simulink model "abslut50_fixpt20_32"  (R2021b)
settings: Solver=VariableStepAuto  StartTime=0.0  StopTime=99  RelTol=1e-3
undefined symbols (not defined in the file or in its folder): figd2104, xcu250
libraries: hdlBasic x5226, vmcUtilities x1
(part 14 of 17)

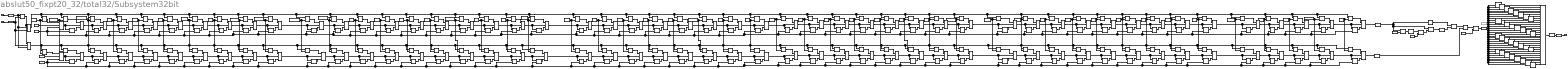
== system abslut50_fixpt20_32/total32/Subsystem32bit ==
  note: 50
  note: 40
  note: 30
  note: 20
  note: 10
  note: tiisai
  note: ooki
  note: 1275no11bit
  note: tmp_2
  note: tmp_3
  note: truthtable_out_x
  note: truthtable_out_y
  In3 : Inport
  In4 : Inport  Port=2
  CMult1 : hdlBasic/CMult  const=50  gui_display_data_type=Fixed-point  const_n_bits=6  const_bin_pt=0  float_type=Single  exp_bits=8  fraction_bits=24  en=off  latency=0  precision=Full  arith_type="Signed  (2's comp)"  n_bits=16  bin_pt=14  quantization=Truncate  overflow=Wrap  use_behavioral_HDL=off  mem_type=Distributed RAM  pipeline=off  XmcBlockStatus=1  maskContainerNames=tabcontainer1  block_type=cmult  block_config=sysgen:CMult_config
      settings: infoedit=[]
  Concat : hdlBasic/Concat  num_inputs=32  XmcBlockStatus=1  maskContainerNames=group1  block_type=concat  block_config=sysgen:Concat_config
  Constant : hdlBasic/Constant  const=1.0  gui_display_data_type=Fixed-point  arith_type=Unsigned  n_bits=1  bin_pt=0  preci_type=Single  exp_width=8  frac_width=24  explicit_period=on  period=1  XmcBlockStatus=1  maskContainerNames=tabcontainer1  block_type=constant  block_config=sysgen:Constant_config
  Constant1 : hdlBasic/Constant  const=0  gui_display_data_type=Fixed-point  arith_type=Unsigned  n_bits=6  bin_pt=0  preci_type=Single  exp_width=8  frac_width=24  explicit_period=on  period=1  XmcBlockStatus=1  maskContainerNames=tabcontainer1  block_type=constant  block_config=sysgen:Constant_config
  Constant2 : hdlBasic/Constant  const=1  gui_display_data_type=Fixed-point  arith_type=Unsigned  n_bits=6  bin_pt=0  preci_type=Single  exp_width=8  frac_width=24  explicit_period=on  period=1  XmcBlockStatus=1  maskContainerNames=tabcontainer1  block_type=constant  block_config=sysgen:Constant_config
  Constant3 : hdlBasic/Constant  const=98  gui_display_data_type=Fixed-point  arith_type=Unsigned  n_bits=7  bin_pt=0  preci_type=Single  exp_width=8  frac_width=24  explicit_period=on  period=1  XmcBlockStatus=1  maskContainerNames=tabcontainer1  block_type=constant  block_config=sysgen:Constant_config
  Constant5 : hdlBasic/Constant  const=1.0  gui_display_data_type=Fixed-point  arith_type=Unsigned  n_bits=10  bin_pt=0  preci_type=Single  exp_width=8  frac_width=24  explicit_period=on  period=1  XmcBlockStatus=1  maskContainerNames=tabcontainer1  block_type=constant  block_config=sysgen:Constant_config
  Constant6 : hdlBasic/Constant  const=0  gui_display_data_type=Fixed-point  arith_type=Unsigned  n_bits=6  bin_pt=0  preci_type=Single  exp_width=8  frac_width=24  explicit_period=on  period=1  XmcBlockStatus=1  maskContainerNames=tabcontainer1  block_type=constant  block_config=sysgen:Constant_config
  Constant7 : hdlBasic/Constant  const=1  gui_display_data_type=Fixed-point  arith_type=Unsigned  n_bits=6  bin_pt=0  preci_type=Single  exp_width=8  frac_width=24  explicit_period=on  period=1  XmcBlockStatus=1  maskContainerNames=tabcontainer1  block_type=constant  block_config=sysgen:Constant_config
  Convert23 : hdlBasic/Convert  Commented=on  gui_display_data_type=Fixed-point  arith_type=Unsigned  n_bits=11  bin_pt=0  float_type=Single  exp_bits=8  fraction_bits=24  quantization="Round  (unbiased: +/- Inf)"  overflow=Saturate  en=off  latency=1  pipeline=off  XmcBlockStatus=1  maskContainerNames=group2  block_type=convert  block_config=sysgen:Convert_config
  Gate_In1 : hdlBasic/Gateway In  gui_display_data_type=Fixed-point  arith_type=Signed (2's comp)  n_bits=32  bin_pt=30  preci_type=Double  exp_width=8  frac_width=24  rows=1  columns=1  quantization="Round  (unbiased: +/- Inf)"  overflow=Saturate  period=1  UseAsADC=off  ADCChannel='1'  interface=None  automatic_assignment=on  address_offset=hex2dec('00')  intf_name=''  intf_description=''  default_value=0  timing_constraint=None  locs_specified=off  LOCs={}  io_standard={}  inherit_from_input=off  hdl_port=on  XmcBlockStatus=1  maskContainerNames=group4  block_type=gatewayin  block_config=sysgen:gateway_in_config  block_width_w=590  block_height_w=620  block_width=640  block_height=850
  Gate_In2 : hdlBasic/Gateway In  gui_display_data_type=Fixed-point  arith_type=Signed (2's comp)  n_bits=32  bin_pt=30  preci_type=Double  exp_width=8  frac_width=24  rows=1  columns=1  quantization="Round  (unbiased: +/- Inf)"  overflow=Saturate  period=1  UseAsADC=off  ADCChannel='1'  interface=None  automatic_assignment=on  address_offset=hex2dec('00')  intf_name=''  intf_description=''  default_value=0  timing_constraint=None  locs_specified=off  LOCs={}  io_standard={}  inherit_from_input=off  hdl_port=on  XmcBlockStatus=1  maskContainerNames=group4  block_type=gatewayin  block_config=sysgen:gateway_in_config  block_width_w=590  block_height_w=620  block_width=640  block_height=850
  Gate_out1 : hdlBasic/Gateway Out  inherit_from_input=off  hdl_port=on  rows=1  columns=1  UseAsDAC=off  DACChannel='1'  interface=None  automatic_assignment=on  address_offset=hex2dec('00')  intf_name=''  intf_description=''  timing_constraint=None  locs_specified=off  LOCs={}  io_standard={}  XmcBlockStatus=1  maskContainerNames=group4  block_type=gatewayout  block_config=sysgen:gateway_out_config  block_width_w=590  block_height_w=620  block_width=620  block_height=750
  Negate : hdlBasic/Negate  precision=Full  arith_type=Unsigned  n_bits=16  bin_pt=14  quantization=Truncate  overflow=Wrap  en=off  latency=0  XmcBlockStatus=1  maskContainerNames=tabcontainer1  block_type=negate  block_config=sysgen:Negate_config
  ROM1 : hdlBasic/ROM  depth=1275  initVector=[1,1,1,1,1,1,1,1,1,1,1,1,1,1,1,1,1,1,1,1,1,1,1,1,1,1,1,1,1,1,1,1,1,1,1,1,1,1,1,1,1,1,1,0,0,1,1,1,1,1,1,0,0,0,0,1,1,1,1,1,0,0,0,0,0,0,1,1,1,1,1,0,0,0,0,0,0,0,1,1,1,1,0,0,0,0,0,0,0,0,0,1,1,1,0,0,0,0,0,0,0,0,0,0,0,1,1,1,0,0,0,0,0,0,0,0,0,0,0,0,1,1,0,0,0,0,0,0,0,0,0,0,0,0,0,0,1,1,0,0,0,0,0,0,0,0,0,0,0,0,0,0,0,1,1,0,0,0,0,0,0,0,0,0,0,0,0,0,0,0,0,1,0,0,0,0,0,0,0,0,0,0,0,0,0,0,0,0,0,0,1,0,0,0,0,0,0,0,0,0,0,0,0,0,0,0,0,0,0,0,1,0,0,0,0,0,0,0,0,0,0,0,0,0,0,0,0,0,0,0,0,1,0,0,0,0,0,0,0,0,0,0,0,0,0,0,0,0,0,0,0,0,0,1,0,0,0,0,0,0,0,0,0,0,0,0,0,0,0,0,0,0,0,0,0,0,1,0,0,0,0,0,0,0,0,0,0,0,0,0,0,0,0,0,0,0,0,0,0,0,1,0,0,0,0,0,0,0,0,0,0,0,0,0,0,0,0,0,0,0,0,0,0,0,0,1,0,0,0,0,0,0,0,0,0,0,0,0,0,0,0,0,0,0,0,0,0,0,0,0,0,1,0,0,0,0,0,0,0,0,0,0,0,0,0,0,0,0,0,0,0,0,0,0,0,0,0,0,1,0,0,0,0,0,0,0,0,0,0,0,0,0,0,0,0,0,0,0,0,0,0,0,0,0,0,0,1,0,0,0,0,0,0,0,0,0,0,0,0,0,0,0,0,0,0,0,0,0,0,0,0,0,0,0,0,1,0,0,0,0,0,0,0,0,0,0,0,0,0,0,0,0,0,0,0,0,0,0,0,0,0,0,0,0,0,1,0,0,0,0,0,0,0,0,0,0,0,0,0,0,0,0,0,0,0,0,0,0,0,0,0,0,0,0,0,0,1,0,0,0,0,0,0,0,0,0,0,0,0,0,0,0,0,0,0,0,0,0,0,0,0,0,0,0,0,0,0,0,1,1,0,0,0,0,0,0,0,0,0,0,0,0,0,0,0,0,0,0,0,0,0,0,0,0,0,0,0,0,0,0,0,1,1,0,0,0,0,0,0,0,0,0,0,0,0,0,0,0,0,0,0,0,0,0,0,0,0,0,0,0,0,0,0,0,0,1,1,0,0,0,0,0,0,0,0,0,0,0,0,0,0,0,0,0,0,0,0,0,0,0,0,0,0,0,0,0,0,0,0,0,1,1,1,0,0,0,0,0,0,0,0,0,0,0,0,0,0,0,0,0,0,0,0,0,0,0,0,0,0,0,0,0,0,0,0,0,1,1,1,0,0,0,0,0,0,0,0,0,0,0,0,0,0,0,0,0,0,0,0,0,0,0,0,0,0,0,0,0,0,0,0,0,0,1,1,1,1,0,0,0,0,0,0,0,0,0,0,0,0,0,0,0,0,0,0,0,0,0,0,0,0,0,0,0,0,0,0,0,0,0,0,1,1,1,1,1,0,0,0,0,0,0,0,0,0,0,0,0,0,0,0,0,0,0,0,0,0,0,0,0,0,0,0,0,0,0,0,0,0,0,1,1,1,1,1,0,0,0,0,0,0,0,0,0,0,0,0,0,0,0,0,0,0,0,0,0,0,0,0,0,0,0,0,0,0,0,0,0,0,0,1,1,1,1,1,1,0,0,0,0,0,0,0,0,0,0,0,0,0,0,0,0,0,0,0,0,0,0,0,0,0,0,0,0,0,0,0,0,0,0,0,1,1,1,1,1,1,1,0,0,0,0,0,0,0,0,0,0,0,0,0,0,0,0,0,0,0,0,0,0,0,0,0,0,0,0,0,0,0,0,0,0,0,1,1,1,1,1,1,1,1,0,0,0,0,0,0,0,0,0,0,0,0,0,0,0,0,0,0,0,0,0,0,0,0,0,0,0,0,0,0,0,0,0,0,1,1,1,1,1,1,1,1,1,1,0,0,0,0,0,0,0,0,0,0,0,0,0,0,0,0,0,0,0,0,0,0,0,0,0,0,0,0,0,0,0,0,1,1,1,1,1,1,1,1,1,1,1,1,1,0,0,0,0,0,0,0,0,0,0,0,0,0,0,0,0,0,0,0,0,0,0,0,0,0,0,0,0,0,0,1,1,1,1,1,1,1,1,1,1,1,1,1,1,1,1,1,0,0,0,0,0,0,0,0,0,0,0,0,0,0,0,0,0,0,0,0,0,0,0,0,0,0,1,1,1,1,1,1,1,1,1,1,1,1,1,1,1,1,1,1,1,1,1,0,0,0,0,0,0,0,0,0,0,0,0,0,0,0,0,0,0,0,0,0,0,0,0,1,1,1,1,1,1,1,1,1,1,1,1,1,1,1,1,1,1,1,1,1,1,1,1,1,0,0,0,0,0,0,0,0,0,0,0,0,0,0,0,0,0,0,0,0,1,1,1,1,1,1,1,1,1,1,1,1,1,1,1,1,1,1,1,1,1,1,1,1,1,1,1,1,1,1,1,0,0,0,0,0,0,0,0,0,0,0,0,0,0,1,1,1,1,1,1,1,1,1,1,1,1,1,1,1,1,1,1,1,1,1,1,1,1,1,1,1,1,1,1,1,1,1,1,1,1,1,1,1,1,1,1,1,1,1,1,1,1,1,1,1,1,1,1,1,1,1,1,1,1,1,1,1,1,1,1,1]  distributed_mem=Distributed memory  rst=off  init_reg=0  en=off  latency=0  gui_display_data_type=Boolean  arith_type=Boolean  n_bits=2  bin_pt=0  preci_type=Double  exp_width=8  frac_width=24  optimize=Area  use_rpm=on  simulation_type=fast_sim  XmcBlockStatus=1  maskContainerNames=tabcontainer1  block_type=sprom  block_config=sysgen:SPROM_config
  ROM10 : hdlBasic/ROM  depth=1275  initVector=[0,1,0,1,1,0,1,1,0,1,1,1,0,0,1,0,0,0,0,1,0,1,1,0,0,1,1,0,1,0,1,1,1,1,0,1,1,0,1,0,1,1,0,0,1,1,0,0,1,1,0,0,0,1,0,0,1,1,1,0,1,1,0,1,1,0,0,0,0,0,0,1,0,1,1,1,0,0,0,0,1,1,1,0,0,1,0,0,0,0,1,1,0,0,1,1,1,1,1,0,1,0,0,0,1,1,1,0,0,1,0,0,0,0,1,0,1,1,1,0,1,1,0,1,0,1,0,0,1,1,0,0,0,1,1,0,1,0,0,1,1,0,1,0,1,1,1,1,1,0,0,0,1,1,1,1,1,0,0,1,1,0,1,1,0,0,0,1,0,0,1,1,1,1,1,1,1,1,0,0,1,0,1,0,0,0,0,1,1,0,0,0,0,1,1,1,1,1,1,1,0,0,1,0,1,1,1,0,1,0,0,0,1,1,0,0,1,1,1,1,1,1,1,0,0,1,0,0,1,0,0,1,0,1,1,0,0,1,0,0,0,1,1,1,1,1,1,0,0,0,0,1,1,0,1,1,0,1,0,0,1,0,0,1,0,0,1,1,1,1,1,1,0,1,1,1,0,0,1,0,1,0,1,1,0,1,0,1,1,0,1,0,0,1,1,1,1,1,0,0,0,1,0,1,0,1,0,1,0,0,1,0,1,0,1,0,1,1,0,1,0,1,1,1,0,0,1,0,1,0,1,0,1,0,0,1,0,1,0,1,0,1,1,0,1,0,1,1,1,0,0,0,0,1,0,1,0,1,1,0,1,0,1,1,0,1,0,0,1,1,1,1,1,0,0,1,1,0,0,1,1,0,1,0,0,1,0,0,1,0,0,1,1,1,1,1,1,0,1,1,1,0,1,1,0,1,1,0,1,1,0,0,1,0,0,0,1,1,1,1,1,1,0,0,0,0,1,1,1,1,1,1,1,1,1,0,0,1,1,0,0,1,1,1,1,1,1,1,0,0,1,0,0,1,0,0,1,1,1,0,0,1,1,1,0,0,0,0,1,1,1,1,1,1,1,0,0,1,0,1,1,1,0,1,0,0,0,0,1,1,1,1,0,0,0,0,1,1,1,1,1,1,1,0,0,1,0,1,0,0,0,0,1,1,0,1,1,0,1,1,0,0,1,1,0,1,1,0,1,1,1,1,0,0,1,1,0,1,1,0,0,0,1,0,0,1,1,0,0,0,1,1,1,1,1,1,0,0,0,1,1,1,0,0,1,1,0,1,0,1,1,1,1,1,0,0,0,1,0,1,1,0,0,1,0,1,1,0,1,0,0,1,1,0,1,1,1,0,1,0,1,0,0,1,1,0,0,0,1,1,0,0,0,0,1,1,1,1,0,0,0,0,1,1,1,1,0,0,0,0,1,1,0,0,1,0,0,0,0,1,0,1,1,1,0,1,0,1,0,1,0,1,1,1,1,1,1,1,1,0,1,0,1,0,1,0,1,0,0,1,1,1,1,1,0,1,0,0,0,1,1,1,0,0,0,0,0,1,1,0,0,0,0,1,1,0,0,0,0,0,1,1,1,0,0,1,1,1,0,0,1,0,0,0,0,1,0,1,0,1,0,0,1,1,1,0,1,1,1,1,0,1,1,1,0,0,1,0,1,0,1,0,0,0,0,0,1,0,1,1,1,0,0,0,0,1,0,1,0,1,0,1,1,0,1,0,0,1,0,1,1,0,1,0,1,0,1,0,0,0,0,1,1,1,0,1,1,0,1,1,0,0,0,0,0,0,1,1,0,0,1,1,1,0,1,1,0,1,1,1,0,0,1,1,0,0,0,0,0,0,1,0,0,1,1,0,0,0,1,0,1,1,0,1,1,1,1,1,1,1,1,0,0,1,0,0,1,0,0,1,1,1,1,1,1,1,1,0,1,1,0,1,0,1,0,1,1,0,0,1,1,1,1,0,0,0,1,1,0,0,1,1,0,0,0,0,0,0,0,0,1,1,0,0,1,1,0,0,0,1,1,1,1,1,0,1,1,1,1,0,1,0,0,0,1,1,1,0,0,0,1,0,1,1,0,1,1,1,1,1,1,0,1,1,0,1,0,0,0,1,1,1,0,0,0,1,1,1,0,0,1,1,0,0,0,0,1,0,0,1,0,0,1,1,1,1,1,1,0,1,0,0,1,0,1,1,1,1,1,1,0,0,1,0,0,1,0,0,0,0,0,0,0,0,1,0,1,1,1,0,1,1,0,1,0,1,0,0,1,1,0,0,0,0,1,1,0,0,0,0,1,1,0,0,1,0,1,0,1,1,0,1,1,1,0,1,1,0,0,1,1,1,1,1,1,0,0,1,1,1,0,1,0,1,1,0,0,1,1,0,0,1,1,0,0,1,1,0,1,0,1,1,1,0,0,1,1,1,1,1,1,1,1,0,1,0,0,0,1,0,1,1,0,1,1,0,1,1,1,1,1,1,1,0,0,1,1,0,0,1,1,1,1,1,1,1,0,1,1,0,1,1,0,1,0,0,0,1,1,1,0,0,0,0,0,1,1,0,1,0,1,0,0,0,0,1,1,0,1,1,1,1,0,0,1,1,1,1,0,1,1,0,0,0,0,1,0,1,0,1,1,0,0,0,0,0,1,0,1,1,1,0,1,0,0,0,1,0,0,0,1,1,0,1,1,0,0,0,1,0,1,1,0,1,0,0,0,1,1,0,1,1,0,0,0,1,0,0,0,1,0,1,1,1,0,0,1,1,1,1,0,1,1,1,1,0,0,0,1,1,1,1,1,1,0,0,1,0,0,0,0,0,0,1,0,0,1,1,1,1,1,1,0,0,0,1,1,1,1,0,1,1,1,1,0]  distributed_mem=Distributed memory  rst=off  init_reg=0  en=off  latency=0  gui_display_data_type=Boolean  arith_type=Boolean  n_bits=2  bin_pt=0  preci_type=Double  exp_width=8  frac_width=24  optimize=Area  use_rpm=on  simulation_type=fast_sim  XmcBlockStatus=1  maskContainerNames=tabcontainer1  block_type=sprom  block_config=sysgen:SPROM_config
  ROM11 : hdlBasic/ROM  depth=1275  initVector=[0,0,1,0,1,1,0,1,0,0,1,1,0,1,1,0,0,0,1,0,0,1,0,1,1,0,1,1,0,0,1,0,0,1,0,0,0,0,0,0,1,1,0,1,1,1,0,1,1,0,1,0,1,0,0,1,0,0,1,1,1,0,1,0,1,1,1,0,0,1,1,1,1,1,1,1,0,1,1,0,1,1,1,0,1,0,1,0,0,0,0,1,1,0,1,0,0,0,1,0,0,1,1,1,1,0,1,1,0,0,1,1,0,1,0,0,0,0,0,0,0,1,0,0,0,0,1,0,1,1,0,1,0,1,1,1,1,0,1,0,1,1,0,1,1,0,0,0,1,1,0,0,0,0,1,1,1,0,1,0,1,1,1,0,1,1,1,1,1,1,1,1,1,0,0,0,1,1,0,1,0,0,0,0,0,0,1,1,0,0,1,0,0,1,1,0,0,0,0,1,0,1,0,0,1,0,1,0,1,1,1,0,1,0,1,0,1,1,0,0,0,0,1,0,1,1,1,1,0,1,1,0,1,1,0,1,0,0,1,0,0,1,0,0,0,0,1,0,1,0,0,0,0,1,1,0,0,1,1,0,0,1,0,0,1,0,1,1,0,0,0,1,0,1,1,1,1,0,0,0,1,1,1,0,0,0,1,1,0,0,1,1,0,1,0,0,0,1,1,0,0,0,0,0,1,1,1,1,1,0,0,0,0,1,1,1,1,0,0,0,1,1,0,0,1,0,0,0,0,1,1,1,1,1,0,0,0,0,1,1,1,1,0,0,0,1,1,0,0,1,1,1,0,0,0,1,1,1,0,0,0,1,1,0,0,1,1,0,1,0,0,0,1,1,0,0,0,0,1,1,0,0,1,1,0,0,1,0,0,1,0,1,1,0,0,0,1,0,1,1,1,1,0,0,1,1,0,1,1,0,1,0,0,1,0,0,1,0,0,0,0,1,0,1,0,0,0,0,1,1,1,1,1,1,0,1,0,1,0,1,0,1,1,0,0,0,0,1,0,1,1,1,1,0,1,1,0,1,0,1,1,0,1,0,1,1,0,0,1,1,0,0,0,0,1,0,1,0,0,1,0,1,0,1,1,1,0,0,0,0,0,0,0,0,1,1,1,1,0,0,0,1,1,0,1,0,0,0,0,0,0,1,1,0,0,1,0,0,1,0,0,0,0,1,0,0,1,0,0,1,1,1,0,1,0,1,1,1,0,1,1,1,1,1,1,1,0,0,1,1,0,1,0,0,1,0,1,1,0,0,1,1,0,1,0,1,1,0,1,1,0,0,0,1,1,0,0,0,1,1,1,1,0,0,0,1,1,0,0,0,1,1,1,1,0,0,1,0,0,0,0,1,0,1,1,0,1,0,1,1,1,0,1,1,0,1,1,0,1,1,1,1,0,1,1,0,1,1,0,1,0,1,1,0,0,1,1,0,1,0,0,0,0,0,0,1,0,1,0,1,1,0,1,1,1,1,1,1,0,1,1,0,1,0,1,0,1,1,0,1,0,0,0,1,0,0,1,1,1,1,0,1,1,1,0,0,0,0,1,0,1,1,0,1,0,0,0,0,1,1,1,0,1,1,0,1,1,1,0,1,0,1,0,0,0,0,1,0,0,1,1,0,0,1,0,0,0,0,0,0,0,0,1,0,0,1,1,0,0,1,0,1,0,0,1,1,1,1,1,1,1,0,1,0,1,0,1,0,1,0,1,0,0,1,1,0,0,1,1,0,0,1,0,1,0,1,0,1,0,1,1,0,0,1,1,1,0,1,0,1,1,0,0,1,0,0,0,0,0,0,0,1,0,1,0,0,1,0,1,0,0,0,0,0,0,0,1,0,0,1,1,0,1,1,0,1,0,1,0,0,1,1,0,0,0,1,0,1,0,1,0,0,0,0,0,0,0,0,0,0,1,0,1,0,1,0,0,0,1,1,0,0,0,0,0,1,1,0,1,1,0,0,1,1,0,1,1,1,1,1,0,0,0,1,0,1,1,0,1,0,0,0,1,1,1,1,1,0,1,1,0,0,1,0,0,1,0,0,1,0,0,1,1,1,1,0,1,0,0,1,1,0,0,1,1,0,0,1,1,0,0,1,1,0,0,1,1,0,0,1,0,1,1,1,1,0,1,0,1,1,0,1,1,0,0,0,0,1,1,0,1,1,0,0,1,0,1,0,0,1,1,1,1,0,0,1,0,1,0,0,1,1,0,1,1,0,0,0,0,1,0,0,0,1,0,0,1,1,1,1,1,1,0,0,1,0,1,1,1,0,0,0,1,1,1,1,1,1,0,0,0,1,1,1,0,1,0,0,1,1,1,1,1,1,0,1,1,0,1,1,0,0,0,1,0,1,1,1,0,0,0,1,0,0,1,1,1,1,1,1,1,1,1,1,1,1,0,0,1,0,0,0,1,1,1,0,1,0,0,0,1,0,1,0,0,1,1,1,0,0,1,1,1,1,1,0,0,0,1,0,1,0,0,0,0,0,0,0,0,0,0,1,0,1,0,0,0,1,1,1,1,1,0,0,1,1,1,0,0,1,1,0,0,0,1,1,0,1,0,0,1,0,1,0,1,1,0,0,1,1,0,0,0,0,0,0,1,1,0,0,1,1,0,1,0,1,0,0,1,0,1,1,0,0,0,1,0,1,1,1,1,0,0,0,0,0,0,0,0,1,1,1,0,1,1,0,0,1,1,0,0,0,0,1,1,0,0,1,1,0,1,1,1,0,0,0,0,0,0,0,0,1,1,1,1,0,0,0,0,1,0,1,0,0,1,1,1,1,1,0,0,1,0,1,1,1,0,1,1,0,0,1,1,0,1,1,1,0,1,0,0,1,1,1,1,1,0,0,1,0,1,0,0,0,0]  distributed_mem=Distributed memory  rst=off  init_reg=0  en=off  latency=0  gui_display_data_type=Boolean  arith_type=Boolean  n_bits=2  bin_pt=0  preci_type=Double  exp_width=8  frac_width=24  optimize=Area  use_rpm=on  simulation_type=fast_sim  XmcBlockStatus=1  maskContainerNames=tabcontainer1  block_type=sprom  block_config=sysgen:SPROM_config
  ROM12 : hdlBasic/ROM  depth=1275  initVector=[0,1,0,0,1,1,0,0,1,1,0,0,0,1,1,1,0,0,0,1,1,0,0,0,0,0,0,1,0,1,0,1,1,0,0,0,1,0,0,1,1,1,0,0,0,1,1,1,1,0,0,1,0,0,0,1,0,1,1,0,1,0,1,0,0,0,0,1,1,0,1,0,0,1,0,0,0,1,1,1,1,0,1,0,0,1,0,0,0,1,1,0,1,0,0,0,0,0,0,1,1,1,0,1,1,0,1,1,0,1,1,0,1,0,0,0,1,0,1,1,0,0,1,0,0,1,0,0,1,1,1,1,0,0,1,1,1,0,0,0,1,0,1,0,1,1,0,1,1,1,1,1,0,1,0,0,1,0,0,0,1,1,1,0,0,0,1,0,1,1,0,0,0,1,1,1,0,1,0,0,0,0,0,1,0,0,0,0,1,0,0,1,0,1,0,1,1,1,1,0,0,0,1,1,0,1,0,1,1,0,0,0,0,0,0,0,1,0,1,1,1,1,0,0,0,0,1,1,0,0,1,0,0,1,0,0,0,1,1,1,0,0,1,1,0,1,0,0,1,1,0,0,1,0,1,0,1,0,1,0,1,1,0,1,1,1,1,0,1,0,0,0,1,0,1,1,1,0,0,1,0,0,1,0,0,1,0,1,0,1,0,1,1,1,1,0,0,0,1,1,0,0,1,1,0,0,1,1,1,0,0,1,1,0,0,1,1,0,0,1,0,1,1,0,1,0,0,1,1,0,0,1,1,1,0,0,1,1,0,0,1,1,0,0,1,0,1,1,0,1,1,1,0,0,1,0,0,1,0,0,1,0,1,0,1,0,1,1,1,1,0,0,0,1,1,0,0,1,0,1,0,1,0,1,0,1,1,0,1,1,1,1,0,1,0,0,0,1,0,1,1,1,1,1,1,1,0,0,1,0,0,0,1,1,1,0,0,1,1,0,1,0,0,1,1,0,0,1,1,0,1,1,0,1,1,0,0,0,0,0,0,1,0,1,1,1,1,0,0,0,0,1,1,0,0,1,0,0,0,0,0,0,0,0,1,0,1,0,1,0,1,1,1,1,0,0,0,1,1,0,1,0,1,1,0,0,0,1,0,1,1,0,1,0,0,0,0,0,1,1,1,0,1,0,0,0,0,0,1,0,0,0,0,1,0,1,0,1,0,1,0,0,1,0,1,0,1,0,1,0,0,1,0,0,0,1,1,1,0,0,0,1,0,1,1,0,1,1,1,1,0,1,0,0,1,0,1,1,1,1,0,1,0,0,0,1,0,1,0,1,1,0,1,1,1,1,1,0,1,0,0,1,0,0,1,1,1,1,0,0,1,0,0,1,0,0,0,1,0,0,1,0,0,1,1,1,1,0,0,1,1,1,1,0,1,0,0,1,1,1,1,1,1,0,0,1,0,1,1,1,0,1,1,0,1,1,0,1,0,0,0,1,0,1,1,1,1,0,0,0,0,1,0,0,0,0,0,0,1,0,0,0,0,1,1,1,0,1,0,0,0,0,0,0,1,1,1,0,1,1,1,0,1,1,0,1,0,0,1,1,0,0,1,1,0,0,1,0,1,1,0,1,1,1,1,1,0,1,0,0,1,0,0,0,1,1,1,0,0,1,0,1,1,0,1,1,0,1,1,0,1,1,0,1,1,0,1,0,0,1,1,0,1,1,0,1,0,0,1,0,0,0,1,1,0,1,1,1,0,0,0,1,1,1,1,1,1,1,1,1,1,0,0,0,1,1,1,0,1,1,1,0,1,1,0,1,0,1,0,0,0,0,0,1,0,1,0,0,0,0,1,0,1,0,0,0,0,1,0,1,0,0,0,0,1,0,1,0,0,0,1,1,1,1,0,0,1,0,0,0,0,0,0,1,0,1,1,1,0,0,1,0,0,1,0,0,1,0,0,1,0,0,1,1,1,0,1,0,0,0,0,1,0,0,1,1,1,0,0,0,0,0,0,0,1,0,1,1,1,0,1,1,1,1,0,1,1,0,1,1,1,1,0,1,1,1,0,1,0,0,0,0,0,0,1,0,1,1,0,0,0,0,0,1,1,1,0,1,0,0,1,0,1,0,1,1,0,1,1,0,1,1,0,1,0,1,0,0,1,0,1,1,1,0,0,0,0,0,0,0,0,0,1,0,0,1,0,0,0,0,0,0,1,0,1,1,1,1,0,1,1,1,1,0,1,1,1,1,0,1,0,0,0,0,0,0,1,0,0,1,1,0,0,0,1,1,0,0,1,0,1,0,0,0,1,1,0,0,0,1,0,0,1,0,0,0,0,1,0,0,1,0,0,0,1,1,0,0,0,1,0,1,0,0,1,0,0,0,1,1,1,0,1,1,0,0,1,1,0,1,0,1,0,1,0,0,0,0,0,0,0,0,0,0,0,0,1,0,1,0,1,0,1,1,0,0,1,1,0,1,1,0,0,1,1,1,0,0,1,1,1,1,0,0,0,0,0,0,1,1,1,0,0,1,1,1,1,1,1,0,0,1,1,1,0,0,0,0,0,0,1,1,1,1,0,0,1,1,0,1,1,1,0,0,0,0,0,1,1,1,1,0,1,1,0,0,1,0,0,1,0,0,1,1,0,0,1,0,0,1,0,0,1,1,0,1,1,1,1,0,0,0,0,0,1,1,1,0,1,0,0,0,0,1,0,1,0,1,1,1,1,0,0,0,0,1,0,0,1,0,0,0,0,1,0,0,1,0,0,0,0,1,1,1,1,0,1,0,1,0,0,0,0,1,0,0,1,0,0,0,1,0,0,1,1,1,0,1,0,0,0,1,1,0,0,0,0,0,1,0,0,1,0,0,0,0,0,1,1,0,0,0,1,0,1,1,1,0,0,1,0,0,0,1,0]  distributed_mem=Distributed memory  rst=off  init_reg=0  en=off  latency=0  gui_display_data_type=Boolean  arith_type=Boolean  n_bits=2  bin_pt=0  preci_type=Double  exp_width=8  frac_width=24  optimize=Area  use_rpm=on  simulation_type=fast_sim  XmcBlockStatus=1  maskContainerNames=tabcontainer1  block_type=sprom  block_config=sysgen:SPROM_config
  ROM13 : hdlBasic/ROM  depth=1275  initVector=[0,1,0,1,1,1,1,1,0,1,0,1,0,0,0,1,1,1,0,0,0,0,0,1,1,0,1,0,1,0,1,0,0,0,1,1,0,0,0,0,1,0,0,1,1,0,0,1,1,0,0,0,0,0,0,1,0,1,1,1,0,1,1,0,0,0,0,0,0,0,1,1,0,1,0,0,0,1,0,0,1,1,0,0,0,1,0,1,0,1,1,0,0,0,0,1,0,1,0,0,0,0,0,1,0,0,1,1,0,0,0,0,1,1,1,1,1,1,1,0,1,1,1,1,1,0,0,1,1,1,0,1,0,1,1,0,1,1,1,1,0,0,1,0,1,1,1,1,1,0,0,1,1,1,0,1,0,1,0,1,1,0,0,1,1,1,1,1,1,1,1,1,0,1,1,1,0,0,1,0,1,0,0,1,0,0,0,0,1,0,1,0,0,0,0,1,0,0,1,1,0,1,1,1,1,1,0,0,1,0,0,0,0,0,0,1,1,0,1,0,0,1,1,0,1,1,1,0,1,0,1,1,0,0,1,0,0,1,1,1,0,1,1,0,1,0,0,0,1,0,1,1,1,1,0,0,0,0,0,1,1,0,0,1,1,1,1,0,0,1,1,0,0,0,1,1,1,0,1,1,0,1,1,0,1,1,1,0,0,0,1,1,1,0,1,1,1,0,1,0,0,1,0,1,0,1,0,0,1,0,1,0,1,0,1,0,1,0,1,1,0,1,0,0,0,0,1,0,1,0,1,0,0,1,0,1,0,1,0,1,0,1,0,1,1,0,1,0,0,0,0,1,0,1,1,0,1,1,0,1,1,1,0,0,0,1,1,1,0,1,1,1,0,1,0,0,0,0,1,0,0,0,0,0,1,1,0,0,1,1,1,1,0,0,1,1,0,0,0,1,1,1,0,0,1,1,1,0,0,1,0,0,1,1,1,0,1,1,0,1,0,0,0,1,0,1,1,1,1,0,1,1,0,1,1,0,0,0,0,0,1,1,0,1,0,0,1,1,0,1,1,1,0,1,0,1,1,0,1,0,0,1,0,1,1,1,0,0,0,0,1,0,0,1,1,0,1,1,1,1,1,0,0,1,0,0,1,0,1,1,1,1,0,1,0,0,1,0,1,1,1,0,0,1,0,1,0,0,1,0,0,0,0,1,0,1,1,0,0,1,1,1,1,0,0,1,1,0,1,0,1,0,1,0,1,1,0,0,1,1,1,1,1,1,1,1,1,0,0,1,1,0,0,0,0,1,1,0,0,1,1,1,1,1,1,0,0,1,0,1,1,1,1,1,0,0,1,1,1,0,0,1,0,1,1,1,1,1,1,0,1,0,0,1,1,1,1,1,1,1,0,0,1,1,1,0,1,0,1,1,0,1,1,0,1,1,0,0,1,0,0,1,0,0,1,1,0,1,1,0,0,1,1,0,0,0,0,1,1,1,1,1,1,1,0,1,0,1,0,1,1,0,0,1,1,1,1,0,0,1,1,0,1,0,1,0,0,0,0,0,1,0,1,0,0,0,0,0,1,0,1,1,0,1,0,1,0,1,1,0,0,0,0,1,1,0,1,0,1,0,1,1,0,0,0,1,1,0,0,0,1,0,1,0,1,1,1,1,0,1,1,1,1,1,0,1,0,1,1,0,1,0,1,1,1,1,1,0,1,1,1,0,0,0,0,1,1,0,1,0,0,0,1,1,0,1,1,1,1,0,1,1,1,1,0,0,0,0,1,1,1,1,0,1,1,1,1,0,1,1,1,0,1,1,1,0,1,1,0,0,0,0,0,0,1,0,1,1,0,0,0,1,1,1,1,1,1,1,1,0,0,0,1,1,0,1,0,0,0,0,0,0,1,1,0,0,0,0,0,0,0,0,1,0,1,1,1,0,1,1,0,0,0,1,0,0,1,0,0,0,1,1,0,1,1,1,0,1,0,0,0,0,0,0,0,1,0,0,1,1,0,0,0,0,0,1,1,1,0,0,1,1,1,0,1,1,1,1,0,1,1,1,0,0,1,1,1,0,0,0,0,0,1,1,0,1,0,0,0,1,1,1,0,1,1,1,0,1,1,0,1,1,0,0,1,1,0,0,0,0,1,1,0,0,1,1,0,1,1,0,1,1,1,0,1,1,0,0,1,1,0,1,0,1,0,0,1,0,0,1,0,0,1,1,0,0,1,1,1,1,0,0,1,1,1,1,0,0,1,1,0,0,1,0,0,1,0,0,1,0,1,1,1,0,0,0,1,0,0,0,0,1,0,0,0,0,0,0,0,1,1,0,0,1,1,1,1,0,0,1,1,0,0,0,0,0,0,0,1,0,0,0,0,1,0,0,1,0,0,0,0,0,0,1,0,1,1,0,1,0,1,0,1,1,0,0,0,0,0,0,0,0,0,0,0,0,1,1,0,1,0,1,0,1,1,0,1,0,0,0,0,1,1,0,1,0,0,1,0,0,1,1,0,1,0,0,1,1,0,1,0,0,1,0,1,1,1,1,0,1,0,0,1,0,1,1,0,0,1,0,1,1,0,0,1,0,0,1,1,1,1,0,0,1,1,1,0,1,1,0,1,0,1,1,1,1,1,0,0,0,0,1,0,0,1,0,0,0,0,1,1,1,1,1,0,1,0,1,1,0,1,1,1,0,0,1,1,0,1,1,1,1,0,0,0,0,0,0,0,0,1,1,1,0,0,0,0,0,0,0,1,1,0,0,0,0,0,0,0,1,1,1,0,0,0,0,0,0,0,0,1,1,1,1,0,0,1,1,1,0,1,0,1,0,0,1,0,0,0,0,1,1,1,1,1,0,1,1,1,0,0,1,1,1,0,1,1,1,1,1,0,0,0,0,1,0,0,1,0,1,0,1,1,1,0]  distributed_mem=Distributed memory  rst=off  init_reg=0  en=off  latency=0  gui_display_data_type=Boolean  arith_type=Boolean  n_bits=2  bin_pt=0  preci_type=Double  exp_width=8  frac_width=24  optimize=Area  use_rpm=on  simulation_type=fast_sim  XmcBlockStatus=1  maskContainerNames=tabcontainer1  block_type=sprom  block_config=sysgen:SPROM_config
  ROM14 : hdlBasic/ROM  depth=1275  initVector=[1,1,0,0,0,1,1,0,1,0,1,1,1,1,1,0,0,1,1,0,0,1,0,1,1,1,1,0,1,1,0,1,0,0,0,1,0,1,1,1,1,1,0,0,0,1,0,1,0,1,1,1,0,1,1,1,1,0,1,1,1,1,1,0,0,0,1,1,1,0,1,0,1,0,0,0,0,1,0,0,0,1,0,0,1,0,1,0,1,1,0,1,0,0,0,1,1,1,1,0,1,0,1,1,1,0,0,0,0,1,1,0,1,1,1,0,0,0,0,1,0,1,0,1,0,0,1,0,0,0,0,1,1,1,0,0,1,1,0,0,0,0,1,1,0,0,1,0,0,1,1,0,1,1,0,0,1,0,1,0,0,0,1,0,1,0,0,0,1,0,0,1,0,0,0,0,0,0,0,1,1,1,1,0,0,1,0,1,0,1,1,1,0,0,0,0,1,1,1,1,1,0,0,0,1,0,1,1,1,0,1,0,0,0,1,1,0,1,0,0,0,0,0,1,1,0,1,0,1,0,1,1,0,1,1,1,0,1,1,1,1,1,1,0,1,0,1,1,1,0,1,0,1,0,1,1,1,1,1,0,0,0,1,1,0,0,1,0,0,0,1,0,0,1,0,0,1,1,1,0,0,1,0,0,1,0,0,1,1,1,0,1,0,1,0,0,0,1,0,1,1,1,1,0,0,0,0,1,1,1,1,1,0,0,0,0,1,1,1,0,1,0,0,0,0,1,1,1,0,0,0,0,1,1,1,1,1,0,0,0,0,1,1,1,0,1,0,0,0,0,0,1,1,1,0,0,1,0,0,1,0,0,1,1,1,0,1,0,1,0,0,0,1,0,1,0,0,1,0,1,1,1,1,1,0,0,0,1,1,0,0,1,0,0,0,1,0,0,1,0,0,0,0,0,0,0,1,0,1,1,1,0,1,1,1,1,1,1,0,1,0,1,1,1,0,1,0,1,0,1,0,0,1,0,1,1,0,0,0,1,1,0,1,0,0,0,0,0,1,1,0,1,0,1,0,1,0,1,0,1,1,0,1,0,1,1,1,0,0,0,0,1,1,1,1,1,0,0,0,1,0,1,1,1,0,0,1,0,0,0,0,0,0,1,0,0,1,0,0,0,0,0,0,0,1,1,1,1,0,0,1,0,1,0,1,1,1,0,0,0,1,1,0,0,0,1,1,1,1,0,0,1,0,1,0,0,0,1,0,1,0,0,0,1,0,0,0,1,0,1,1,1,1,1,1,1,1,0,1,0,0,1,1,0,0,0,0,1,1,0,0,1,0,0,1,1,0,1,0,1,1,1,1,0,0,1,1,0,0,1,1,1,1,0,1,0,1,0,1,0,0,1,0,0,0,0,1,1,1,0,0,0,1,0,0,0,1,0,1,0,0,1,0,1,0,0,0,1,0,0,0,0,0,0,1,1,0,1,1,1,0,0,0,0,1,0,1,0,1,1,1,0,0,0,0,0,0,0,0,1,1,1,0,1,0,1,1,0,0,0,1,1,1,1,0,1,0,1,1,1,0,1,1,0,0,0,1,1,1,1,0,0,1,1,1,1,0,0,0,1,1,0,1,0,0,0,1,0,0,1,0,1,0,1,1,0,1,0,1,0,0,0,0,0,0,0,1,0,0,1,0,0,0,0,0,0,0,1,0,1,0,1,1,1,0,1,0,1,0,0,0,0,1,1,1,0,1,0,1,1,0,0,1,0,1,1,1,1,0,1,0,0,1,1,0,1,0,1,1,1,1,1,0,1,1,1,1,1,0,0,0,0,1,0,0,0,1,0,1,1,0,1,1,0,1,1,0,1,1,0,1,1,0,1,0,0,0,1,0,0,1,0,1,0,1,1,1,0,1,1,0,0,0,1,1,0,0,1,1,1,0,1,1,0,1,1,0,1,1,0,1,1,1,0,0,1,1,0,0,0,1,0,1,1,1,1,1,0,0,0,1,0,0,1,0,1,0,0,0,1,1,0,1,0,1,1,1,1,0,1,0,1,1,0,0,0,1,0,1,0,0,1,0,1,1,0,1,0,0,0,1,0,0,1,0,0,1,1,0,1,0,0,1,1,1,0,0,1,1,0,0,1,1,1,0,0,1,0,1,1,0,0,1,0,0,1,1,0,1,1,1,1,0,0,0,1,1,1,1,1,0,1,1,0,0,1,0,1,0,0,0,0,0,0,1,0,1,0,0,1,1,0,1,1,1,1,1,0,0,0,0,0,1,1,0,0,1,0,1,1,1,0,0,1,1,0,0,1,0,0,1,0,1,1,0,0,1,1,0,1,0,0,1,0,0,1,1,0,0,1,1,1,0,1,0,1,1,1,1,1,0,1,0,1,1,1,1,0,1,1,0,0,0,0,0,1,1,1,0,0,0,0,1,1,1,0,0,0,0,0,1,1,0,1,1,1,1,0,1,0,1,1,0,1,0,1,1,1,1,1,0,1,0,1,0,0,1,0,1,0,0,0,1,1,0,0,0,0,1,1,0,0,0,1,0,1,0,0,1,0,1,0,1,1,1,1,1,0,0,0,1,1,1,1,1,0,1,1,0,1,0,0,0,0,0,0,0,0,0,1,1,1,1,1,1,1,1,0,0,0,0,0,0,0,0,0,1,0,1,1,0,1,1,1,1,1,1,0,0,0,1,0,0,1,1,0,1,1,0,0,0,1,1,0,0,1,0,0,1,1,1,1,1,1,0,0,1,0,0,1,1,0,0,0,1,1,0,1,1,0,0,1,0,0,0,1,1,0,1,1,0,1,1,0,1,1,1,0,1,0,0,1,1,1,1,1,1,0,1,1,1,1,0,1,1,1,1,1,1,0,0,1,0,1,1,1,0,1,1,0,1,1,0,1,1]  distributed_mem=Distributed memory  rst=off  init_reg=0  en=off  latency=0  gui_display_data_type=Boolean  arith_type=Boolean  n_bits=2  bin_pt=0  preci_type=Double  exp_width=8  frac_width=24  optimize=Area  use_rpm=on  simulation_type=fast_sim  XmcBlockStatus=1  maskContainerNames=tabcontainer1  block_type=sprom  block_config=sysgen:SPROM_config
  ROM15 : hdlBasic/ROM  depth=1275  initVector=[0,0,0,0,1,1,0,0,1,1,0,0,1,0,1,0,1,1,0,0,1,0,0,1,1,0,1,0,0,0,1,0,0,1,1,0,1,0,0,1,0,0,1,0,0,1,1,1,0,0,0,1,1,1,0,0,0,0,0,1,0,0,0,1,1,1,0,1,1,1,0,0,1,0,0,1,0,1,1,0,0,1,0,1,0,1,0,0,0,1,1,1,0,1,1,0,1,1,1,1,0,0,1,0,1,1,0,0,0,0,0,1,1,0,1,0,1,0,1,0,0,0,0,0,1,1,1,0,0,1,0,1,1,1,1,0,0,1,0,0,0,1,0,0,0,1,1,0,0,1,0,0,0,0,0,0,1,1,1,1,0,0,1,0,1,0,1,1,0,0,1,0,1,1,0,1,1,0,0,1,1,0,1,1,1,0,1,1,1,1,1,1,1,0,1,1,0,1,0,0,0,0,0,0,0,0,0,1,0,1,0,0,0,1,1,1,0,1,1,1,0,0,0,0,1,1,1,1,0,0,1,0,0,1,1,1,0,1,0,1,0,1,0,0,0,1,0,1,0,0,1,0,0,1,1,1,0,0,1,0,1,0,1,1,1,0,0,1,1,1,0,1,0,0,0,0,0,1,1,0,1,0,0,1,1,1,0,1,1,1,1,1,0,0,1,0,0,0,1,0,1,0,0,1,1,0,0,1,1,0,0,0,1,1,1,1,0,0,1,1,1,0,0,1,0,1,0,0,1,1,0,0,1,1,0,0,0,1,1,1,1,0,0,1,1,1,0,0,1,0,0,0,1,1,0,1,0,0,1,1,1,0,1,1,1,1,1,0,0,1,0,0,0,1,0,1,1,0,1,1,1,0,0,1,0,1,0,1,1,1,0,0,1,1,1,0,1,0,0,0,0,1,0,0,1,0,0,0,1,1,1,0,1,0,1,0,1,0,0,0,1,0,1,0,0,1,0,0,0,0,0,0,0,0,0,0,0,0,1,1,1,0,1,1,1,0,0,0,0,1,1,1,1,0,0,1,0,0,0,1,1,0,0,0,1,1,1,1,0,1,1,0,1,0,0,0,0,0,0,0,0,0,1,0,1,0,1,0,0,1,1,0,0,1,0,1,0,1,1,0,1,1,0,0,1,1,0,1,1,1,0,1,1,1,1,0,0,0,1,1,1,1,1,1,0,0,0,1,0,0,0,1,1,1,1,0,0,1,0,1,0,1,1,0,0,1,1,1,1,0,0,0,0,0,0,0,0,1,1,1,1,0,1,0,0,0,1,0,0,0,1,1,0,0,1,0,0,0,0,1,0,1,1,1,0,0,0,0,1,1,1,0,1,0,0,0,0,0,0,1,1,1,0,0,1,0,1,1,1,1,0,0,0,1,0,1,0,1,1,1,1,1,1,0,1,0,1,0,0,0,1,0,0,0,0,0,1,1,0,1,0,1,0,1,0,1,0,1,0,0,1,1,1,1,1,1,1,1,1,1,0,0,1,0,1,0,1,0,1,1,0,1,1,1,1,0,0,1,0,1,1,1,1,1,1,0,0,0,0,1,1,1,1,0,0,0,0,1,1,1,1,1,1,1,0,0,1,0,1,0,1,0,0,0,1,1,0,0,1,0,0,1,0,0,0,0,1,1,1,1,0,0,0,0,1,0,0,1,0,0,1,0,1,1,1,0,0,1,0,0,1,0,1,1,1,1,1,0,1,1,0,0,0,1,1,0,0,1,1,0,0,0,1,1,0,1,1,1,1,1,0,0,0,0,1,0,0,0,1,1,1,0,0,0,0,0,1,0,0,0,0,1,1,0,0,0,0,1,1,0,0,0,0,1,0,0,0,0,0,1,1,1,1,0,0,0,1,1,1,0,1,1,0,0,1,1,1,1,1,0,1,0,1,1,0,0,1,1,0,1,0,1,1,1,1,1,0,0,1,1,0,1,0,0,1,0,0,1,0,0,1,1,0,0,1,0,0,0,0,1,0,1,1,0,1,1,1,1,0,1,1,0,1,0,0,0,0,1,0,0,1,1,0,0,0,1,0,0,1,1,0,0,1,0,0,1,1,1,0,0,0,0,1,1,0,1,1,1,1,1,1,0,1,1,0,0,0,0,1,1,1,0,0,1,0,0,0,0,1,1,0,1,0,1,1,1,0,1,0,1,1,1,0,1,0,0,0,1,0,0,0,0,0,0,1,0,0,0,1,0,1,1,1,0,1,0,1,1,1,0,0,1,1,0,0,1,1,1,0,0,0,0,1,1,0,1,1,1,1,1,1,0,1,0,0,0,0,1,0,1,1,1,1,1,1,0,1,1,0,0,0,0,1,1,1,0,0,1,0,1,0,0,0,0,0,1,0,0,0,0,1,0,1,1,1,1,1,0,1,1,1,1,0,1,1,1,1,1,0,1,0,0,0,0,1,0,0,0,0,0,1,0,0,1,1,0,0,1,0,1,0,0,1,1,1,0,0,0,1,0,0,1,1,0,0,1,1,0,0,1,1,0,0,1,0,0,0,1,1,1,0,0,1,0,1,0,0,1,0,1,1,1,1,1,1,1,0,1,0,1,0,1,0,0,0,0,1,1,0,1,1,1,0,0,1,1,1,0,1,1,0,0,0,0,1,0,1,0,1,0,1,1,1,1,1,1,0,0,1,0,0,1,0,0,0,1,0,1,0,0,0,0,1,0,1,1,0,0,1,1,0,0,1,1,0,0,1,1,0,1,0,0,0,0,1,0,1,0,0,0,1,0,0,1,0,0,0,0,0,0,0,0,0,1,1,0,0,1,1,1,0,0,0,0,1,0,0,1,0,1,1,0,1,0,0,1,0,0,0,0,1,1,1,0,0,1,1,0,0,0,0,0,0,0,0]  distributed_mem=Distributed memory  rst=off  init_reg=0  en=off  latency=0  gui_display_data_type=Boolean  arith_type=Boolean  n_bits=2  bin_pt=0  preci_type=Double  exp_width=8  frac_width=24  optimize=Area  use_rpm=on  simulation_type=fast_sim  XmcBlockStatus=1  maskContainerNames=tabcontainer1  block_type=sprom  block_config=sysgen:SPROM_config
  ROM16 : hdlBasic/ROM  depth=1275  initVector=[0,1,1,1,0,0,0,0,1,0,1,0,0,0,1,0,0,0,1,1,1,0,1,1,1,0,0,0,0,0,1,1,1,1,1,0,0,0,1,1,0,0,0,0,1,1,1,0,1,1,0,1,0,0,1,0,0,0,0,1,0,1,0,0,1,0,1,1,0,0,1,0,0,0,1,1,1,0,0,0,1,0,1,1,1,1,1,0,0,1,1,0,0,1,0,1,0,0,1,1,1,0,0,1,1,0,1,0,1,1,1,0,1,1,1,0,0,1,1,0,1,1,1,1,1,1,0,0,0,0,0,0,0,0,0,0,0,1,0,1,1,0,1,0,0,1,1,0,1,0,0,1,1,0,0,0,0,1,1,1,0,1,0,1,1,0,0,0,0,1,0,1,0,1,1,1,1,1,0,0,1,0,1,1,1,0,1,1,0,0,1,1,1,1,1,0,1,0,1,1,1,0,1,1,1,1,0,1,0,1,0,1,1,0,0,0,0,1,0,0,1,0,0,0,0,1,1,0,1,0,1,0,1,0,0,0,1,0,1,1,0,0,0,1,1,1,0,0,1,1,1,0,0,0,1,0,1,1,0,0,1,0,0,1,0,1,0,1,0,0,1,0,0,1,0,0,1,0,1,1,1,1,0,1,1,1,0,0,0,1,0,1,0,1,0,0,0,0,1,1,0,1,0,1,0,1,0,1,0,1,0,0,1,1,1,1,0,1,1,0,1,0,1,0,1,0,1,0,1,0,1,0,1,0,1,0,0,1,1,1,1,0,1,1,0,1,0,1,0,1,1,1,0,1,1,1,1,0,1,1,1,0,0,0,1,0,1,0,1,0,0,0,0,1,1,0,0,1,0,1,0,1,1,0,0,1,0,0,1,0,1,0,1,0,0,1,0,0,1,0,0,1,1,1,1,0,0,1,0,0,0,1,0,1,1,0,0,0,1,1,1,0,0,1,1,1,0,0,0,0,0,0,0,0,0,0,1,1,0,0,0,0,1,0,0,1,0,0,0,0,1,1,0,1,0,1,0,1,0,1,1,0,1,0,1,1,1,1,1,1,0,1,0,1,1,1,0,1,1,1,1,0,1,0,1,0,1,0,0,0,0,0,0,1,0,1,1,0,1,1,1,1,1,0,0,1,0,1,1,1,0,1,1,0,0,0,1,1,0,0,1,1,0,0,1,1,0,0,0,0,0,0,1,1,1,0,1,0,1,1,0,0,0,0,1,0,0,1,0,1,1,1,1,1,1,1,1,0,1,0,0,0,1,0,1,1,0,1,0,0,1,1,0,1,0,0,1,1,1,1,0,1,0,0,0,0,0,0,0,0,1,0,1,1,1,1,1,1,1,1,1,0,0,0,0,0,0,0,0,0,0,1,0,1,1,1,0,0,1,1,1,1,0,0,1,1,1,0,1,0,0,1,0,1,1,1,0,1,1,1,0,0,1,1,0,0,0,0,0,1,0,1,1,0,1,1,0,1,1,0,1,0,0,0,0,0,0,0,1,0,1,0,0,1,1,1,0,0,1,1,1,0,0,0,1,1,0,1,0,1,1,1,1,0,1,0,1,1,0,0,0,1,1,0,0,1,0,1,1,1,1,1,0,0,1,1,1,1,0,1,0,1,1,0,1,1,0,1,1,0,1,1,0,1,1,0,1,0,1,1,1,1,1,0,0,1,0,0,0,1,1,1,0,1,0,0,0,0,1,1,0,0,0,0,0,0,0,0,0,0,0,0,1,1,0,0,0,0,1,0,0,0,0,0,1,0,1,0,0,1,0,1,0,0,0,0,1,1,0,1,1,0,1,0,0,0,0,1,0,1,1,0,1,1,0,0,0,0,1,0,1,1,0,1,1,0,1,0,0,1,1,1,0,1,1,0,1,0,1,1,0,0,0,1,1,1,1,0,0,0,1,1,0,1,0,1,1,0,1,1,1,0,0,1,1,0,0,0,0,1,0,0,1,1,1,1,0,0,1,0,1,0,1,0,1,0,0,1,0,1,0,1,0,1,0,0,1,1,1,1,0,0,1,0,0,1,1,1,1,1,0,0,0,0,0,1,1,1,0,0,0,0,0,1,1,1,1,1,1,1,1,1,1,0,0,0,0,0,1,1,1,0,0,0,0,0,0,1,1,1,0,0,0,1,0,1,1,0,1,0,0,0,1,1,1,1,0,0,0,0,0,0,0,0,0,0,1,1,1,1,0,0,0,1,0,1,1,0,1,0,0,0,0,1,1,1,0,1,0,0,0,0,1,0,1,1,0,1,1,0,0,1,0,1,1,1,1,0,1,0,0,1,1,0,1,1,0,1,0,0,0,0,1,0,1,1,0,0,0,1,1,0,1,0,1,1,1,1,1,1,1,1,1,1,1,0,0,1,1,0,0,1,1,0,0,1,1,1,1,1,1,1,1,1,1,1,0,1,0,1,1,0,0,1,0,0,1,1,1,1,1,0,0,0,0,1,1,1,0,1,1,0,0,1,1,1,1,1,1,0,0,1,1,0,1,1,1,0,0,0,0,1,1,1,1,1,0,0,1,0,0,1,0,0,1,1,1,0,0,0,1,1,0,1,0,0,1,1,1,0,0,1,0,0,1,0,0,1,1,1,0,0,1,0,1,1,0,0,0,1,1,1,0,0,1,0,1,1,0,0,0,0,1,0,0,1,0,1,0,0,1,1,1,0,0,1,1,1,1,0,1,1,0,1,1,1,1,0,0,1,1,1,0,0,1,0,1,0,0,1,0,0,0,0,1,0,1,1,0,1,0,0,0,0,1,0,1,0,0,0,1,0,0,1,1,0,0,0,1,0,0,1,0,0,0,1,1,0,0,1,0,0,0,1,0,1,0,0,0,0,1,0,1,1,0]  distributed_mem=Distributed memory  rst=off  init_reg=0  en=off  latency=0  gui_display_data_type=Boolean  arith_type=Boolean  n_bits=2  bin_pt=0  preci_type=Double  exp_width=8  frac_width=24  optimize=Area  use_rpm=on  simulation_type=fast_sim  XmcBlockStatus=1  maskContainerNames=tabcontainer1  block_type=sprom  block_config=sysgen:SPROM_config
  ROM17 : hdlBasic/ROM  depth=1275  initVector=[1,0,0,1,0,0,0,0,0,1,1,1,1,0,0,0,0,0,0,0,1,1,0,0,1,0,0,0,1,0,1,0,1,0,1,1,0,0,1,1,0,0,1,1,0,0,1,1,0,0,0,1,0,0,1,1,0,1,0,1,1,1,0,1,1,0,0,1,0,0,0,1,1,1,1,0,0,1,0,0,0,0,0,0,1,0,1,0,1,0,0,0,0,1,1,1,0,0,0,0,1,0,1,0,1,1,0,1,1,0,0,1,1,1,1,0,0,1,1,0,0,1,0,1,0,0,1,0,1,1,1,0,1,0,0,1,0,0,1,0,1,1,1,1,0,0,1,1,0,0,0,0,0,1,0,1,1,0,0,0,1,0,0,1,0,1,1,0,0,0,0,1,1,1,0,0,0,1,0,1,1,1,1,1,1,1,0,1,0,1,1,1,0,1,1,0,1,0,1,0,1,1,0,0,0,1,1,0,0,0,0,1,0,1,1,0,1,0,0,1,1,1,1,1,1,0,0,0,1,1,1,1,0,1,0,1,0,0,0,0,1,0,1,0,0,0,1,1,1,1,0,1,0,0,1,0,0,0,0,0,0,0,1,0,1,0,0,1,1,0,1,0,0,0,1,1,0,0,1,0,0,1,0,1,0,1,1,1,0,0,0,0,0,1,0,1,0,1,0,0,1,1,0,0,0,0,0,0,0,1,1,0,1,0,0,1,0,0,0,0,1,1,1,1,1,1,1,0,0,0,0,0,0,0,1,1,0,1,0,0,1,0,0,0,0,1,1,1,1,1,1,0,0,1,0,0,1,0,1,0,1,1,1,0,0,0,0,0,1,0,1,0,1,0,0,1,1,0,0,1,0,0,0,0,0,0,0,1,0,1,0,0,1,1,0,1,0,0,0,1,1,0,1,1,0,1,1,0,1,0,1,0,0,0,0,1,0,1,0,0,0,1,1,1,1,0,1,0,1,1,1,1,1,1,0,0,1,0,1,1,0,1,0,0,1,1,1,1,1,1,0,0,0,1,1,1,1,0,0,1,1,0,0,1,1,1,1,0,1,1,0,1,0,1,0,1,1,0,0,0,1,1,0,0,0,1,0,0,1,0,0,1,0,0,1,0,1,1,1,0,0,0,1,0,1,1,1,1,1,1,1,0,1,0,1,0,1,1,0,0,0,0,0,0,1,1,0,1,1,0,1,1,0,0,0,1,0,0,1,0,1,1,0,0,0,0,0,0,0,1,1,1,0,0,1,1,1,0,0,0,0,0,0,1,0,1,1,1,1,0,0,1,1,0,0,0,0,0,0,1,1,0,1,0,0,0,0,0,0,1,0,1,1,0,0,0,1,0,1,0,0,1,0,1,1,1,0,1,0,0,1,0,0,0,1,0,1,1,0,1,1,0,1,1,0,1,0,0,0,1,1,0,1,1,0,0,1,1,1,1,0,0,1,1,0,0,0,0,1,0,1,0,1,0,0,0,0,1,0,1,0,1,0,0,0,0,0,0,1,1,1,0,0,0,0,1,0,1,0,1,1,0,0,1,1,0,1,0,0,0,0,0,0,0,0,1,0,1,1,0,0,1,1,0,0,0,0,0,0,1,0,1,0,1,0,0,0,1,1,0,1,1,0,1,0,0,0,1,1,0,0,0,1,0,1,1,0,1,1,0,0,0,1,0,0,0,1,1,1,1,0,0,1,0,1,0,0,1,0,1,1,1,1,1,1,0,0,1,1,1,1,1,1,0,1,0,0,1,0,1,1,0,1,0,1,1,1,0,1,1,0,0,1,0,0,1,1,1,1,1,1,0,0,1,1,1,1,0,0,1,1,1,1,1,1,0,0,1,0,0,0,1,1,0,0,0,1,0,0,1,1,0,0,1,1,1,0,0,1,0,1,1,1,1,1,1,1,1,1,1,0,1,0,0,1,1,1,0,0,1,1,0,0,1,1,0,0,1,1,0,0,1,1,1,0,1,1,0,0,1,1,0,0,0,0,0,0,0,0,0,0,1,1,0,0,1,1,0,1,1,1,0,0,1,0,1,0,1,0,1,1,1,0,0,1,0,0,1,0,1,1,0,0,0,0,0,1,0,0,1,0,0,0,0,0,1,1,0,1,0,0,1,0,0,1,1,1,0,0,1,0,0,0,1,1,1,1,1,1,0,1,1,1,0,1,1,1,0,0,0,0,0,0,0,0,1,1,1,0,1,1,1,0,1,1,1,1,1,1,0,0,0,0,0,0,1,0,0,0,0,1,1,0,0,0,0,1,0,0,0,0,0,0,1,0,0,1,0,0,0,0,0,0,1,0,0,0,0,1,1,0,0,0,0,1,1,1,1,0,0,0,0,1,0,0,1,0,0,1,0,0,1,0,0,1,1,1,0,0,0,0,0,0,1,1,1,0,0,1,0,0,1,0,0,1,0,0,1,0,0,0,0,0,0,1,0,0,1,0,1,0,0,0,0,1,1,1,0,1,0,1,1,0,0,0,0,0,0,0,0,1,1,0,1,0,1,1,1,0,0,0,0,1,0,1,0,0,1,1,0,0,0,1,0,0,1,1,1,1,0,0,1,1,0,1,1,1,0,0,1,0,1,0,0,1,0,1,0,0,1,1,1,0,1,1,0,0,1,1,1,1,0,0,1,0,0,0,0,0,0,1,0,0,0,0,1,0,1,0,0,0,1,0,0,1,1,1,0,1,0,1,1,0,1,0,1,1,1,0,0,1,0,0,0,1,0,1,0,0,0,0,1,0,0,0,1,0,1,0,1,0,1,1,0,0,1,0,0,0,1,0,0,1,1,1,0,1,0,0,1,1,0,0,1,0,1,1,1,0,0,1,0,0,0,1,0,0,1,1,0,1,0,1,0,1]  distributed_mem=Distributed memory  rst=off  init_reg=0  en=off  latency=0  gui_display_data_type=Boolean  arith_type=Boolean  n_bits=2  bin_pt=0  preci_type=Double  exp_width=8  frac_width=24  optimize=Area  use_rpm=on  simulation_type=fast_sim  XmcBlockStatus=1  maskContainerNames=tabcontainer1  block_type=sprom  block_config=sysgen:SPROM_config
  ROM18 : hdlBasic/ROM  depth=1275  initVector=[1,0,1,0,0,0,0,0,0,0,1,1,0,0,0,0,0,0,0,0,0,0,1,0,0,0,1,0,0,0,0,0,0,0,0,0,1,0,0,0,0,1,0,1,0,0,0,0,0,0,0,1,1,1,0,1,0,0,0,0,1,0,0,0,1,1,1,0,0,1,1,1,0,1,0,1,1,1,1,1,0,1,0,0,1,1,1,0,1,1,1,1,0,1,0,0,1,0,0,1,0,0,1,1,1,0,0,0,0,1,0,0,0,0,0,0,0,1,0,1,0,0,1,0,0,0,1,0,0,0,1,1,0,1,1,1,0,1,1,1,0,0,1,0,1,1,1,0,1,1,0,1,1,1,1,1,1,1,0,0,0,0,0,1,0,1,1,0,1,1,0,0,0,0,0,1,1,1,0,1,1,0,0,0,1,0,1,0,0,0,0,1,0,0,1,0,0,1,1,0,0,1,0,1,1,0,1,0,0,0,0,0,0,0,1,0,0,0,0,1,1,0,0,0,1,1,1,0,0,0,0,0,0,1,0,1,1,0,0,1,0,1,1,1,1,0,1,0,0,0,0,0,0,0,1,1,1,1,0,0,1,0,0,1,1,1,0,1,0,0,0,1,1,0,0,0,1,1,1,1,1,0,1,0,0,0,1,1,1,0,0,1,0,0,0,0,0,1,1,0,1,0,1,1,1,0,0,1,1,0,1,0,0,1,1,0,0,1,0,1,0,0,1,0,0,1,0,1,1,1,0,0,1,1,0,1,0,0,1,1,0,0,1,0,1,0,0,1,0,0,0,1,1,1,1,1,0,1,0,0,0,1,1,1,0,0,1,0,0,0,0,0,1,1,0,0,0,0,0,1,1,1,1,0,0,1,0,0,1,1,1,0,1,0,0,0,1,1,0,0,0,1,1,1,1,0,0,0,1,0,1,1,0,0,1,0,1,1,1,1,0,1,0,0,0,0,0,0,0,1,0,0,1,0,0,0,0,0,0,1,0,0,0,0,1,1,0,0,0,1,1,1,0,0,0,0,0,0,0,0,0,0,0,0,0,0,1,0,0,1,0,0,1,1,0,0,1,0,1,1,0,1,0,0,0,0,0,1,0,1,1,0,1,0,0,0,0,0,0,0,1,1,1,0,1,1,0,0,0,1,0,1,0,0,0,0,0,0,1,0,0,0,0,1,0,0,0,0,1,1,1,1,1,0,0,0,0,0,1,0,1,1,0,1,1,0,0,0,0,0,0,0,1,1,0,0,0,0,0,0,0,0,1,1,1,0,0,1,0,1,1,1,0,1,1,0,1,1,1,0,1,1,0,0,0,0,0,0,0,0,1,1,0,1,1,0,0,1,0,0,0,1,0,0,0,1,1,0,1,1,1,1,1,1,0,1,1,0,1,0,0,1,0,1,1,0,1,1,1,1,0,0,0,0,1,0,0,0,0,0,0,0,1,0,1,1,0,0,0,1,1,0,1,0,1,1,0,1,0,1,1,0,0,0,1,1,1,0,1,0,0,1,0,0,1,0,0,1,1,1,0,1,1,1,1,1,0,1,0,0,1,1,0,0,1,0,1,1,1,1,1,0,1,1,1,0,1,0,0,1,1,1,0,1,1,1,1,1,0,1,1,0,0,0,1,1,1,0,0,1,1,1,0,0,0,1,1,0,1,1,1,1,0,0,1,1,1,0,1,0,1,1,1,1,1,0,1,0,0,0,1,0,1,1,1,0,0,1,1,1,0,1,0,0,0,1,0,1,1,1,1,0,0,0,0,1,0,0,0,1,1,1,1,0,0,1,1,1,0,0,1,1,1,1,1,1,1,1,1,1,0,0,1,1,1,0,0,1,1,1,0,0,0,0,0,0,1,1,1,0,1,1,0,0,0,0,1,0,1,0,1,0,0,0,0,0,0,0,0,1,0,1,0,1,0,0,0,0,1,1,0,1,0,0,0,0,1,0,1,0,1,0,0,1,1,0,0,1,0,1,1,0,1,0,0,1,1,0,0,1,0,1,1,0,1,0,0,1,1,0,0,1,0,0,0,0,0,0,0,0,0,1,1,0,1,1,0,0,0,0,0,0,1,0,0,1,0,1,1,0,1,0,0,1,0,0,0,0,0,0,1,1,0,1,1,0,0,1,0,0,0,1,0,0,0,1,0,0,1,0,0,1,1,0,1,0,0,0,0,1,0,0,1,0,0,0,0,1,0,1,1,0,0,1,0,0,1,0,0,0,0,0,0,0,0,0,1,0,1,0,1,1,0,1,0,0,0,0,1,0,0,1,0,0,0,0,0,0,1,0,0,1,0,0,0,0,1,0,1,1,0,1,0,1,0,1,1,0,0,0,0,0,0,0,0,0,1,0,0,1,0,0,1,1,1,1,1,1,1,1,1,1,1,1,1,1,1,1,0,0,1,0,0,1,0,0,0,0,0,0,0,0,0,0,0,0,0,0,0,0,0,0,1,1,0,0,0,1,1,0,0,0,0,1,1,1,1,1,1,0,0,0,0,1,1,0,0,0,1,1,0,0,0,0,0,0,0,0,0,0,0,0,0,0,0,0,0,0,0,0,0,1,0,1,1,1,0,0,0,1,1,1,1,1,1,1,1,0,0,0,1,1,1,0,1,0,0,0,0,0,0,0,0,0,0,0,0,1,0,0,1,0,1,0,0,0,0,0,1,0,0,0,1,1,0,1,0,0,1,1,0,0,1,1,0,0,1,0,1,1,0,0,0,1,0,0,0,0,0,1,0,1,0,0,1,1,0,0,0,1,0,0,0,1,0,1,1,1,1,0,0,0,1,0,0,0,0,0,1,1,1,1,0,0,0,0,0,1,0,0,0,1,1,1,1,0,1,0,0,0,1,0,0,0,1]  distributed_mem=Distributed memory  rst=off  init_reg=0  en=off  latency=0  gui_display_data_type=Boolean  arith_type=Boolean  n_bits=2  bin_pt=0  preci_type=Double  exp_width=8  frac_width=24  optimize=Area  use_rpm=on  simulation_type=fast_sim  XmcBlockStatus=1  maskContainerNames=tabcontainer1  block_type=sprom  block_config=sysgen:SPROM_config
  ROM19 : hdlBasic/ROM  depth=1275  initVector=[1,0,1,1,0,0,1,0,0,0,0,1,0,0,0,0,0,0,1,1,0,0,0,1,0,0,0,1,1,0,1,0,1,1,0,1,0,1,0,1,0,1,1,0,1,0,0,0,1,1,1,0,1,0,1,0,0,1,0,0,0,1,1,1,0,0,0,1,1,0,0,0,1,0,0,1,1,0,1,0,1,1,1,0,0,0,1,0,0,0,0,0,1,1,1,1,0,0,1,1,0,1,1,0,0,0,1,0,0,1,1,1,0,1,1,0,1,1,0,1,1,0,1,1,0,0,0,0,1,1,1,0,1,0,0,1,0,0,0,0,0,1,1,0,1,0,0,1,1,0,1,1,1,1,1,0,1,1,1,1,1,0,0,1,1,0,0,0,0,0,0,0,1,1,0,0,1,1,0,1,0,1,1,0,0,0,1,0,0,0,0,0,0,0,0,1,0,1,1,1,0,0,1,1,1,1,0,1,1,0,1,0,0,1,1,0,1,1,1,0,0,0,1,0,0,0,0,0,0,0,0,1,1,1,0,0,1,0,1,0,1,0,0,0,1,0,0,0,0,1,1,1,1,1,1,0,0,0,0,0,0,0,1,1,0,1,1,1,0,0,0,1,0,0,1,1,0,1,0,1,1,1,1,0,1,0,0,1,0,1,0,0,1,1,0,1,1,1,0,1,0,1,1,0,0,1,1,0,0,0,0,1,1,1,0,0,1,0,1,1,1,1,1,1,1,0,1,1,0,0,1,1,0,0,0,0,1,1,1,0,0,1,0,1,1,1,1,1,1,1,1,0,1,0,1,1,1,1,0,1,0,0,1,0,1,0,0,1,1,0,1,1,1,0,1,1,1,1,1,1,0,0,0,0,0,0,0,1,1,0,1,1,1,0,0,0,1,0,0,1,1,0,1,1,0,1,1,1,1,0,0,1,0,1,0,1,0,0,0,1,0,0,0,0,1,1,1,1,1,1,1,1,1,1,1,1,0,0,1,1,0,1,1,1,0,0,0,1,0,0,0,0,0,0,0,0,1,0,1,1,1,1,0,1,0,0,0,0,0,0,1,0,1,1,1,0,0,1,1,1,1,0,1,1,0,0,1,0,1,1,1,1,0,1,0,0,0,1,1,0,0,1,1,0,1,0,1,1,0,0,0,1,0,0,0,1,0,1,1,0,1,1,0,1,1,0,1,0,1,1,0,1,1,1,1,1,0,0,1,1,0,0,0,0,0,0,0,1,0,0,0,1,0,0,1,0,0,0,1,0,0,0,0,0,0,0,1,1,0,1,0,0,1,1,0,1,1,1,0,0,0,0,0,0,1,1,1,1,0,0,0,0,0,0,1,1,0,1,1,0,0,0,0,1,1,1,0,1,0,0,1,1,0,1,1,0,0,0,0,0,0,0,0,0,0,1,1,0,1,1,0,1,0,0,1,1,1,0,1,1,0,1,1,0,1,0,1,0,0,1,0,0,1,0,0,0,0,1,0,0,1,0,0,1,0,1,0,1,1,1,1,0,0,1,1,0,1,1,0,0,0,0,0,0,0,1,0,1,1,1,1,1,1,1,1,0,1,0,0,0,0,0,0,1,0,1,1,1,0,0,0,1,0,0,0,0,0,1,1,1,0,0,1,1,0,1,0,1,1,0,1,0,1,1,0,0,1,1,1,0,0,0,1,1,0,0,0,1,0,0,1,1,0,0,1,1,0,1,1,1,0,0,0,0,1,1,1,1,0,0,0,0,1,1,1,0,1,1,0,0,0,0,1,0,0,0,1,1,1,0,0,1,0,1,0,1,0,1,1,0,0,0,1,0,0,0,0,1,0,0,0,1,1,0,1,0,1,0,1,0,0,0,0,1,1,1,0,1,0,1,0,1,0,0,1,1,0,0,0,1,0,1,1,0,0,0,0,1,1,0,1,0,0,0,1,1,0,0,1,0,1,0,1,0,1,0,1,1,0,1,0,1,0,1,1,1,1,1,0,1,1,1,0,0,1,0,0,1,0,0,1,1,1,0,1,1,1,1,1,0,1,0,1,1,0,1,0,1,1,0,1,0,1,1,0,0,1,0,0,0,1,0,1,1,1,0,0,0,0,0,0,1,1,1,0,1,0,0,0,1,0,0,1,1,0,1,0,0,1,0,0,0,1,0,1,0,1,1,0,0,1,0,1,1,1,0,1,0,0,1,1,1,1,0,0,1,0,1,1,1,0,1,0,0,1,1,0,1,0,1,0,0,0,1,1,0,0,1,1,1,0,0,0,0,1,0,1,1,1,1,0,1,0,1,1,1,1,0,1,0,1,1,1,1,0,1,0,0,0,0,1,1,1,0,0,0,1,0,0,0,1,0,1,0,1,0,0,1,1,1,0,0,1,0,0,1,0,0,1,0,0,1,0,0,1,0,0,1,0,0,1,1,1,0,0,1,0,1,0,1,0,1,0,0,0,0,1,0,0,1,1,0,0,1,1,0,1,0,1,0,0,1,0,0,1,0,0,1,0,0,1,0,0,1,0,1,0,1,1,0,0,1,1,0,0,1,0,0,1,0,0,0,0,0,1,1,0,0,1,1,1,1,0,1,0,0,1,0,0,1,0,0,1,1,0,0,1,0,0,1,0,0,1,0,1,1,1,1,0,0,1,1,0,0,0,0,0,1,0,0,1,0,0,0,1,0,0,1,0,1,1,0,0,1,1,0,0,1,1,1,1,1,1,1,1,0,0,1,1,0,0,1,1,0,1,0,0,1,0,0,0,1,0,0,1,1,0,1,1,0,0,0,1,0,0,0,0,1,0,0,1,0,1,0,0,1,1,1,0,0,0,0,1,1,1,0,0,1,0,1,0,0,1,0,0,0,0,1,0,0,0,1,1,0,1]  distributed_mem=Distributed memory  rst=off  init_reg=0  en=off  latency=0  gui_display_data_type=Boolean  arith_type=Boolean  n_bits=2  bin_pt=0  preci_type=Double  exp_width=8  frac_width=24  optimize=Area  use_rpm=on  simulation_type=fast_sim  XmcBlockStatus=1  maskContainerNames=tabcontainer1  block_type=sprom  block_config=sysgen:SPROM_config
  ROM2 : hdlBasic/ROM  depth=1275  initVector=[0,0,0,0,0,0,0,0,0,0,0,0,0,0,0,0,0,0,0,0,0,0,0,0,0,0,0,0,0,0,0,0,0,0,0,0,0,0,0,0,0,0,0,1,1,0,0,0,0,0,0,1,1,1,1,0,0,0,0,0,1,1,1,1,1,1,0,0,0,0,0,1,1,1,1,1,1,1,0,0,0,0,1,1,1,1,1,1,1,1,1,0,0,0,1,1,1,1,1,1,1,1,1,1,1,0,0,0,1,1,1,1,1,1,1,1,1,1,1,1,0,0,1,1,1,1,1,1,1,1,1,1,1,1,1,1,0,0,1,1,1,1,1,1,1,1,1,1,1,1,1,1,0,0,0,1,1,1,1,1,1,1,1,1,1,1,1,1,0,0,0,0,1,1,1,1,1,1,1,1,1,1,1,1,1,1,0,0,0,0,0,1,1,1,1,1,1,1,1,1,1,1,1,1,0,0,0,0,0,0,0,1,1,1,1,1,1,1,1,1,1,1,1,1,0,0,0,0,0,0,0,0,1,1,1,1,1,1,1,1,1,1,1,1,0,0,0,0,0,0,0,0,0,0,1,1,1,1,1,1,1,1,1,1,1,1,0,0,0,0,0,0,0,0,0,0,0,1,1,1,1,1,1,1,1,1,1,1,1,0,0,0,0,0,0,0,0,0,0,0,0,1,1,1,1,1,1,1,1,1,1,1,1,0,0,0,0,0,0,0,0,0,0,0,0,0,1,1,1,1,1,1,1,1,1,1,1,1,0,0,0,0,0,0,0,0,0,0,0,0,0,0,1,1,1,1,1,1,1,1,1,1,1,1,0,0,0,0,0,0,0,0,0,0,0,0,0,0,0,1,1,1,1,1,1,1,1,1,1,1,1,0,0,0,0,0,0,0,0,0,0,0,0,0,0,0,0,1,1,1,1,1,1,1,1,1,1,1,1,0,0,0,0,0,0,0,0,0,0,0,0,0,0,0,0,0,1,1,1,1,1,1,1,1,1,1,1,1,1,0,0,0,0,0,0,0,0,0,0,0,0,0,0,0,0,0,1,1,1,1,1,1,1,1,1,1,1,1,1,0,0,0,0,0,0,0,0,0,0,0,0,0,0,0,0,0,0,1,1,1,1,1,1,1,1,1,1,1,1,1,1,0,0,0,0,0,0,0,0,0,0,0,0,0,0,0,0,0,0,0,1,1,1,1,1,1,1,1,1,1,1,1,1,0,0,0,0,0,0,0,0,0,0,0,0,0,0,0,0,0,0,0,0,1,1,1,1,1,1,1,1,1,1,1,1,1,1,0,0,0,0,0,0,0,0,0,0,0,0,0,0,0,0,0,0,0,0,1,1,1,1,1,1,1,1,1,1,1,1,1,1,1,0,0,0,0,0,0,0,0,0,0,0,0,0,0,0,0,1,1,0,0,0,1,1,1,1,1,1,1,1,1,1,1,1,1,1,1,1,0,0,0,0,0,0,0,0,0,0,0,0,1,1,1,1,1,0,0,0,1,1,1,1,1,1,1,1,1,1,1,1,1,1,1,1,1,1,0,0,0,0,0,0,0,0,1,1,1,1,1,1,1,1,0,0,0,0,1,1,1,1,1,1,1,1,1,1,1,1,1,1,1,1,1,1,1,1,1,1,1,1,1,1,1,1,1,1,1,1,1,1,0,0,0,0,0,1,1,1,1,1,1,1,1,1,1,1,1,1,1,1,1,1,1,1,1,1,1,1,1,1,1,1,1,1,1,1,1,1,1,0,0,0,0,0,1,1,1,1,1,1,1,1,1,1,1,1,1,1,1,1,1,1,1,1,1,1,1,1,1,1,1,1,1,1,1,1,1,1,1,0,0,0,0,0,0,1,1,1,1,1,1,1,1,1,1,1,1,1,1,1,1,1,1,1,1,1,1,1,1,1,1,1,1,1,1,1,1,1,1,1,0,0,0,0,0,0,0,1,1,1,1,1,1,1,1,1,1,1,1,1,1,1,1,1,1,1,1,1,1,1,1,1,1,1,1,1,1,1,1,1,1,1,0,0,0,0,0,0,0,0,1,1,1,1,1,1,1,1,1,1,1,1,1,1,1,1,1,1,1,1,1,1,1,1,1,1,1,1,1,1,1,1,1,1,0,0,0,0,0,0,0,0,0,0,1,1,1,1,1,1,1,1,1,1,1,1,1,1,1,1,1,1,1,1,1,1,1,1,1,1,1,1,1,1,1,1,0,0,0,0,0,0,0,0,0,0,0,0,0,1,1,1,1,1,1,1,1,1,1,1,1,1,1,1,1,1,1,1,1,1,1,1,1,1,1,1,1,1,1,0,0,0,0,0,0,0,0,0,0,0,0,0,0,0,0,0,1,1,1,1,1,1,1,1,1,1,1,1,1,1,1,1,1,1,1,1,1,1,1,1,1,1,0,0,0,0,0,0,0,0,0,0,0,0,0,0,0,0,0,0,0,0,0,1,1,1,1,1,1,1,1,1,1,1,1,1,1,1,1,1,1,1,1,1,1,1,1,0,0,0,0,0,0,0,0,0,0,0,0,0,0,0,0,0,0,0,0,0,0,0,0,0,1,1,1,1,1,1,1,1,1,1,1,1,1,1,1,1,1,1,1,1,0,0,0,0,0,0,0,0,0,0,0,0,0,0,0,0,0,0,0,0,0,0,0,0,0,0,0,0,0,0,0,1,1,1,1,1,1,1,1,1,1,1,1,1,1,0,0,0,0,0,0,0,0,0,0,0,0,0,0,0,0,0,0,0,0,0,0,0,0,0,0,0,0,0,0,0,0,0,0,0,0,0,0,0,0,0,0,0,0,0,0,0,0,0,0,0,0,0,0,0,0,0,0,0,0,0,0,0,0,0,0,0]  distributed_mem=Distributed memory  rst=off  init_reg=0  en=off  latency=0  gui_display_data_type=Boolean  arith_type=Boolean  n_bits=2  bin_pt=0  preci_type=Double  exp_width=8  frac_width=24  optimize=Area  use_rpm=on  simulation_type=fast_sim  XmcBlockStatus=1  maskContainerNames=tabcontainer1  block_type=sprom  block_config=sysgen:SPROM_config
  ROM20 : hdlBasic/ROM  depth=1275  initVector=[1,1,1,1,0,0,0,0,0,0,1,0,0,1,1,1,1,0,0,0,1,0,0,0,1,1,1,0,1,1,1,1,1,1,0,0,1,1,0,0,0,0,0,1,1,1,1,0,1,1,0,1,1,0,1,0,1,1,1,0,0,0,0,1,0,0,0,0,1,1,1,1,0,0,0,0,0,0,1,0,1,0,1,1,1,1,1,1,0,0,1,0,0,0,0,0,0,1,0,0,0,1,0,0,1,0,1,1,1,0,1,1,0,1,0,1,1,1,1,0,0,1,1,0,1,1,1,1,0,1,1,1,1,0,0,1,1,1,1,0,1,1,0,1,0,1,1,1,1,0,1,1,1,1,0,1,1,1,1,0,0,0,1,1,0,0,1,0,1,0,0,1,0,0,0,1,0,1,1,0,1,1,1,1,0,0,0,0,0,0,0,1,1,1,0,1,0,1,1,1,0,0,0,1,0,1,1,0,0,1,0,1,0,1,0,1,0,0,1,0,0,0,1,0,0,1,1,1,1,0,1,0,1,1,1,1,0,1,1,0,1,0,0,1,1,1,1,0,0,1,1,1,0,0,0,0,1,0,1,1,1,1,1,1,1,1,0,1,0,0,1,0,1,0,0,0,1,1,1,1,0,1,0,0,1,1,0,1,0,0,0,1,0,0,0,1,0,0,1,1,1,0,1,1,0,1,1,0,1,0,1,1,1,0,1,0,0,0,1,0,0,0,0,1,1,1,0,1,1,0,1,1,0,1,0,1,1,1,0,1,0,0,0,1,0,0,0,0,1,1,1,1,1,1,1,0,1,0,0,1,1,0,1,0,0,0,1,0,0,0,1,0,0,1,1,1,1,1,0,0,0,1,0,1,1,1,1,1,1,1,1,0,1,0,0,1,0,1,0,0,0,1,0,0,1,0,0,1,1,1,1,0,1,1,0,1,0,0,1,1,1,1,0,0,1,1,1,0,0,0,0,0,0,0,0,0,1,0,1,0,1,0,0,1,0,0,0,1,0,0,1,1,1,1,0,1,1,0,0,0,0,0,0,1,1,0,1,1,1,0,1,0,1,1,1,0,0,0,1,0,1,1,0,0,1,0,1,1,1,0,0,1,1,1,0,1,1,0,0,0,1,0,1,1,0,1,1,1,1,0,0,0,0,0,0,0,1,1,0,0,1,1,0,0,1,1,0,0,1,0,1,1,1,1,0,0,0,1,1,0,0,1,0,1,0,0,0,0,1,0,1,0,0,0,0,1,0,1,0,0,0,1,1,1,0,1,1,0,1,0,1,1,1,1,0,1,1,1,0,0,1,1,0,0,0,0,0,0,0,0,1,1,0,0,1,0,1,1,0,1,1,1,1,0,1,1,1,1,0,0,1,1,1,0,1,1,1,0,1,0,0,1,0,1,1,1,0,1,1,1,0,1,1,1,0,1,1,0,1,0,1,1,1,1,0,0,1,0,0,0,0,1,1,0,1,1,0,1,1,0,0,0,0,1,0,0,0,0,0,0,0,0,1,0,0,0,1,0,0,1,1,0,0,1,0,1,0,1,0,0,0,0,0,0,1,0,1,0,1,0,0,1,1,1,0,1,0,1,1,1,1,1,1,0,0,1,0,1,1,1,0,1,0,1,1,1,0,1,1,0,1,1,1,0,1,0,1,1,1,0,1,0,0,1,1,1,1,0,0,0,0,0,0,0,0,1,1,1,0,1,0,0,0,1,1,1,1,1,1,0,0,0,1,0,1,1,1,0,0,0,0,1,1,1,0,0,0,0,1,0,0,0,0,1,1,1,1,1,1,0,0,0,1,0,1,1,0,1,0,0,0,1,1,1,1,1,1,0,0,0,1,1,0,1,1,0,1,1,0,1,0,0,1,0,0,1,1,1,1,1,0,1,1,1,0,0,1,1,1,0,1,1,1,1,1,0,0,1,0,0,1,1,1,0,0,0,0,0,1,1,0,1,0,1,0,1,0,0,0,0,1,1,0,1,1,1,1,1,1,0,1,1,0,0,0,0,1,0,1,0,1,0,1,1,1,1,1,1,1,0,0,1,1,0,0,1,0,0,1,1,0,1,1,0,1,1,0,0,0,0,1,1,0,1,1,0,1,1,0,0,1,0,0,1,1,0,0,0,0,1,1,1,0,0,0,1,0,0,1,1,1,1,0,0,1,0,0,1,1,0,1,1,0,1,1,0,0,1,0,0,1,1,1,1,0,0,1,0,0,0,1,1,0,0,0,1,1,1,0,0,0,1,1,0,1,1,1,1,0,1,1,0,1,1,1,1,1,1,0,1,1,0,1,1,1,1,0,1,1,0,0,0,1,1,1,1,0,0,1,1,0,1,1,0,1,0,1,1,0,0,1,1,1,1,0,0,1,0,0,0,0,0,0,1,0,0,1,1,1,1,0,0,1,1,0,1,0,1,1,0,1,0,0,0,0,1,0,1,1,0,1,1,1,0,0,1,0,0,1,0,1,1,1,1,1,1,1,1,1,1,1,1,0,1,0,0,1,0,0,1,1,1,0,1,1,0,1,0,1,0,0,0,0,0,0,1,0,0,1,1,1,0,1,1,1,1,0,1,0,1,0,1,1,1,1,0,1,0,1,0,1,1,1,1,0,1,1,1,0,0,1,0,0,0,0,0,1,1,0,0,0,1,0,1,1,1,1,0,0,0,1,1,1,0,0,1,1,1,0,1,0,0,1,0,1,1,1,0,0,1,1,1,0,0,0,1,1,1,1,0,1,0,0,0,1,1,1,1,0,1,1,0,1,1,1,0,0,1,0,0,0,1,1,1,0,0,0,0,1,1,1,1,0,0,0,0,1,1,1,0,0,0,1,0,0,1,1,1,0,1,1,0,1,1,1]  distributed_mem=Distributed memory  rst=off  init_reg=0  en=off  latency=0  gui_display_data_type=Boolean  arith_type=Boolean  n_bits=2  bin_pt=0  preci_type=Double  exp_width=8  frac_width=24  optimize=Area  use_rpm=on  simulation_type=fast_sim  XmcBlockStatus=1  maskContainerNames=tabcontainer1  block_type=sprom  block_config=sysgen:SPROM_config
  ROM21 : hdlBasic/ROM  depth=1275  initVector=[0,0,1,0,0,0,1,0,0,1,0,0,0,0,0,1,1,0,1,1,1,0,1,1,0,0,0,0,0,0,1,1,0,1,1,1,0,1,1,0,1,1,1,1,0,0,1,1,1,1,0,1,1,0,1,1,0,1,0,1,1,0,1,0,0,0,1,0,1,0,1,1,1,1,0,1,1,1,1,1,1,1,0,1,0,1,0,1,0,0,0,0,0,1,1,0,0,1,0,1,0,1,0,1,1,0,1,0,0,0,1,0,0,0,0,0,1,0,1,1,1,1,1,0,1,0,1,1,1,1,0,1,0,0,1,0,0,1,1,1,0,0,0,0,0,0,0,1,1,0,0,0,1,1,1,1,1,0,0,1,1,1,1,0,0,1,0,0,1,0,0,1,1,0,0,1,1,1,0,0,0,1,1,1,0,0,1,1,0,1,1,1,1,0,0,0,0,0,1,0,1,1,0,0,0,1,1,1,0,0,0,0,0,0,1,1,1,0,1,0,0,0,1,0,1,0,1,0,1,0,1,1,0,1,1,1,1,1,1,0,1,0,1,1,1,0,1,1,0,1,1,1,0,0,0,0,0,0,1,0,0,1,0,0,0,0,0,1,1,0,1,0,1,1,1,1,1,1,1,1,1,0,0,1,1,1,1,0,1,1,0,1,0,1,1,1,1,1,1,0,0,0,1,1,0,1,1,0,1,1,0,0,1,1,0,1,0,1,1,1,0,1,0,1,1,0,0,1,1,0,1,1,0,1,1,0,0,1,1,0,1,0,1,1,1,0,1,0,1,1,1,1,1,1,1,1,0,0,1,1,1,1,0,1,1,0,1,0,1,1,1,1,1,1,0,1,1,0,0,0,0,0,0,1,0,0,1,0,0,0,0,0,1,1,0,1,0,1,1,1,1,1,0,0,1,1,1,0,1,1,1,1,1,1,0,1,0,1,1,1,0,1,1,0,1,1,1,0,1,1,1,1,1,1,0,0,0,0,0,1,1,1,0,1,0,0,0,1,0,1,0,1,0,1,0,1,1,1,1,0,0,1,1,1,1,1,1,1,0,0,0,0,0,1,0,1,1,0,0,0,1,1,1,0,0,0,1,1,1,1,1,1,1,1,0,0,1,1,0,0,1,1,1,0,0,0,1,1,1,0,0,1,1,0,1,0,1,1,0,1,1,1,1,0,1,1,0,1,1,1,1,1,0,0,1,1,1,1,0,0,1,0,0,1,0,0,0,1,0,0,1,1,1,1,1,1,0,0,1,0,0,0,1,1,1,0,0,0,0,0,0,0,1,1,0,0,0,1,0,1,1,1,1,0,0,0,0,0,0,1,1,1,1,0,1,1,1,1,0,1,0,1,1,1,1,0,1,0,0,1,0,0,1,1,1,0,1,1,1,1,1,1,1,1,0,1,1,1,0,0,0,1,0,0,0,1,0,0,0,0,0,1,0,1,1,1,0,0,0,0,1,0,1,0,0,0,0,1,0,1,0,0,0,0,1,1,0,0,1,1,0,0,1,0,1,0,1,0,1,1,1,0,0,0,0,0,0,1,0,1,1,1,1,0,1,0,0,0,0,0,0,1,1,1,1,1,1,0,1,0,1,0,1,0,0,0,1,0,0,1,1,1,0,1,1,0,1,1,1,1,0,1,1,0,1,1,1,0,0,1,0,1,0,1,0,1,1,1,1,0,1,1,1,0,0,1,1,1,0,1,1,0,1,0,0,0,0,0,0,1,0,1,1,0,1,1,1,0,0,1,1,0,1,0,1,1,0,1,0,0,0,1,0,1,0,0,0,0,1,1,0,0,0,1,0,0,1,0,0,0,1,1,0,0,0,0,1,0,1,0,0,1,1,1,1,0,1,1,0,1,0,1,1,0,0,1,0,1,0,0,0,1,0,1,1,1,1,0,1,0,0,0,1,0,1,0,0,1,1,0,1,0,1,1,0,1,1,1,1,0,0,0,0,0,1,0,1,0,1,0,1,1,0,1,1,1,1,1,1,0,1,1,0,1,0,1,0,1,0,0,0,0,0,0,0,1,1,0,1,1,1,1,1,1,1,1,0,0,1,0,1,0,0,0,1,0,1,0,0,1,0,1,0,0,0,1,0,1,0,0,1,1,1,1,1,1,0,1,1,0,0,0,0,1,1,1,0,1,0,1,0,1,0,1,1,0,1,1,0,0,1,1,0,0,1,1,0,1,1,0,1,0,1,0,1,0,1,1,1,0,1,1,0,1,1,1,0,1,1,0,1,1,1,0,1,0,0,0,1,0,1,1,1,0,1,1,0,1,1,1,0,1,0,0,0,1,0,1,1,1,0,1,1,0,1,0,0,0,0,0,1,0,0,1,1,1,1,0,0,0,1,0,0,1,0,1,1,0,1,0,0,1,0,1,1,0,1,0,0,1,0,0,0,1,1,1,1,0,0,1,0,1,0,0,1,0,1,0,1,0,1,0,0,1,1,0,0,1,1,0,0,0,1,0,1,1,1,1,0,1,0,0,0,1,1,0,0,1,1,0,0,1,0,1,0,1,0,1,0,0,0,0,0,0,1,1,1,1,1,1,1,1,0,1,1,1,0,1,0,1,0,1,1,1,1,0,1,0,1,0,1,1,1,0,1,1,1,1,1,1,1,1,0,0,0,0,0,1,0,0,0,1,1,0,1,1,0,0,1,0,1,1,1,1,1,1,0,0,0,1,0,0,1,0,0,0,1,1,1,1,1,1,0,1,0,0,1,1,0,1,1,0,0,0,1,0,0,0,1,0,1,0,0,0,0,1,1,1,0,0,1,0,1,1,1,0,1,0,1,0,0,1,0,1,0,1,1,1,0,1,0,0,1,1,1,0,0,0,0,1,0,1,0,0,0]  distributed_mem=Distributed memory  rst=off  init_reg=0  en=off  latency=0  gui_display_data_type=Boolean  arith_type=Boolean  n_bits=2  bin_pt=0  preci_type=Double  exp_width=8  frac_width=24  optimize=Area  use_rpm=on  simulation_type=fast_sim  XmcBlockStatus=1  maskContainerNames=tabcontainer1  block_type=sprom  block_config=sysgen:SPROM_config
  ROM22 : hdlBasic/ROM  depth=1275  initVector=[0,0,0,1,1,0,0,1,1,1,0,1,0,0,1,0,1,0,1,0,1,1,0,1,1,1,0,1,1,1,1,0,0,0,0,1,0,1,1,1,0,1,1,0,1,1,0,0,1,0,1,1,0,0,1,0,1,1,0,0,0,1,1,0,1,1,1,1,1,1,0,1,1,0,1,1,1,1,1,1,0,0,0,0,1,1,0,0,1,0,1,0,1,1,1,1,0,1,0,1,0,0,0,1,1,1,0,1,1,0,1,1,1,0,0,0,1,1,1,0,1,1,0,1,1,0,1,0,0,1,0,1,0,1,1,0,0,0,0,1,0,1,1,0,0,1,1,0,0,1,1,1,0,0,0,1,0,1,0,1,0,1,1,1,0,1,0,1,0,0,0,1,1,0,0,1,1,1,1,0,1,0,1,1,0,1,1,1,0,0,0,1,0,0,1,0,0,1,0,1,1,1,1,1,0,1,0,1,1,0,1,1,1,0,1,0,0,1,1,1,0,1,0,1,0,1,1,1,1,0,0,1,1,0,1,1,1,0,1,1,0,1,0,1,0,0,0,0,1,1,0,1,0,1,0,0,1,0,1,1,1,1,0,0,0,1,1,1,1,0,1,1,0,0,1,0,0,1,1,1,1,0,0,0,1,1,1,0,1,1,0,1,1,1,0,1,1,1,1,0,0,1,1,1,1,0,0,1,1,1,1,1,1,1,1,0,1,0,0,0,1,0,1,0,0,0,1,1,1,1,0,0,1,1,1,1,1,1,1,1,0,1,0,0,0,1,0,1,0,0,0,0,1,1,1,1,0,0,0,1,1,1,0,1,1,0,1,1,1,0,1,1,1,1,0,0,0,0,1,0,0,1,0,1,1,1,1,0,0,0,1,1,1,1,0,1,1,0,0,1,0,1,1,1,1,0,1,1,0,1,1,1,0,1,1,0,1,0,1,0,0,0,0,1,1,0,1,0,1,1,0,0,1,1,0,1,1,1,0,1,0,0,1,1,1,0,1,0,1,0,1,1,1,1,0,0,1,0,1,1,1,1,0,1,0,0,1,0,0,1,0,0,1,0,1,1,1,1,1,0,1,0,1,1,0,0,0,0,1,0,0,1,0,0,0,0,1,1,0,0,1,1,1,1,0,1,0,1,1,0,1,1,1,0,0,1,1,1,1,0,0,0,0,1,1,1,1,0,0,0,1,0,1,0,1,0,1,1,1,0,1,0,1,0,0,0,0,1,1,1,1,1,0,0,1,1,1,1,1,0,0,0,0,0,1,0,1,1,0,0,1,1,0,0,1,1,1,0,0,1,0,1,0,0,1,1,1,1,0,0,1,0,1,0,0,1,1,0,1,1,0,1,0,0,1,0,1,0,1,1,0,1,0,1,1,1,0,1,1,0,0,1,1,0,1,1,1,0,1,0,1,0,1,1,0,1,1,1,0,0,0,1,1,1,0,1,1,1,1,0,0,0,1,0,1,1,0,1,0,0,0,1,1,1,1,0,0,1,1,1,1,0,1,0,1,0,0,0,1,1,1,1,1,0,0,1,1,0,1,1,1,1,1,1,0,1,1,0,0,1,1,1,1,1,1,0,0,0,0,1,1,0,0,1,0,1,1,1,0,0,1,1,1,0,1,1,1,1,1,1,1,1,0,1,1,1,0,0,1,1,1,1,1,1,1,0,1,1,0,1,1,1,1,0,0,1,1,0,0,1,1,1,0,0,0,1,1,0,0,0,1,1,1,0,0,1,1,0,0,1,0,1,1,0,0,0,1,1,0,1,1,1,1,0,0,0,1,1,0,1,0,1,0,1,1,1,1,0,1,0,1,0,1,1,0,0,0,1,1,1,1,0,0,1,0,1,1,0,0,1,1,1,0,0,0,1,1,1,1,1,1,0,0,1,1,1,1,0,0,1,1,1,1,1,1,0,0,0,1,1,1,0,1,1,1,0,1,1,0,1,0,0,1,0,1,0,0,0,1,0,0,1,1,1,1,1,1,1,1,1,1,0,0,1,0,0,0,1,0,1,0,0,1,1,1,1,0,0,0,0,1,0,0,1,0,1,0,1,0,0,0,1,1,1,1,1,0,1,1,0,1,1,1,1,1,0,0,0,1,0,1,0,1,0,0,1,1,0,1,1,1,0,1,0,1,1,1,1,1,1,1,1,1,1,1,0,0,0,1,0,0,0,0,1,0,0,0,1,1,1,1,1,1,1,1,1,1,1,0,1,0,1,0,1,0,1,0,0,1,1,0,1,0,0,1,0,1,0,1,0,0,1,1,0,0,0,0,1,1,0,0,1,0,1,0,1,0,0,1,0,1,1,0,0,1,0,1,0,0,1,0,1,0,0,0,0,0,0,1,0,1,0,1,1,1,1,1,0,1,1,1,1,0,1,1,1,1,1,0,1,0,1,0,0,0,0,0,0,1,0,1,0,1,1,1,0,1,1,0,1,1,0,1,0,1,1,1,1,0,0,0,0,1,1,1,1,1,1,1,1,0,0,0,0,1,1,1,1,0,1,0,1,1,0,1,1,0,1,1,1,0,1,0,0,1,1,1,0,1,1,0,1,1,0,0,1,0,0,1,0,0,1,1,1,1,0,0,1,0,0,1,0,0,1,1,0,1,1,0,1,1,1,0,0,1,0,0,0,1,1,1,1,0,1,1,0,1,1,1,1,0,1,0,0,1,1,1,1,0,1,1,1,1,0,1,1,1,1,0,0,1,0,1,1,1,1,0,1,1,0,1,1,1,1,0,0,0,1,0,0,0,1,1,0,1,0,1,1,0,1,1,0,0,1,0,1,1,1,0,0,0,0,1,1,1,0,1,0,0,1,1,0,1,1,0,1,0,1,1,0,0,0,1,0,0]  distributed_mem=Distributed memory  rst=off  init_reg=0  en=off  latency=0  gui_display_data_type=Boolean  arith_type=Boolean  n_bits=2  bin_pt=0  preci_type=Double  exp_width=8  frac_width=24  optimize=Area  use_rpm=on  simulation_type=fast_sim  XmcBlockStatus=1  maskContainerNames=tabcontainer1  block_type=sprom  block_config=sysgen:SPROM_config
  ROM23 : hdlBasic/ROM  depth=1275  initVector=[1,0,1,0,1,1,1,1,1,0,0,0,1,1,0,0,1,1,1,1,0,1,1,0,1,0,1,0,1,0,1,1,1,1,1,0,0,0,0,0,0,0,0,0,1,0,1,1,1,0,0,1,0,0,1,1,0,0,0,0,0,0,1,1,0,1,0,0,0,1,1,1,0,1,0,0,0,1,0,1,0,0,0,0,0,0,0,1,0,0,1,0,0,0,0,0,0,1,0,1,0,0,0,0,1,0,0,1,1,0,1,1,0,1,0,0,1,0,1,0,0,1,1,0,0,0,0,1,0,0,1,1,1,1,0,0,0,1,0,0,1,1,1,0,1,1,0,0,1,1,1,0,0,1,1,1,0,0,0,1,0,1,1,0,1,0,1,0,1,1,0,1,0,1,0,0,0,1,0,0,0,0,0,0,1,1,0,0,0,0,0,1,0,1,0,1,0,0,0,0,1,0,1,0,1,0,0,1,0,1,0,1,0,1,1,0,0,1,1,0,1,0,0,1,1,1,1,0,1,0,1,0,1,0,1,0,0,0,0,0,0,1,0,0,0,1,0,0,1,1,1,1,1,1,1,0,1,0,1,0,1,0,1,0,1,0,0,1,0,1,1,0,1,1,0,1,1,1,0,0,0,1,1,0,1,1,0,1,1,1,0,1,1,0,0,1,0,1,0,1,1,0,0,0,1,0,0,0,1,1,0,1,0,0,1,1,0,0,1,1,1,1,0,0,1,1,0,0,0,1,0,0,0,1,1,0,1,0,0,1,1,0,0,1,1,1,1,0,0,1,1,1,1,0,0,0,1,1,0,1,1,0,1,1,1,0,1,1,0,0,1,0,1,0,1,0,0,1,1,1,0,1,0,1,0,1,0,1,0,1,0,0,1,0,1,1,0,1,1,0,1,0,0,0,0,1,0,1,0,1,0,0,0,0,0,0,1,0,0,0,1,0,0,1,1,1,1,1,0,1,1,1,1,0,1,0,1,0,1,1,0,0,1,1,0,1,0,0,1,1,1,1,0,1,0,1,1,1,0,1,1,0,1,1,1,0,1,0,1,0,1,0,0,0,0,1,0,1,0,1,0,0,1,0,1,0,1,1,1,1,1,1,1,1,0,1,1,0,1,0,0,0,1,0,0,0,0,0,0,1,1,0,0,0,0,0,1,1,0,0,1,1,0,0,1,1,0,0,1,1,1,0,0,0,1,0,1,1,0,1,0,1,0,1,1,0,0,1,0,1,1,0,0,0,0,1,1,0,1,0,0,0,1,0,0,1,1,1,0,1,1,0,0,1,1,1,0,0,1,0,0,1,0,1,1,0,0,1,1,0,1,0,0,1,0,0,1,1,0,0,0,0,1,0,0,1,1,1,1,0,0,0,1,0,0,1,0,0,1,1,1,1,0,0,1,0,0,1,0,0,0,0,1,1,0,1,1,0,1,0,0,1,0,1,0,0,1,0,1,1,1,1,1,0,1,1,0,1,1,1,1,1,0,1,0,0,0,0,0,0,0,0,1,0,1,0,0,0,0,1,1,1,1,1,1,0,1,0,0,1,0,0,1,0,0,1,0,1,1,1,1,1,1,0,1,0,0,0,0,0,0,0,1,0,0,1,0,0,1,1,0,0,1,0,0,0,1,0,0,1,0,0,0,1,0,0,1,1,0,0,1,0,0,0,1,1,1,0,1,0,0,0,1,0,0,1,1,0,1,0,0,0,0,1,1,1,1,1,1,0,0,0,0,1,0,1,1,0,0,1,1,0,0,0,0,0,0,1,1,0,1,0,0,0,0,1,0,0,0,1,1,1,0,0,0,0,0,0,1,1,1,0,0,0,1,0,0,0,0,1,0,1,1,1,0,0,1,0,0,1,0,0,1,0,0,0,1,1,0,0,0,0,1,1,1,1,1,1,0,0,0,0,1,1,0,0,0,1,0,0,1,0,0,0,0,0,0,0,0,1,0,1,0,0,1,1,0,1,1,0,0,1,0,0,1,1,1,1,0,0,1,0,0,1,1,0,1,1,0,0,1,0,1,1,0,1,1,1,1,1,0,0,0,1,1,0,0,0,1,0,0,0,0,1,0,1,0,0,0,0,1,0,1,0,0,0,0,1,0,0,0,1,1,0,0,0,1,1,0,1,0,1,0,1,0,1,0,0,0,1,1,0,1,1,1,0,0,0,0,1,0,0,1,0,0,0,0,1,1,1,0,1,1,0,0,0,1,0,1,0,0,1,1,1,1,0,1,1,0,0,0,1,0,0,1,0,1,0,0,1,0,0,1,1,0,0,1,1,0,0,1,0,0,1,0,1,0,0,1,0,0,0,1,1,0,0,0,1,1,0,1,0,1,0,0,0,1,0,0,0,0,1,0,0,0,1,0,0,0,1,1,0,0,0,1,0,0,0,1,0,0,0,0,1,0,0,0,1,0,1,0,1,1,1,0,1,1,1,1,0,1,0,1,0,0,1,0,0,0,0,1,1,1,1,0,0,0,0,1,1,1,1,0,0,0,0,1,0,0,1,0,1,0,1,1,1,1,0,0,1,1,1,1,1,0,1,0,1,0,0,0,0,1,1,0,1,1,0,0,0,0,0,0,0,0,0,0,0,0,1,1,0,1,1,0,0,0,0,1,0,1,0,1,1,1,1,0,1,1,1,0,1,1,0,0,1,0,0,1,0,0,1,1,1,0,1,1,1,1,1,0,0,1,1,1,1,1,0,1,1,1,0,0,1,0,0,1,0,0,1,1,0,1,1,1,1,0,0,1,0,0,1,1,0,0,1,0,0,0,0,0,0,1,1,0,0,0,1,1,1,1,1,1,0,0,0,1,1,0,0,0,0,0,0,1,0,0,1,1,0,0,1,0,0,1]  distributed_mem=Distributed memory  rst=off  init_reg=0  en=off  latency=0  gui_display_data_type=Boolean  arith_type=Boolean  n_bits=2  bin_pt=0  preci_type=Double  exp_width=8  frac_width=24  optimize=Area  use_rpm=on  simulation_type=fast_sim  XmcBlockStatus=1  maskContainerNames=tabcontainer1  block_type=sprom  block_config=sysgen:SPROM_config
  ROM24 : hdlBasic/ROM  depth=1275  initVector=[1,1,1,1,1,1,1,0,0,0,0,0,1,0,0,0,0,1,1,0,0,1,0,1,1,0,0,1,0,0,0,0,1,0,1,1,1,1,1,0,0,0,1,1,0,0,0,0,1,1,1,1,1,0,0,0,0,0,0,0,0,0,0,0,0,0,0,0,1,1,1,1,1,1,0,0,0,1,0,1,1,0,1,0,0,1,0,0,0,1,1,1,1,0,0,0,0,1,1,0,1,0,1,1,1,1,1,0,1,0,1,0,0,1,0,0,0,1,1,0,0,0,1,0,1,0,0,0,0,0,0,1,0,0,1,0,0,1,1,0,1,0,1,1,0,1,1,1,0,1,1,0,0,1,0,1,1,1,0,1,0,0,0,1,0,0,1,1,0,1,1,0,0,0,0,1,0,1,1,1,1,0,0,0,1,1,1,0,1,1,0,1,0,1,0,1,1,0,0,0,1,0,0,0,0,0,0,1,0,0,1,1,1,0,0,1,0,0,0,1,1,1,0,1,1,1,0,0,1,1,0,1,0,1,1,0,0,1,1,0,0,0,0,0,0,0,0,1,1,1,1,1,0,1,0,0,0,0,0,1,1,1,0,1,1,0,1,1,1,0,1,1,0,1,0,1,1,0,0,1,0,1,0,1,1,1,0,1,1,1,1,0,0,0,0,1,0,0,0,1,0,0,1,1,0,1,0,0,1,1,1,1,0,1,1,1,0,1,1,0,0,1,0,1,1,0,0,1,1,0,1,0,0,1,1,1,1,0,1,1,1,0,1,1,0,0,1,0,1,1,1,1,0,0,1,0,1,0,1,1,1,0,1,1,1,1,0,0,0,0,1,0,0,0,1,1,1,1,1,0,0,0,0,0,1,1,1,0,1,1,0,1,1,1,0,1,1,0,1,0,1,0,0,0,0,1,1,0,1,1,0,0,1,1,0,0,0,0,0,0,0,0,1,1,1,1,1,0,0,0,1,1,0,0,0,1,1,1,0,0,1,0,0,0,1,1,1,0,1,1,1,0,0,1,1,0,1,1,0,0,0,0,1,1,0,0,1,0,1,0,1,1,0,0,0,1,0,0,0,0,0,0,1,0,0,1,1,0,1,0,0,1,0,1,1,0,0,0,0,0,1,0,1,1,1,1,0,0,0,1,1,1,0,1,1,0,1,1,1,0,1,1,0,1,1,1,0,1,1,0,1,1,1,0,1,0,0,0,1,0,0,1,1,0,1,1,1,1,0,1,1,0,1,1,0,1,1,0,1,1,1,0,1,1,0,1,0,1,1,0,1,1,1,0,1,1,0,0,1,0,0,0,1,0,0,0,0,0,0,1,0,0,0,1,0,0,0,1,0,1,0,0,0,0,0,0,1,0,0,1,0,0,0,1,0,1,0,1,0,1,1,0,1,0,1,0,1,0,0,0,1,1,0,1,0,1,0,0,1,0,0,0,1,1,0,1,1,1,1,0,1,0,1,1,1,1,1,1,0,1,0,1,1,1,1,0,1,1,0,0,0,0,1,1,0,1,0,1,1,1,1,0,1,1,1,0,1,0,1,1,1,1,1,1,0,1,0,1,1,1,0,1,1,0,1,1,0,1,0,0,1,0,0,0,1,1,1,1,0,0,0,0,0,0,0,0,1,0,0,1,0,0,0,0,0,0,0,0,1,1,1,0,0,1,1,1,1,1,1,0,0,0,1,1,1,0,1,1,0,0,0,1,0,1,1,1,1,1,1,0,1,0,0,0,1,1,0,1,1,1,0,0,0,0,0,0,0,0,0,0,0,0,0,0,0,0,1,1,0,1,1,0,1,0,1,1,0,1,0,1,1,0,1,1,0,0,0,0,0,0,0,0,0,1,1,1,1,1,0,0,0,0,0,1,0,0,1,0,1,0,1,0,0,1,1,1,1,0,0,1,0,1,0,1,0,0,1,0,0,0,0,1,1,1,0,0,0,1,1,0,0,0,0,0,0,1,0,0,0,1,0,0,0,1,1,1,1,1,1,0,0,0,1,0,0,0,1,0,0,0,0,0,0,0,0,0,0,1,0,1,1,1,1,0,1,1,1,0,0,1,0,1,0,0,1,1,1,0,0,1,1,1,0,0,1,0,1,0,0,1,1,1,0,1,1,1,1,0,1,1,0,0,1,1,1,1,0,1,0,1,0,0,1,1,1,1,0,1,1,0,0,0,0,1,1,0,1,1,1,1,0,0,1,0,1,0,1,1,1,1,0,0,1,1,0,0,0,0,0,1,0,1,0,0,1,0,0,0,0,1,1,0,0,1,1,1,1,0,0,1,1,0,0,0,0,1,0,0,1,0,1,0,0,0,0,0,0,1,0,0,0,0,1,0,1,0,1,1,0,0,1,1,1,1,0,0,0,0,0,0,0,0,0,0,0,0,1,1,1,1,0,0,1,1,0,1,0,1,0,0,0,1,0,0,0,0,1,1,0,0,1,0,1,0,0,1,0,0,1,0,1,0,1,0,1,1,1,1,0,1,0,1,0,1,0,0,1,0,0,1,0,1,0,0,1,1,0,0,1,1,1,0,1,1,1,0,1,0,0,1,1,0,0,1,1,1,0,0,1,1,0,0,1,1,0,0,1,1,0,0,1,1,1,0,0,1,1,0,0,1,0,1,1,1,0,1,1,1,1,0,0,0,0,0,1,0,0,0,1,1,1,0,1,0,0,1,1,0,0,0,0,0,0,0,0,1,1,0,0,1,0,1,1,1,0,0,0,1,0,0,0,0,0,1,1,1,1,1,1,0,0,1,0,1,0,0,0,0,1,1,0,0,1,0,0,1,1,1,1,0,0,1,1,1,1,0,0,1,0,0,1,1,0,0,0,0,1,0,1,0,0,1,1,1,1]  distributed_mem=Distributed memory  rst=off  init_reg=0  en=off  latency=0  gui_display_data_type=Boolean  arith_type=Boolean  n_bits=2  bin_pt=0  preci_type=Double  exp_width=8  frac_width=24  optimize=Area  use_rpm=on  simulation_type=fast_sim  XmcBlockStatus=1  maskContainerNames=tabcontainer1  block_type=sprom  block_config=sysgen:SPROM_config
  ROM25 : hdlBasic/ROM  depth=1275  initVector=[0,0,1,0,0,1,0,1,1,0,1,0,0,0,1,0,1,1,1,1,1,0,1,0,1,1,0,0,1,1,0,0,0,1,0,1,1,1,1,0,1,1,0,1,0,1,1,1,0,0,0,0,1,0,0,1,1,0,1,1,0,1,0,0,1,1,1,0,0,0,0,0,0,1,0,0,1,0,1,0,1,1,1,0,1,1,0,0,1,1,1,1,0,0,1,1,0,1,1,1,0,0,0,0,1,1,1,0,1,1,1,0,1,0,1,0,1,0,1,0,0,0,0,1,0,1,1,0,1,1,0,1,0,0,0,1,1,0,1,0,1,0,1,1,0,1,0,0,0,1,0,1,1,1,1,0,0,0,0,0,1,0,1,0,1,1,1,0,0,1,0,0,1,1,1,1,0,0,1,0,0,1,1,0,0,0,1,0,0,1,1,0,0,1,1,0,0,0,1,0,0,1,1,1,1,0,0,0,0,0,0,1,0,0,0,1,1,0,1,1,0,1,1,0,1,1,0,0,1,0,0,1,1,0,1,1,1,1,0,0,1,0,1,1,1,1,0,1,0,1,1,1,1,0,1,0,1,1,0,1,1,1,0,0,1,1,0,0,0,0,1,0,0,1,0,0,0,0,0,1,0,0,0,1,1,1,1,0,0,0,0,0,1,0,1,1,1,1,0,0,1,1,1,1,1,1,0,0,1,0,0,0,1,1,1,1,0,0,1,1,0,0,0,1,1,1,1,1,1,1,1,0,0,1,0,0,0,1,1,1,1,0,0,1,1,0,0,0,1,1,1,0,0,0,1,0,0,0,1,1,1,1,0,0,0,0,0,1,0,1,1,1,1,0,0,1,1,0,0,1,0,1,1,0,1,1,1,0,0,1,1,0,0,0,0,1,0,0,1,0,0,0,0,0,0,0,1,1,0,1,1,1,1,0,0,1,0,1,1,1,1,0,1,0,1,1,1,1,0,1,0,0,1,0,1,0,1,0,0,0,1,1,0,1,1,0,1,1,0,1,1,0,0,1,0,0,1,1,1,0,0,1,1,1,0,1,0,0,1,1,0,0,0,1,0,0,1,1,1,1,0,0,0,0,0,0,1,0,1,1,1,1,0,1,0,0,0,1,1,1,1,0,0,1,0,0,1,1,0,0,0,1,0,0,1,0,1,1,0,1,1,1,1,0,1,1,0,1,1,1,0,0,0,0,0,1,0,1,0,1,1,1,0,0,1,0,0,0,0,0,1,0,0,0,0,1,0,0,0,0,0,1,0,1,0,1,0,1,1,0,1,0,0,0,1,0,1,1,1,0,0,0,1,0,1,0,0,1,0,1,0,0,0,1,1,0,0,0,1,0,1,1,0,1,1,0,1,0,0,0,1,1,0,1,0,1,0,0,0,1,1,0,0,0,1,0,1,0,1,1,1,1,0,1,1,1,0,1,0,1,0,1,0,1,0,0,0,0,0,1,1,1,0,0,1,1,0,0,1,1,1,0,0,0,0,0,1,0,0,1,1,0,1,1,1,0,0,0,0,1,1,0,1,1,0,1,0,1,0,0,1,1,0,0,1,0,1,0,1,1,0,1,1,1,0,1,1,1,0,1,1,0,0,1,1,1,0,0,0,0,1,0,1,1,1,1,0,1,1,0,1,1,1,1,0,1,0,0,0,0,1,1,0,0,0,0,0,0,1,0,0,1,0,1,0,1,1,0,1,1,1,1,1,1,0,0,0,0,1,1,1,1,1,1,0,1,1,0,1,0,1,1,0,1,1,0,1,0,0,1,1,1,1,0,0,0,0,0,1,0,0,0,0,1,0,0,1,0,0,0,0,1,0,0,0,0,0,1,1,1,1,1,1,0,0,0,0,1,0,0,1,0,0,0,1,1,1,1,0,0,1,1,0,1,0,0,1,0,1,1,0,0,1,1,1,1,0,0,0,1,0,1,1,1,0,1,1,0,1,0,0,0,0,0,1,0,1,0,0,0,1,1,0,1,1,1,1,1,1,0,1,1,0,0,0,1,0,1,0,0,0,0,0,1,1,0,0,0,1,0,1,1,1,0,1,1,1,1,0,1,1,1,0,0,0,1,1,0,0,1,1,0,0,0,1,1,1,0,1,1,1,1,0,1,1,1,0,1,0,1,1,0,0,0,0,0,1,0,1,1,0,1,1,0,0,0,1,1,1,0,0,0,0,1,1,1,0,0,0,1,1,0,1,1,0,1,0,0,0,0,0,1,1,1,1,1,0,1,1,0,0,0,0,0,1,1,0,0,0,0,1,1,0,0,1,1,0,0,1,1,0,0,0,0,1,1,0,0,0,0,0,1,1,0,1,1,0,0,0,1,1,1,0,1,0,1,0,1,1,1,0,1,0,1,1,0,1,1,0,1,1,0,1,1,0,1,1,0,1,0,1,1,1,0,1,0,1,0,1,1,1,0,1,1,0,0,1,1,0,0,0,1,0,1,1,1,1,0,0,1,1,0,1,1,1,1,1,1,1,1,0,1,1,0,0,1,1,1,1,0,1,0,0,0,1,1,0,0,0,0,1,1,0,1,0,0,1,1,0,0,1,0,0,0,1,0,1,0,0,0,0,0,1,1,0,0,0,0,0,1,0,1,0,0,0,1,0,0,1,1,0,0,1,0,1,1,0,1,0,1,0,1,1,1,1,1,1,0,0,0,1,0,0,1,1,0,1,1,1,0,1,1,0,1,1,1,0,1,1,0,0,1,0,0,0,1,1,1,1,1,1,0,1,0,1,0,0,0,0,1,0,0,1,1,1,1,1,1,1,1,0,1,1,0,1,0,1,0,0,1,1,0,0,1,0,1,0,1,1,0,1,1,1,1,1,1,1,1,0,0,1,0,0,0,0]  distributed_mem=Distributed memory  rst=off  init_reg=0  en=off  latency=0  gui_display_data_type=Boolean  arith_type=Boolean  n_bits=2  bin_pt=0  preci_type=Double  exp_width=8  frac_width=24  optimize=Area  use_rpm=on  simulation_type=fast_sim  XmcBlockStatus=1  maskContainerNames=tabcontainer1  block_type=sprom  block_config=sysgen:SPROM_config
  ROM26 : hdlBasic/ROM  depth=1275  initVector=[0,0,0,1,0,1,0,1,1,1,0,1,0,1,0,0,0,0,1,0,1,0,1,1,1,0,1,1,0,1,1,0,1,0,1,0,0,0,0,0,1,0,0,0,0,0,0,1,0,0,0,1,1,1,1,1,0,1,0,0,0,1,0,0,0,1,1,0,0,1,1,0,1,1,1,0,1,0,0,1,0,1,0,0,0,1,1,0,0,0,0,1,1,0,0,1,1,0,1,0,1,0,0,1,1,0,0,0,1,1,0,1,1,1,0,1,1,0,0,0,1,0,1,1,0,0,0,0,0,1,0,1,0,0,1,0,0,1,0,0,0,1,0,0,0,0,0,1,0,0,1,1,1,0,1,0,1,1,1,1,0,1,0,0,0,0,0,0,1,0,1,0,0,1,1,1,0,1,1,0,0,0,0,0,1,1,1,0,0,0,0,1,0,0,0,0,1,0,1,1,0,0,0,1,0,0,1,0,0,0,0,1,1,0,0,1,0,1,1,1,1,1,1,1,0,0,1,1,0,1,1,0,1,1,0,0,1,1,0,1,0,0,0,1,1,1,1,0,1,1,1,0,0,1,0,1,0,0,0,1,0,0,0,1,0,1,0,1,1,1,0,1,0,0,1,0,1,1,1,0,0,1,0,0,0,0,0,1,0,1,1,1,0,1,0,0,0,0,0,1,0,1,0,1,1,0,0,0,1,0,0,1,0,1,0,0,0,1,1,0,1,0,0,0,1,0,1,0,1,1,0,0,0,1,0,0,1,0,1,0,0,0,1,1,0,1,0,0,0,1,1,1,1,1,0,0,1,0,0,0,0,0,1,0,1,1,1,0,1,0,0,0,0,0,1,0,0,1,1,0,1,0,0,0,1,0,0,0,1,0,1,0,1,1,1,0,1,0,0,1,0,0,0,0,0,0,0,1,1,0,0,1,1,0,1,0,0,0,1,1,1,1,0,1,1,1,0,0,1,0,0,0,0,1,0,0,1,1,0,0,1,0,1,1,1,1,1,1,1,0,0,1,1,0,1,1,0,0,0,1,1,0,0,0,1,0,1,0,0,0,0,1,0,1,1,0,0,0,1,0,0,1,0,0,0,1,1,0,0,0,0,0,0,1,1,0,0,0,1,1,1,0,1,1,0,0,0,0,0,1,1,1,0,0,0,0,0,1,1,0,1,1,0,1,1,0,0,0,0,1,0,1,1,1,1,0,1,0,0,0,0,0,0,1,0,1,0,0,1,1,0,1,1,1,1,0,1,1,0,0,1,0,1,0,0,0,1,0,0,0,0,0,1,0,0,1,1,1,0,0,1,1,0,1,0,0,0,0,1,0,1,1,0,0,1,1,0,1,1,0,0,0,0,0,1,0,1,0,0,1,0,1,1,1,0,0,1,1,1,0,0,1,1,1,0,0,1,1,1,0,0,0,0,1,1,0,1,1,1,0,1,1,0,0,0,1,1,0,1,0,0,1,1,1,0,0,1,1,1,0,0,1,0,1,1,0,1,1,0,0,1,1,0,1,0,1,0,0,1,1,0,0,0,0,1,1,1,1,0,1,1,1,1,0,1,1,1,1,0,0,0,0,1,0,1,0,1,0,0,0,1,1,0,0,0,0,1,0,0,0,0,0,0,1,1,1,0,0,0,0,1,1,1,0,0,0,0,0,0,1,0,1,0,0,1,1,0,1,1,1,0,1,0,0,0,1,1,1,0,0,0,1,0,0,1,1,1,1,0,0,1,0,0,0,1,1,1,0,0,0,1,0,1,0,0,0,1,0,0,0,1,1,0,0,1,0,0,0,0,0,1,0,1,0,0,0,0,1,0,1,0,0,0,0,0,1,0,0,1,1,0,0,1,0,0,0,1,1,1,1,0,0,0,1,0,1,0,0,0,1,1,0,0,0,0,0,0,0,0,1,1,0,0,0,1,0,1,0,0,0,1,0,0,0,0,1,0,0,0,0,1,0,1,1,0,1,0,0,1,0,1,1,1,0,0,1,1,0,0,1,1,1,0,1,0,0,1,0,1,1,0,1,0,0,1,1,0,1,0,1,0,0,1,0,1,1,1,1,0,0,0,1,0,1,0,0,0,0,0,0,0,0,1,0,1,0,0,0,1,1,1,1,0,1,0,0,0,1,1,1,0,1,1,1,0,1,1,1,0,0,1,0,0,1,1,1,0,1,1,0,0,0,0,1,1,0,1,1,1,0,0,1,0,0,1,1,1,0,1,1,0,0,0,1,0,1,1,0,0,0,0,0,0,1,0,0,1,1,0,0,1,1,0,1,0,0,1,0,1,1,0,0,1,1,0,0,1,0,0,0,0,0,0,1,1,0,1,0,1,0,0,0,1,1,0,0,1,0,1,1,0,0,1,1,0,0,0,0,0,1,1,0,0,0,0,0,1,1,0,0,1,1,0,1,0,0,1,1,0,0,0,0,1,1,1,1,1,1,0,0,0,0,1,1,0,1,1,0,1,1,0,0,0,0,0,1,1,0,0,0,0,0,1,1,0,1,1,0,1,1,0,0,0,0,1,1,1,1,1,0,1,1,0,0,1,1,0,1,1,0,0,0,0,1,0,0,1,0,1,1,1,1,0,0,1,1,1,1,0,1,0,0,1,0,0,0,0,1,1,0,1,1,0,0,1,1,0,0,0,1,1,0,1,1,0,0,0,0,1,1,0,0,1,1,0,1,1,1,0,1,1,1,1,0,1,1,1,0,1,1,0,0,1,1,0,0,0,0,1,1,0,1,1,0,0,0,0,1,0,0,0,0,0,0,0,1,1,0,1,0,1,0,0,0,0,0,0,1,1,0,0,1,1,0,0,0,0,0,0,1,0,1,0,1,1,0,0,0,0,0,0,0,1,0,0]  distributed_mem=Distributed memory  rst=off  init_reg=0  en=off  latency=0  gui_display_data_type=Boolean  arith_type=Boolean  n_bits=2  bin_pt=0  preci_type=Double  exp_width=8  frac_width=24  optimize=Area  use_rpm=on  simulation_type=fast_sim  XmcBlockStatus=1  maskContainerNames=tabcontainer1  block_type=sprom  block_config=sysgen:SPROM_config
  ROM27 : hdlBasic/ROM  depth=1275  initVector=[1,0,0,0,0,1,0,1,1,0,1,1,0,0,1,0,0,0,0,1,1,1,0,0,0,1,0,0,1,0,0,1,0,1,1,1,1,0,0,1,1,1,1,0,0,1,1,0,1,1,0,1,0,0,1,1,1,0,1,1,0,0,1,0,0,0,1,1,0,1,1,1,0,1,1,0,1,1,1,0,1,0,1,0,1,1,1,1,0,0,0,1,0,0,1,0,0,1,1,1,1,0,1,1,0,0,1,1,0,0,0,0,0,1,0,1,1,0,1,1,1,0,1,0,1,0,0,1,0,0,1,1,0,0,0,0,1,1,0,0,1,0,0,1,0,0,1,1,0,1,1,0,1,1,1,1,0,1,1,1,0,0,1,0,0,0,0,1,0,0,0,0,1,0,1,1,0,1,0,1,1,0,1,1,0,0,0,1,1,1,1,1,0,1,0,0,1,0,1,0,0,0,1,0,0,0,1,1,1,0,0,0,1,0,1,0,0,1,1,0,0,1,1,0,0,0,1,0,1,1,1,1,1,0,1,0,1,1,1,0,0,0,0,0,1,0,1,1,1,0,0,1,1,0,0,0,1,1,0,0,0,1,0,1,0,0,1,1,0,0,1,1,0,0,1,0,1,0,0,1,0,1,0,0,0,1,0,0,1,1,0,1,0,1,0,1,1,0,0,1,1,0,0,1,0,1,0,0,1,0,1,1,0,0,0,0,1,1,0,0,1,0,1,0,0,1,0,0,1,0,1,0,0,1,0,1,1,0,0,0,0,1,1,0,0,1,0,1,0,0,0,1,0,0,1,0,1,0,0,0,1,0,0,1,1,0,1,0,1,0,1,1,0,0,1,0,0,1,0,0,0,1,1,0,0,0,1,0,1,0,0,1,1,0,0,1,1,0,0,1,0,0,1,1,0,0,1,1,0,1,0,1,1,1,0,0,0,0,0,1,0,1,1,1,0,0,1,1,1,0,0,0,0,1,1,0,0,1,0,1,0,0,1,1,0,0,1,1,0,0,0,1,0,1,1,1,1,0,1,1,1,1,0,1,1,1,1,0,1,0,0,1,0,1,0,0,0,1,0,0,0,1,1,1,0,1,0,0,1,0,0,1,0,0,1,0,0,1,0,1,1,0,1,0,1,1,0,1,1,0,0,0,1,1,1,1,1,0,1,0,0,0,0,1,0,1,1,1,1,1,1,0,1,1,1,0,0,1,0,0,0,0,1,0,0,0,1,1,0,1,1,1,1,1,1,1,1,0,1,1,0,1,1,0,0,1,0,0,1,0,0,1,1,0,1,1,0,1,0,1,1,1,1,0,0,1,1,0,0,1,1,1,1,0,1,1,0,1,0,1,0,0,1,0,0,1,1,0,0,0,0,0,0,0,0,0,1,0,1,0,0,1,0,1,0,0,0,0,0,0,0,1,1,0,0,0,0,0,1,0,1,1,0,1,1,0,1,1,0,0,0,0,1,0,0,0,0,1,0,0,0,0,1,1,0,1,1,0,0,1,0,0,1,1,1,1,0,1,1,0,1,0,1,0,0,0,0,1,1,1,0,0,1,1,1,0,0,0,0,1,0,1,0,1,0,1,0,1,0,1,1,1,1,0,0,0,1,0,0,0,0,1,1,1,0,0,1,0,0,1,0,0,1,1,1,0,0,0,0,1,0,1,1,0,1,1,1,0,1,1,0,1,1,0,1,1,1,1,0,1,0,1,0,0,0,1,1,0,0,0,1,0,1,0,1,1,1,1,0,1,1,1,0,1,1,0,0,1,0,0,0,1,0,0,1,1,1,0,0,0,0,0,1,0,1,1,0,1,0,0,0,0,0,1,1,1,0,0,1,0,1,1,0,1,1,0,1,0,0,1,0,0,1,1,0,0,0,1,1,0,0,0,0,1,0,0,1,0,0,0,0,1,1,0,0,0,1,1,0,0,1,1,0,0,1,1,1,1,0,0,0,0,1,1,1,1,0,0,0,1,1,1,0,1,0,1,1,0,1,0,1,1,1,0,0,0,1,1,1,1,0,0,0,1,0,0,1,0,1,1,1,0,0,1,1,1,1,0,1,1,0,0,0,1,1,0,0,0,0,0,0,1,1,0,0,0,1,1,0,1,1,1,1,0,0,1,1,0,0,0,1,0,0,1,1,1,0,0,1,1,0,0,0,1,1,1,0,1,0,0,0,0,0,0,1,0,1,1,1,0,0,0,1,1,0,0,1,1,1,0,0,0,0,0,1,1,0,1,1,0,0,1,0,0,0,0,0,1,0,0,0,1,0,1,1,1,1,0,1,0,0,0,1,0,0,0,0,0,1,0,0,1,1,0,1,1,1,0,0,1,1,1,0,1,1,1,1,1,0,0,1,1,1,1,0,1,0,1,0,0,0,0,1,0,1,0,1,1,1,1,0,0,1,1,1,1,1,0,1,1,1,0,1,1,0,0,0,0,1,1,1,1,1,0,1,0,0,0,0,1,1,0,1,1,1,1,1,1,1,1,0,1,1,0,0,0,0,1,0,1,1,1,1,1,0,0,0,0,0,0,1,1,0,0,0,0,0,0,0,0,1,0,1,1,0,1,0,0,1,0,0,0,0,0,0,0,0,1,0,0,1,0,1,1,0,1,0,0,0,0,0,0,0,0,1,1,0,0,0,1,1,0,0,0,0,1,1,1,0,0,1,0,1,1,1,1,0,1,0,0,0,0,0,0,1,0,1,1,1,1,0,1,0,0,1,1,1,0,0,0,0,1,1,0,0,1,0,0,0,1,0,1,1,1,1,1,1,1,1,0,1,1,1,0,1,0,1,0,1,1,1,1,0,1,0,1,0,1,1,1,0,1,1,1,1,1,1,1,1,0,1,0,0,0,1]  distributed_mem=Distributed memory  rst=off  init_reg=0  en=off  latency=0  gui_display_data_type=Boolean  arith_type=Boolean  n_bits=2  bin_pt=0  preci_type=Double  exp_width=8  frac_width=24  optimize=Area  use_rpm=on  simulation_type=fast_sim  XmcBlockStatus=1  maskContainerNames=tabcontainer1  block_type=sprom  block_config=sysgen:SPROM_config
  ROM28 : hdlBasic/ROM  depth=1275  initVector=[1,1,0,1,0,0,1,1,1,0,0,0,0,0,0,1,1,1,0,1,1,0,1,0,0,0,0,1,0,0,0,1,0,1,1,1,1,1,1,0,0,0,0,0,1,0,1,0,1,1,1,1,1,0,0,1,0,0,1,1,0,1,0,1,1,0,1,0,0,0,0,0,1,1,1,1,1,0,1,1,1,0,1,1,1,0,1,0,0,0,0,0,1,1,0,1,0,0,1,0,1,0,1,0,1,1,1,0,0,1,0,1,1,1,1,0,1,1,0,1,0,0,1,1,0,0,1,0,1,0,0,1,0,1,1,1,1,1,0,1,0,1,0,1,0,0,1,0,0,0,0,0,1,0,0,0,0,0,1,1,1,1,1,1,1,1,0,0,1,1,0,0,0,0,0,0,1,1,1,1,1,1,1,0,1,0,0,0,1,0,1,1,1,0,1,0,1,0,1,0,0,1,0,0,1,1,1,1,1,0,1,0,1,1,0,1,1,1,1,0,1,0,1,0,0,0,0,1,1,1,0,1,0,0,0,1,1,1,0,1,1,1,1,0,1,0,1,0,0,1,1,0,1,1,1,0,1,0,1,1,0,1,0,0,0,0,1,1,1,0,1,1,1,0,0,1,0,0,0,0,1,1,0,0,1,0,1,1,1,1,0,0,1,1,1,0,0,0,1,1,1,1,1,0,0,0,0,0,1,0,0,0,1,0,0,1,1,0,1,0,1,1,0,0,1,1,1,1,0,0,0,0,0,1,0,0,0,1,0,0,1,1,0,1,0,1,1,0,0,1,1,0,0,0,0,1,1,0,0,1,0,1,1,1,1,0,0,1,1,1,0,0,0,1,1,0,0,1,1,1,0,1,0,1,1,0,1,0,0,0,0,1,1,1,0,1,1,1,0,0,1,1,0,0,1,1,1,0,0,0,1,1,1,0,1,1,1,1,0,1,0,1,0,0,1,1,0,1,0,0,1,1,0,0,1,1,0,1,1,0,1,1,1,1,0,1,0,1,0,0,0,0,1,1,1,0,0,0,0,1,1,0,0,0,0,1,1,1,0,1,0,1,0,1,0,0,1,0,0,1,1,1,1,1,0,1,1,1,0,0,0,0,1,1,1,0,0,0,0,0,0,1,1,1,1,1,1,1,0,1,0,0,0,1,0,1,1,1,1,1,1,1,1,1,1,1,1,0,0,0,0,0,0,1,1,1,1,1,1,1,1,0,0,1,1,0,1,1,1,0,1,1,0,0,1,1,0,1,1,1,0,1,1,0,1,0,1,0,1,0,0,1,0,0,0,0,0,1,1,0,1,0,0,0,1,1,1,1,0,0,0,1,0,1,1,0,0,1,1,0,0,1,0,1,0,0,1,0,1,1,1,0,1,0,1,0,1,1,0,1,1,0,1,1,0,1,0,1,0,1,1,1,0,0,1,0,1,1,1,1,0,1,1,0,1,1,0,0,0,1,0,0,1,0,0,0,0,1,0,0,1,0,0,0,1,1,0,1,1,0,1,0,0,1,0,1,0,1,0,1,0,1,0,0,1,0,0,1,1,1,0,0,1,1,1,0,0,1,0,0,1,0,1,1,1,1,0,1,1,1,0,1,0,0,0,0,0,1,0,0,1,0,0,1,0,0,1,1,1,1,0,0,1,0,0,1,0,0,1,0,0,1,0,0,0,0,0,1,1,1,1,1,0,0,1,1,1,0,1,1,1,0,1,0,1,0,0,1,0,1,0,1,1,1,0,1,1,1,0,0,1,0,0,1,1,0,1,0,1,1,0,1,0,0,0,0,1,1,1,0,1,1,0,1,0,0,1,0,1,1,0,1,1,1,0,0,0,0,1,0,0,1,0,1,1,1,1,1,0,0,1,1,0,1,1,0,0,1,1,0,0,1,0,0,0,0,0,0,1,0,0,1,1,0,0,1,1,0,1,1,0,1,1,1,0,0,0,0,0,1,0,1,1,1,0,1,1,0,1,1,1,1,1,1,1,1,1,1,1,1,1,1,1,1,0,1,1,0,1,1,1,0,1,0,0,0,1,0,1,1,1,0,1,0,1,0,1,1,0,1,1,1,0,1,0,0,0,0,0,0,0,0,1,0,1,1,1,0,1,1,0,1,0,1,0,1,0,1,0,0,0,0,1,1,0,1,1,1,1,0,1,1,0,1,1,1,1,1,1,0,0,0,0,1,1,1,1,1,1,0,1,1,0,1,1,1,1,0,1,1,1,1,1,0,1,1,0,1,0,1,0,0,1,0,0,0,1,1,1,0,1,1,1,1,0,0,1,1,1,1,0,1,1,1,0,0,0,1,0,0,1,0,1,0,1,0,0,0,0,0,1,0,0,0,1,1,0,1,1,1,0,0,0,0,1,0,1,0,1,0,0,1,0,1,0,1,0,0,0,0,1,1,1,0,1,1,0,0,0,1,0,1,1,1,0,0,0,0,1,0,1,1,0,0,0,0,1,1,0,0,0,1,0,1,0,0,0,0,1,0,1,0,0,0,1,1,0,0,0,0,1,1,0,1,0,0,0,0,1,0,0,1,0,1,0,0,1,0,0,0,1,1,0,1,0,0,0,1,1,0,0,0,1,1,0,0,0,1,1,0,0,0,1,0,1,1,0,0,0,1,0,0,1,0,1,0,1,0,0,1,0,1,1,0,1,1,0,0,1,1,1,0,1,0,0,1,0,0,1,0,1,1,0,1,0,0,1,0,0,1,0,1,1,1,0,0,1,1,0,1,1,0,1,0,0,1,1,1,1,0,1,0,0,1,0,1,1,1,0,1,0,1,0,0,1,1,1,1,0,1,1,0,1,1,1,1,0,0,1,0,1,0,1,1,1,0,1,0,0,1,0,1,1,1,1]  distributed_mem=Distributed memory  rst=off  init_reg=0  en=off  latency=0  gui_display_data_type=Boolean  arith_type=Boolean  n_bits=2  bin_pt=0  preci_type=Double  exp_width=8  frac_width=24  optimize=Area  use_rpm=on  simulation_type=fast_sim  XmcBlockStatus=1  maskContainerNames=tabcontainer1  block_type=sprom  block_config=sysgen:SPROM_config
  ROM29 : hdlBasic/ROM  depth=1275  initVector=[0,0,1,1,1,1,0,0,1,0,0,1,0,1,0,1,0,0,0,0,1,1,1,1,0,0,0,1,0,1,0,0,1,1,1,0,0,0,0,0,1,0,1,1,0,0,0,1,1,0,1,0,0,0,1,0,0,0,0,1,0,1,1,0,1,1,0,0,1,1,0,1,0,0,0,0,0,0,0,0,0,0,1,0,0,0,1,0,1,1,0,1,1,0,0,1,0,0,1,0,0,1,1,1,1,1,0,0,1,0,1,0,0,0,1,1,0,0,1,1,1,0,0,1,0,0,1,0,0,0,1,1,0,0,0,0,0,1,1,0,0,0,1,0,1,0,0,0,1,0,1,1,0,0,1,1,1,1,1,1,0,1,0,0,1,0,1,0,0,1,1,0,0,0,0,0,0,1,1,1,0,0,1,0,0,1,0,0,0,1,1,0,0,0,1,0,0,1,1,0,1,0,1,1,1,1,0,0,0,0,1,1,0,0,1,0,0,1,0,0,1,0,0,1,1,0,0,1,1,1,0,0,0,1,0,1,0,1,0,1,0,0,1,0,0,1,0,1,0,1,0,0,1,1,1,0,1,0,0,1,0,1,0,0,1,1,0,1,0,1,1,1,1,1,0,1,0,1,1,0,0,0,1,0,0,1,0,1,0,1,1,0,0,1,1,0,0,0,1,0,0,1,1,0,1,0,1,0,1,1,0,1,1,0,0,1,0,1,0,0,0,1,1,1,0,0,1,1,0,1,0,1,0,1,1,0,1,1,0,0,1,0,1,0,0,0,1,1,1,0,0,0,1,1,0,0,0,1,0,0,1,0,1,0,1,1,0,0,1,1,0,0,0,1,0,1,1,0,1,1,0,1,0,0,1,0,1,0,0,1,1,0,1,0,1,1,1,1,1,0,1,1,1,1,1,1,0,0,1,0,1,0,1,0,1,0,0,1,0,0,1,0,1,0,1,0,0,1,0,0,1,1,0,0,1,1,1,0,0,1,0,0,1,0,0,1,0,0,1,1,0,0,1,1,1,0,0,1,0,0,0,0,1,0,0,1,0,0,0,1,0,0,1,1,0,1,0,1,1,1,1,0,0,0,0,1,0,1,0,0,0,0,1,0,1,0,0,0,0,0,0,0,1,1,1,0,0,1,0,0,1,0,0,0,1,0,1,1,1,1,0,0,1,1,1,1,0,1,0,1,1,1,1,1,1,0,1,0,0,1,0,1,0,0,1,1,0,0,1,0,1,1,1,1,1,1,0,1,0,0,1,0,1,1,0,0,0,1,0,1,0,0,0,1,0,1,1,0,1,0,0,0,1,1,0,0,0,0,1,1,0,0,0,1,0,1,0,0,1,0,0,1,0,0,0,1,1,0,0,0,0,1,0,0,1,0,0,0,0,1,1,0,0,0,0,1,0,0,1,0,1,0,0,1,0,1,0,0,0,1,1,0,0,1,1,0,1,0,1,1,1,1,1,1,0,0,1,1,1,1,1,1,0,1,0,1,1,1,0,0,1,0,0,1,0,0,1,1,1,1,1,0,0,1,0,1,1,0,0,1,0,0,1,0,0,1,1,0,1,0,0,1,1,0,0,0,0,1,0,0,0,1,0,1,1,0,1,0,0,1,0,0,1,0,0,1,0,1,1,0,1,0,0,1,0,0,1,0,0,1,0,0,0,1,1,0,1,0,0,0,0,0,0,1,1,0,1,0,1,1,0,0,1,1,1,1,1,1,1,1,0,0,1,1,0,1,0,1,1,0,0,0,0,0,1,0,1,1,0,1,1,0,1,1,1,1,0,0,0,1,1,0,0,0,0,0,0,0,0,1,1,0,0,0,1,1,1,1,0,1,0,0,1,1,0,1,0,0,0,1,1,0,0,0,1,0,0,0,0,0,0,0,0,1,1,1,1,0,0,0,0,0,0,0,0,1,0,0,0,1,1,0,0,0,0,1,0,1,1,0,0,0,0,1,0,0,0,1,1,1,1,0,1,1,0,1,1,0,1,1,0,1,1,1,1,0,0,0,1,0,0,0,0,0,1,0,0,1,1,1,0,1,0,1,0,0,1,0,0,0,0,1,1,1,0,0,0,0,0,0,0,0,1,1,1,0,0,0,0,1,0,0,1,0,1,0,1,1,1,0,0,0,1,1,1,0,1,0,0,0,0,1,1,1,1,0,0,1,1,1,1,1,1,1,1,0,0,1,1,1,1,0,0,0,0,1,0,1,1,1,1,0,0,0,0,1,0,1,0,1,0,1,0,0,1,0,0,1,0,0,0,0,0,0,0,0,0,0,0,0,0,0,1,0,0,1,0,0,1,0,1,0,1,0,1,0,1,0,1,0,0,0,1,1,0,1,0,1,1,0,0,0,1,0,1,1,1,0,0,1,1,0,0,1,1,1,0,1,0,0,0,1,1,0,1,0,1,1,0,0,0,0,0,1,0,1,0,0,0,0,1,0,1,0,0,1,1,0,1,0,0,0,0,1,0,0,0,0,1,0,0,0,0,1,0,1,1,0,0,1,0,1,0,0,0,0,1,0,1,1,1,1,0,0,1,0,0,1,0,1,0,0,0,0,1,1,0,0,0,1,0,1,1,1,1,0,1,0,0,0,1,1,0,0,0,0,1,0,1,0,0,1,0,0,1,1,0,1,1,0,1,0,1,1,0,0,0,0,0,1,0,0,1,1,0,0,1,0,1,1,1,1,1,1,0,1,0,0,1,1,0,0,1,0,0,0,0,0,1,1,0,1,0,1,1,0,0,1,0,0,1,1,0,0,0,0,0,0,1,1,1,0,0,0,1,1,0,1,0,0,0,0,1,0,1,1,0,0,0,1,1,1,0,0,0,0,0,0,1,1,0,0,1,0,0]  distributed_mem=Distributed memory  rst=off  init_reg=0  en=off  latency=0  gui_display_data_type=Boolean  arith_type=Boolean  n_bits=2  bin_pt=0  preci_type=Double  exp_width=8  frac_width=24  optimize=Area  use_rpm=on  simulation_type=fast_sim  XmcBlockStatus=1  maskContainerNames=tabcontainer1  block_type=sprom  block_config=sysgen:SPROM_config
  ROM3 : hdlBasic/ROM  depth=1275  initVector=[1,1,1,1,1,1,1,1,1,0,1,1,0,0,0,1,0,0,0,0,0,1,0,0,0,0,0,0,0,0,0,0,0,0,0,0,0,0,0,0,0,0,0,1,1,0,0,0,0,0,0,1,1,1,1,0,0,0,0,0,1,1,1,1,1,1,0,0,0,0,0,1,1,1,1,1,1,1,0,0,0,0,1,1,1,1,1,1,1,1,0,0,0,0,1,1,1,1,1,1,1,1,0,0,0,0,0,0,1,1,1,1,1,1,1,0,0,0,0,0,0,0,1,1,1,1,1,1,1,0,0,0,0,0,0,0,0,0,1,1,1,1,1,1,1,0,0,0,0,0,0,0,1,0,0,1,1,1,1,1,1,0,0,0,0,0,0,0,1,1,1,0,1,1,1,1,1,1,1,0,0,0,0,0,0,0,1,1,1,1,0,1,1,1,1,1,1,0,0,0,0,0,0,0,1,1,1,1,1,1,0,1,1,1,1,1,1,0,0,0,0,0,0,0,1,1,1,1,1,1,1,0,1,1,1,1,1,1,0,0,0,0,0,0,1,1,1,1,1,1,1,0,0,0,1,1,1,1,1,1,0,0,0,0,0,0,1,1,1,1,1,1,0,0,0,0,0,1,1,1,1,1,1,0,0,0,0,0,0,1,1,1,1,1,1,0,0,0,0,0,0,1,1,1,1,1,1,0,0,0,0,0,0,1,1,1,1,1,1,0,0,0,0,0,0,0,1,1,1,1,1,1,0,0,0,0,0,0,1,1,1,1,1,1,0,0,0,0,0,0,0,0,1,1,1,1,1,1,0,0,0,0,0,0,1,1,1,1,1,1,0,0,0,0,0,0,0,0,0,1,1,1,1,1,1,0,0,0,0,0,0,1,1,1,1,1,1,0,0,0,0,0,0,0,0,0,0,1,1,1,1,1,1,0,0,0,0,0,0,1,1,1,1,1,1,1,0,0,0,0,0,0,0,0,0,0,1,1,1,1,1,1,0,0,0,0,0,0,0,1,1,1,1,1,1,1,0,0,0,0,0,0,0,0,1,0,1,1,1,1,1,1,0,0,0,0,0,0,0,1,1,1,1,1,1,1,1,0,0,0,0,0,0,1,1,1,0,1,1,1,1,1,1,1,0,0,0,0,0,0,0,1,1,1,1,1,1,1,1,1,1,1,1,1,1,1,1,1,0,0,1,1,1,1,1,1,0,0,0,0,0,0,0,1,1,1,1,1,1,1,1,1,1,1,1,1,1,1,1,1,1,0,0,1,1,1,1,1,1,1,0,0,0,0,0,0,0,1,1,1,1,1,1,1,1,1,1,1,1,1,1,1,1,1,1,0,0,1,1,1,1,1,1,1,0,0,0,0,0,0,0,0,1,1,1,1,1,1,1,1,1,1,1,1,1,1,1,1,0,0,0,0,0,1,1,1,1,1,1,1,0,0,0,0,0,0,0,0,0,1,1,1,1,1,1,1,1,1,1,1,1,0,0,0,0,0,0,0,0,1,1,1,1,1,1,1,1,0,0,0,0,0,0,0,0,0,0,1,1,1,1,1,1,1,1,0,0,0,0,0,0,0,0,0,0,0,0,1,1,1,1,1,1,1,1,0,0,0,0,0,0,0,0,0,0,0,0,0,0,0,0,0,0,0,0,0,0,0,0,0,0,0,0,0,0,0,1,1,1,1,1,1,1,1,0,0,0,0,0,0,0,0,0,0,0,0,0,0,0,0,0,0,0,0,0,0,0,0,1,1,0,0,0,0,0,1,1,1,1,1,1,1,1,1,0,0,0,0,0,0,0,0,0,0,0,0,0,0,0,0,0,0,0,0,0,0,1,1,1,1,0,0,0,0,0,0,1,1,1,1,1,1,1,1,1,0,0,0,0,0,0,0,0,0,0,0,0,0,0,0,0,0,0,0,0,1,1,1,1,1,1,0,0,0,0,0,0,0,1,1,1,1,1,1,1,1,1,1,0,0,0,0,0,0,0,0,0,0,0,0,0,0,0,0,1,1,1,1,1,1,1,1,1,0,0,0,0,0,0,0,0,1,1,1,1,1,1,1,1,1,1,1,0,0,0,0,0,0,0,0,0,0,0,0,1,1,1,1,1,1,1,1,1,1,1,0,1,0,0,0,0,0,0,0,0,1,1,1,1,1,1,1,1,1,1,1,1,1,1,1,1,1,1,1,1,1,1,1,1,1,1,1,1,1,1,1,1,0,0,0,1,0,0,0,0,0,0,0,0,0,1,1,1,1,1,1,1,1,1,1,1,1,1,1,1,1,1,1,1,1,1,1,1,1,1,1,1,1,1,1,0,0,0,0,0,1,1,0,0,0,0,0,0,0,0,0,0,1,1,1,1,1,1,1,1,1,1,1,1,1,1,1,1,1,1,1,1,1,1,1,1,1,1,0,0,0,0,0,0,0,0,1,1,1,0,0,0,0,0,0,0,0,0,0,1,1,1,1,1,1,1,1,1,1,1,1,1,1,1,1,1,1,1,1,1,1,1,1,0,0,0,0,0,0,0,0,0,0,1,1,1,1,0,0,0,0,0,0,0,0,0,0,0,1,1,1,1,1,1,1,1,1,1,1,1,1,1,1,1,1,1,1,1,0,0,0,0,0,0,0,0,0,0,0,1,1,1,1,1,1,1,0,0,0,0,0,0,0,0,0,0,0,0,0,1,1,1,1,1,1,1,1,1,1,1,1,1,1,0,0,0,0,0,0,0,0,0,0,0,0,0,1,1,1,1,1,1,1,1,1,1,1,0,0,0,0,0,0,0,0,0,0,0,0,0,0,0,0,0,0,0,0,0,0,0,0,0,0,0,0,0,0,0,0,0,0,0,0,1,1,1,1,1,1,1]  distributed_mem=Distributed memory  rst=off  init_reg=0  en=off  latency=0  gui_display_data_type=Boolean  arith_type=Boolean  n_bits=2  bin_pt=0  preci_type=Double  exp_width=8  frac_width=24  optimize=Area  use_rpm=on  simulation_type=fast_sim  XmcBlockStatus=1  maskContainerNames=tabcontainer1  block_type=sprom  block_config=sysgen:SPROM_config
  ROM30 : hdlBasic/ROM  depth=1275  initVector=[0,0,1,1,0,0,0,1,0,1,0,0,1,0,0,0,0,1,0,0,1,1,0,1,0,0,0,0,1,1,0,1,1,0,1,1,1,0,1,1,1,1,1,0,0,0,1,0,1,1,1,0,0,1,1,0,0,1,1,0,1,1,1,0,1,0,1,1,1,0,0,0,1,1,0,0,0,1,0,0,0,1,0,1,1,1,0,0,0,0,0,0,0,0,1,1,1,1,0,1,0,1,1,0,1,0,0,1,0,0,1,0,0,0,0,1,1,0,0,0,1,1,1,1,0,0,1,0,0,0,1,0,0,0,0,1,1,0,0,1,1,0,1,1,1,0,0,1,1,1,0,1,0,1,1,0,1,1,1,1,0,1,0,0,1,1,1,0,1,1,1,1,1,1,1,1,0,0,1,1,0,1,1,1,1,1,1,0,0,0,0,0,1,1,1,0,0,0,1,0,0,1,1,1,1,0,0,0,1,1,1,0,0,0,1,1,0,0,1,0,0,1,1,1,0,0,0,0,0,0,0,1,0,1,1,1,0,1,0,1,1,0,1,1,0,1,0,0,0,0,0,1,1,1,1,1,0,1,1,1,0,1,0,1,1,1,0,1,1,0,0,1,1,0,0,0,0,0,1,0,0,0,1,0,1,0,1,1,0,1,1,0,0,0,1,1,0,0,1,1,1,1,1,1,0,1,1,1,0,0,1,0,0,1,0,0,1,1,0,1,1,0,0,0,0,1,1,1,1,0,1,1,1,0,0,1,0,0,1,0,0,1,1,0,1,1,0,0,0,0,0,0,0,1,0,0,0,1,0,1,0,1,1,0,1,1,0,0,0,1,1,0,0,1,1,0,0,1,1,1,1,0,1,1,1,0,1,0,1,1,1,0,1,1,0,0,1,1,0,0,0,1,0,0,1,0,1,0,1,1,1,0,1,0,1,1,0,1,1,0,1,0,0,0,0,0,1,1,0,0,0,0,0,0,1,1,0,0,0,1,1,0,0,1,0,0,1,1,1,0,0,0,0,0,0,0,1,0,0,1,1,0,0,1,0,0,0,1,1,1,0,0,0,1,0,0,1,1,1,1,0,0,0,1,1,0,0,1,1,1,1,1,1,0,0,1,1,1,1,1,1,0,0,1,1,0,1,1,1,1,1,1,0,0,0,1,0,0,1,1,0,0,1,1,0,0,1,0,1,1,0,1,1,1,1,0,1,0,0,1,1,1,0,1,1,1,0,0,0,0,0,0,1,1,0,0,0,0,0,0,1,1,0,0,1,1,0,1,1,1,0,0,1,1,1,0,1,0,1,0,0,0,0,0,0,1,1,0,0,0,0,0,0,1,0,1,1,1,1,0,0,1,0,0,0,1,0,0,0,0,1,1,1,1,0,0,0,1,0,0,0,0,1,0,0,0,1,1,1,1,0,0,1,0,0,1,0,0,0,0,1,1,0,0,0,0,0,0,1,1,0,1,1,1,0,0,1,1,1,0,1,1,0,0,0,0,0,0,0,1,1,1,1,0,1,0,1,1,0,1,0,0,1,1,1,1,1,0,0,1,1,1,1,0,0,1,1,1,1,1,0,0,1,0,0,0,1,0,1,1,1,0,0,0,0,0,0,0,0,1,1,1,1,1,1,1,0,0,0,0,1,1,1,1,1,1,1,0,0,0,0,1,1,1,0,0,0,1,1,0,0,0,1,0,1,1,0,1,1,1,1,1,1,1,1,0,0,1,1,1,1,1,1,1,1,0,1,1,0,1,0,0,1,1,0,1,1,1,0,1,0,0,0,1,1,1,0,0,1,0,0,0,1,1,1,1,1,1,0,0,0,1,0,0,1,1,1,0,0,0,0,1,0,1,1,1,0,0,1,1,1,0,0,0,0,0,0,0,0,0,0,1,0,0,0,0,0,0,1,0,0,0,0,0,0,0,0,0,0,1,1,1,0,1,1,1,1,1,0,0,1,0,0,0,1,0,0,1,1,1,1,1,1,1,1,0,0,1,1,1,1,1,1,1,1,0,0,1,0,0,0,1,0,1,1,0,1,1,0,1,1,0,0,1,1,1,0,0,0,1,0,1,0,0,0,0,0,1,1,0,0,0,0,0,1,0,1,0,0,0,1,1,1,0,0,1,1,0,1,0,0,0,0,1,1,0,1,1,1,1,0,1,1,1,0,0,0,1,1,1,1,1,1,1,1,0,0,0,1,1,1,0,1,1,1,1,0,1,1,0,0,0,1,0,0,1,0,0,1,1,1,0,1,1,1,0,0,1,0,0,1,0,1,0,1,1,0,1,0,1,0,0,1,0,0,1,1,1,0,1,1,1,0,0,1,0,0,1,0,0,0,0,1,1,1,0,0,0,1,0,0,1,1,1,1,1,1,1,0,0,0,0,1,1,1,1,1,1,1,0,0,1,0,0,0,1,1,1,0,0,0,0,1,0,1,0,0,0,1,1,1,1,0,1,1,0,1,1,1,1,1,0,1,0,0,1,1,0,0,1,0,1,1,1,1,1,0,1,1,0,1,1,1,1,0,0,0,1,1,0,0,0,1,1,1,0,1,0,1,1,0,0,1,1,0,0,1,1,0,1,1,1,1,1,1,1,1,0,1,1,0,0,1,1,0,0,1,1,0,1,0,1,1,1,0,0,0,1,0,1,0,0,0,1,0,1,0,1,0,0,0,1,0,1,1,0,0,0,1,0,1,1,0,1,0,0,0,1,1,0,1,0,0,0,1,0,1,0,1,0,0,0,1,0,1,0,0,1,0,0,0,1,1,1,0,0,1,0,0,0,1,1,1,1,0,1,1,1,0,1,1,0,1,1,1,0,1,1,1,1,0,0,0,1,0,0,1,1,1,0,0,0,1,0,0]  distributed_mem=Distributed memory  rst=off  init_reg=0  en=off  latency=0  gui_display_data_type=Boolean  arith_type=Boolean  n_bits=2  bin_pt=0  preci_type=Double  exp_width=8  frac_width=24  optimize=Area  use_rpm=on  simulation_type=fast_sim  XmcBlockStatus=1  maskContainerNames=tabcontainer1  block_type=sprom  block_config=sysgen:SPROM_config
  ROM31 : hdlBasic/ROM  depth=1275  initVector=[1,0,1,0,0,1,1,0,0,1,0,1,1,0,1,1,1,0,1,0,1,0,1,1,0,0,0,1,1,1,0,1,1,0,1,1,1,0,0,1,1,1,0,0,1,1,0,1,0,0,1,1,1,0,1,0,0,0,1,0,0,0,1,1,1,1,1,1,0,0,1,1,0,0,1,1,1,1,0,1,0,0,1,1,1,0,1,0,0,0,1,1,1,1,0,0,0,1,1,1,1,1,1,1,1,0,0,1,0,0,1,1,0,0,1,0,0,1,0,1,0,0,1,0,0,1,1,0,1,1,0,1,0,0,1,1,1,0,0,1,1,1,0,1,1,1,1,1,0,1,1,0,1,0,0,1,1,0,0,1,1,1,1,1,0,0,0,1,1,1,1,0,0,1,0,0,1,0,1,1,1,1,0,0,1,1,1,1,0,1,0,1,1,1,1,0,1,1,0,1,1,0,0,0,0,0,1,0,1,1,1,0,1,1,0,0,1,1,0,1,1,1,1,1,1,0,0,0,0,1,1,1,0,1,1,1,1,0,0,1,1,0,1,1,1,1,1,1,1,1,0,1,1,1,0,0,0,0,1,1,1,0,0,0,0,0,1,0,0,1,0,1,1,0,0,1,1,1,0,0,1,0,1,0,0,0,0,0,0,1,1,0,1,1,0,1,1,1,0,1,1,0,1,0,1,0,1,0,1,1,0,1,0,1,0,0,1,1,0,1,0,1,0,1,1,1,0,1,0,1,0,1,0,1,1,0,1,0,1,0,0,1,1,0,1,0,1,0,1,1,1,1,1,0,0,1,0,1,0,0,0,0,0,0,1,1,0,1,1,0,1,1,1,0,1,1,1,1,1,0,0,0,0,1,1,1,0,0,0,0,0,1,0,0,1,0,1,1,0,0,1,0,0,0,0,1,1,0,1,1,1,1,0,0,1,1,0,1,1,1,1,1,1,1,1,0,1,1,0,1,1,1,1,0,1,1,0,1,1,0,0,1,1,0,1,1,1,1,1,1,0,0,0,0,1,1,1,0,1,0,0,1,0,1,1,0,1,1,1,1,0,1,1,0,1,1,0,0,0,0,0,1,0,1,1,1,0,1,1,1,1,1,1,0,1,1,0,0,1,0,0,1,0,1,1,1,1,0,0,1,1,1,1,0,1,1,0,1,1,0,0,0,0,1,1,0,1,1,0,0,1,1,0,0,1,1,1,1,1,0,0,0,1,1,1,1,0,0,0,1,0,1,1,1,1,0,1,0,0,0,1,1,0,0,1,1,1,0,1,1,1,1,1,0,1,1,0,1,1,1,1,0,1,1,1,1,1,1,1,1,0,1,1,1,1,0,0,1,0,0,1,1,0,1,1,0,1,0,0,1,1,0,1,1,0,0,1,0,0,0,0,0,0,1,0,0,1,1,0,1,0,0,1,0,0,1,1,0,0,1,0,0,1,0,1,1,1,1,1,0,1,1,0,1,0,0,1,0,1,1,0,1,1,1,1,1,1,1,1,0,0,0,1,1,1,1,1,1,1,1,0,0,1,0,1,0,1,1,1,1,1,1,1,1,1,1,0,1,0,1,0,0,1,0,1,0,0,1,1,1,0,1,0,0,0,1,1,1,0,0,0,0,0,1,1,0,0,0,0,0,0,1,1,0,0,0,0,0,1,1,1,1,1,0,0,1,1,0,0,1,1,1,1,0,1,0,1,1,0,0,0,1,1,0,0,1,1,0,0,1,1,0,0,0,1,1,0,1,0,1,0,0,0,1,0,0,0,1,1,1,1,1,0,1,0,0,1,1,1,1,1,0,0,0,0,0,0,0,0,1,1,1,1,1,0,0,1,0,1,1,1,0,1,0,0,1,1,1,0,1,1,1,0,1,1,1,1,1,1,1,1,1,0,0,1,1,0,0,1,1,1,1,1,1,1,1,1,0,1,1,1,1,0,0,1,1,1,0,0,1,0,1,1,1,1,0,1,1,1,1,0,0,1,0,0,1,1,0,0,1,0,0,1,1,1,1,0,1,1,1,1,0,1,1,1,0,1,1,0,1,1,0,1,1,0,0,1,0,0,1,1,1,1,1,0,1,0,0,0,0,1,0,1,1,1,1,1,0,0,1,0,0,1,1,0,1,0,1,1,0,0,0,1,1,0,1,0,0,1,1,1,1,0,1,0,1,1,0,1,1,1,1,1,1,0,1,1,0,1,0,1,1,1,1,0,0,1,0,1,1,1,1,0,1,0,1,0,0,1,1,0,1,1,0,1,1,1,0,1,0,0,1,1,0,0,0,0,1,1,0,0,1,0,1,1,1,0,1,1,0,1,1,0,0,1,0,1,1,0,1,0,0,1,1,0,0,1,1,0,0,0,1,0,0,1,0,1,0,1,1,1,1,0,1,0,1,0,0,1,0,0,0,1,1,0,0,1,1,0,0,1,1,0,0,1,0,1,0,1,1,0,1,0,0,0,0,0,1,1,0,1,1,1,0,0,0,0,0,0,1,1,1,0,1,1,0,0,0,0,0,1,0,1,1,0,1,0,1,0,0,1,0,1,0,1,0,0,1,0,0,0,1,1,1,0,1,1,1,1,1,0,0,1,1,0,0,1,1,1,1,1,0,1,1,1,0,0,0,1,0,0,1,0,1,0,1,0,1,0,0,1,1,1,1,0,0,0,1,1,1,0,0,0,0,0,1,0,0,0,1,0,0,1,0,0,0,1,0,0,0,0,0,1,1,1,0,0,0,1,1,1,1,0,0,1,1,0,0,1,0,1,0,1,1,1,0,1,0,1,0,0,1,0,0,0,1,1,1,1,1,1,1,1,1,1,0,0,0,1,0,0,1,0,1,0,1,1,1,0,1,0,1,0,0,1]  distributed_mem=Distributed memory  rst=off  init_reg=0  en=off  latency=0  gui_display_data_type=Boolean  arith_type=Boolean  n_bits=2  bin_pt=0  preci_type=Double  exp_width=8  frac_width=24  optimize=Area  use_rpm=on  simulation_type=fast_sim  XmcBlockStatus=1  maskContainerNames=tabcontainer1  block_type=sprom  block_config=sysgen:SPROM_config
  ROM32 : hdlBasic/ROM  depth=1275  initVector=[1,0,1,0,1,1,0,1,0,1,0,0,0,1,1,1,0,0,0,1,1,1,0,1,0,1,1,1,0,1,1,1,0,0,1,1,1,0,1,1,0,1,0,1,1,1,0,0,1,1,0,1,1,0,1,1,1,0,0,1,0,1,1,0,1,1,0,1,0,0,0,0,1,0,0,1,1,1,0,0,0,0,0,0,0,0,1,0,0,0,1,1,1,1,0,1,0,0,0,1,1,1,1,0,0,1,0,1,0,0,1,0,0,1,1,0,0,1,1,0,0,1,0,1,0,0,1,0,0,0,1,0,1,1,1,0,0,1,1,0,0,0,0,1,0,1,0,0,1,0,0,1,0,0,1,0,0,1,1,1,0,1,1,1,1,1,1,0,0,1,0,1,0,1,1,0,1,0,1,1,0,0,1,1,1,1,0,1,1,0,1,1,0,0,1,0,1,0,1,0,0,1,0,1,1,1,1,1,1,0,0,0,0,0,0,0,0,1,0,0,1,0,1,1,1,0,1,1,0,1,0,1,0,0,0,1,1,0,0,1,0,1,0,1,0,1,1,0,0,0,0,0,0,1,0,0,0,1,0,1,1,0,1,0,1,1,0,1,1,1,0,1,1,1,0,0,0,0,1,1,1,1,0,0,0,1,1,0,1,1,0,1,1,1,0,0,0,1,1,0,1,1,0,0,1,1,1,0,0,0,1,0,0,0,0,0,1,1,0,0,0,0,1,1,0,1,1,0,0,1,1,1,0,0,0,1,0,0,0,0,0,1,1,0,0,0,0,1,1,0,0,0,0,1,1,1,1,0,0,0,1,1,0,1,1,0,1,1,1,0,0,0,1,1,0,1,1,0,1,0,0,0,1,0,1,1,0,1,0,1,1,0,1,1,1,0,1,1,1,0,0,1,1,1,1,0,1,0,0,0,1,1,0,0,1,0,1,0,1,0,1,1,0,0,0,0,0,0,0,1,0,0,1,0,0,0,0,0,0,0,0,0,1,0,0,1,0,1,1,1,0,1,1,0,1,0,0,1,0,0,0,0,1,0,0,1,1,0,0,1,0,1,0,1,0,0,1,0,1,1,1,1,1,1,0,1,0,1,0,0,0,0,1,0,1,0,1,0,1,1,0,1,0,1,1,0,0,1,1,1,1,0,1,1,0,1,0,0,1,0,0,0,0,1,0,0,1,0,0,1,0,0,1,1,1,0,1,1,1,1,1,1,0,0,1,0,1,1,1,0,0,1,1,1,1,0,0,1,1,1,0,0,1,1,0,0,0,0,1,0,1,0,0,1,0,0,1,0,1,1,1,1,0,1,1,1,1,1,1,0,1,1,1,1,0,0,1,0,1,0,0,1,0,0,0,1,0,1,1,1,0,1,0,0,1,0,1,1,1,0,0,1,1,1,0,1,0,0,1,0,1,0,1,0,0,1,0,0,1,1,0,0,1,1,0,1,0,0,1,1,1,1,1,0,0,0,0,1,1,1,1,1,0,0,1,0,1,1,1,0,1,0,0,0,1,1,1,1,0,0,1,1,0,1,1,1,1,0,0,1,0,0,1,0,0,1,1,1,1,0,1,1,0,0,0,0,0,0,0,0,0,1,0,0,0,1,0,1,1,1,1,1,0,1,1,1,1,0,0,1,1,1,1,0,1,1,1,1,1,0,1,0,1,0,0,0,0,1,0,0,1,1,1,0,1,0,0,0,1,1,1,0,0,1,0,0,0,0,1,0,0,1,1,1,0,0,0,1,0,1,1,1,0,0,1,0,1,1,0,1,1,1,0,1,0,1,0,1,0,0,1,1,0,1,1,1,1,0,1,1,0,0,1,0,1,0,1,0,1,1,1,0,0,1,1,0,1,1,0,1,1,1,0,1,1,0,1,1,0,0,0,0,1,1,0,0,1,1,0,0,0,0,1,1,0,1,1,0,1,1,1,1,0,1,1,0,1,0,1,1,0,0,0,1,1,1,0,0,1,1,1,0,1,0,0,0,0,0,0,1,0,1,1,1,0,0,1,1,1,0,0,0,1,0,1,1,1,0,0,1,1,1,1,1,0,0,0,0,0,1,0,1,0,1,0,1,0,0,0,0,1,0,1,0,1,0,1,0,0,0,0,0,1,1,1,1,1,0,1,0,1,1,1,1,0,1,1,1,0,0,0,1,0,1,0,1,0,0,1,0,1,1,0,1,0,0,1,0,1,0,1,0,0,0,1,1,1,0,1,1,1,0,0,0,1,1,1,0,1,0,0,0,0,0,1,0,0,1,1,0,0,1,0,1,1,1,1,0,1,0,0,1,1,0,0,1,0,0,0,0,0,1,0,1,1,0,0,0,1,1,1,1,0,0,1,1,0,0,1,0,0,0,1,0,1,0,1,1,1,1,1,1,1,1,0,1,0,1,0,0,0,1,0,0,1,1,0,0,1,1,1,0,1,0,1,1,0,0,1,1,1,0,0,0,0,0,1,0,0,1,0,0,0,0,1,0,0,1,0,0,0,0,1,0,0,1,0,0,0,0,0,1,1,1,0,0,1,1,0,1,1,0,0,0,1,1,1,0,0,0,0,1,1,0,1,0,1,0,0,0,0,1,0,0,1,0,0,0,0,1,0,1,0,1,1,0,0,0,0,1,1,1,0,0,0,1,0,1,1,1,0,0,0,1,0,0,1,1,0,1,0,1,1,1,0,1,0,0,0,0,1,1,0,0,0,0,1,0,1,1,1,0,1,0,1,1,0,0,1,0,0,0,1,1,1,1,0,0,0,0,1,1,0,1,1,1,0,0,1,1,0,0,0,1,1,0,1,1,0,1,1,0,1,1,0,1,1,0,0,0,1,1,0,0,1,1,1,0,1,1,0,0,0,0,1]  distributed_mem=Distributed memory  rst=off  init_reg=0  en=off  latency=0  gui_display_data_type=Boolean  arith_type=Boolean  n_bits=2  bin_pt=0  preci_type=Double  exp_width=8  frac_width=24  optimize=Area  use_rpm=on  simulation_type=fast_sim  XmcBlockStatus=1  maskContainerNames=tabcontainer1  block_type=sprom  block_config=sysgen:SPROM_config
  ROM4 : hdlBasic/ROM  depth=1275  initVector=[1,1,0,0,0,0,0,0,0,1,0,0,1,1,1,0,1,1,1,1,1,0,1,1,1,1,0,0,1,1,1,1,0,0,0,0,1,1,1,0,0,0,0,1,1,1,1,0,0,0,0,1,1,1,1,1,1,0,0,0,1,1,1,1,0,0,1,0,0,0,0,1,1,1,0,0,0,0,0,0,0,0,1,1,1,1,0,0,0,0,1,0,0,0,1,1,1,1,0,0,0,0,1,1,1,0,0,0,1,1,1,0,0,0,0,1,1,1,1,0,0,0,1,1,1,1,0,0,0,1,1,1,1,0,0,0,0,0,1,1,1,0,0,0,0,1,1,1,0,0,0,0,1,0,0,1,1,1,0,0,0,1,1,1,1,0,0,0,1,1,1,0,1,1,1,1,0,0,0,1,1,1,0,0,0,0,1,1,1,1,0,1,1,1,0,0,0,1,1,1,1,0,0,0,1,1,1,1,0,0,0,1,1,1,0,0,0,1,1,1,0,0,0,0,1,1,1,0,0,0,0,0,1,1,1,0,0,0,1,1,1,0,0,0,1,1,1,1,0,0,0,1,1,0,1,1,1,0,0,0,1,1,1,0,0,0,1,1,1,0,0,0,1,1,1,1,0,1,1,1,0,0,0,1,1,1,0,0,0,1,1,1,0,0,0,1,1,1,0,0,0,1,1,1,0,0,0,1,1,1,0,0,0,1,1,1,0,0,0,1,1,1,0,0,0,0,1,1,1,0,0,0,1,1,1,0,0,0,1,1,1,0,0,0,1,1,1,0,0,0,0,0,1,1,1,0,0,0,1,1,1,0,0,0,1,1,1,0,0,0,1,1,1,0,0,0,0,0,0,1,1,1,0,0,0,1,1,1,0,0,0,1,1,1,0,0,0,1,1,1,1,0,0,0,0,1,0,1,1,1,0,0,0,1,1,1,0,0,0,1,1,1,1,0,0,0,1,1,1,1,1,1,1,1,1,0,1,1,1,0,0,0,1,1,1,0,0,0,0,1,1,1,0,0,0,0,1,1,1,1,1,1,1,1,0,0,1,1,1,0,0,0,1,1,1,1,0,0,0,1,1,1,1,0,0,0,0,1,1,1,1,1,1,0,0,0,0,1,1,1,1,0,0,0,1,1,1,0,0,0,0,1,1,1,1,0,0,0,0,0,0,0,0,0,0,0,0,1,0,0,1,1,1,0,0,0,1,1,1,1,0,0,0,1,1,1,1,1,0,0,0,0,0,0,0,0,0,0,1,1,1,0,0,1,1,1,0,0,0,0,1,1,1,0,0,0,0,1,1,1,1,1,1,0,0,0,0,0,0,1,1,1,1,1,1,0,0,1,1,1,1,0,0,0,1,1,1,1,0,0,0,0,1,1,1,1,1,1,1,1,1,1,1,1,1,1,1,1,0,0,0,0,0,1,1,1,0,0,0,0,1,1,1,1,0,0,0,0,0,1,1,1,1,1,1,1,1,1,1,1,1,0,0,0,0,0,0,0,0,1,1,1,1,0,0,0,0,1,1,1,1,0,0,0,0,0,0,1,1,1,1,1,1,1,1,0,0,0,0,0,0,1,1,0,0,0,0,1,1,1,1,0,0,0,0,1,1,1,1,0,0,0,0,0,0,0,0,0,0,0,0,0,0,0,0,0,0,1,1,1,1,1,0,0,0,0,1,1,1,0,0,0,0,0,1,1,1,1,1,0,0,0,0,0,0,0,0,0,0,0,0,0,0,1,1,1,1,1,0,0,1,1,0,0,0,1,1,1,1,0,0,0,0,0,1,1,1,1,1,1,0,0,0,0,0,0,0,0,0,0,1,1,1,1,1,1,0,0,0,0,1,1,0,0,0,0,1,1,1,1,0,0,0,0,0,1,1,1,1,1,1,1,1,1,1,1,1,1,1,1,1,1,1,1,1,0,0,0,0,0,1,1,1,1,0,0,0,0,1,1,1,1,0,0,0,0,0,0,1,1,1,1,1,1,1,1,1,1,1,1,1,1,1,1,0,0,0,0,0,0,1,1,1,1,1,1,1,0,0,0,0,1,1,1,1,1,0,0,0,0,0,0,1,1,1,1,1,1,1,1,1,1,1,1,0,0,0,0,0,0,1,1,1,1,1,0,0,1,1,1,1,0,0,0,0,1,1,1,1,1,0,0,0,0,0,0,0,0,0,0,0,0,0,0,0,0,0,0,0,0,0,0,1,1,1,1,1,0,0,0,0,1,1,1,1,1,0,0,0,0,1,1,1,1,1,1,0,0,0,0,0,0,0,0,0,0,0,0,0,0,0,0,0,0,1,1,1,1,1,1,0,0,0,0,1,0,0,1,1,1,1,1,0,0,0,0,0,1,1,1,1,1,1,1,0,0,0,0,0,0,0,0,0,0,0,0,1,1,1,1,1,1,1,0,0,0,0,0,1,1,1,0,0,0,1,1,1,1,1,0,0,0,0,0,1,1,1,1,1,1,1,1,1,1,1,1,1,1,1,1,1,1,1,1,1,1,1,1,0,0,0,0,0,1,1,1,1,1,0,0,0,0,1,1,1,1,1,0,0,0,0,0,0,1,1,1,1,1,1,1,1,1,1,1,1,1,1,1,1,1,1,1,1,0,0,0,0,0,0,1,1,1,1,1,0,0,1,0,0,0,0,1,1,1,1,1,1,0,0,0,0,0,0,0,1,1,1,1,1,1,1,1,1,1,1,1,1,1,0,0,0,0,0,0,0,1,1,1,1,1,1,0,0,0,0,1,1,0,0,0,0,0,1,1,1,1,1,0,0,0,0,0,0,0,0,0,0,0,0,0,0,0,0,0,0,0,0,0,0,0,0,0,0,1,1,1,1,1,0,0,0,0,0,1,1]  distributed_mem=Distributed memory  rst=off  init_reg=0  en=off  latency=0  gui_display_data_type=Boolean  arith_type=Boolean  n_bits=2  bin_pt=0  preci_type=Double  exp_width=8  frac_width=24  optimize=Area  use_rpm=on  simulation_type=fast_sim  XmcBlockStatus=1  maskContainerNames=tabcontainer1  block_type=sprom  block_config=sysgen:SPROM_config
  ROM5 : hdlBasic/ROM  depth=1275  initVector=[0,0,1,1,1,0,1,0,0,1,0,0,1,1,0,0,1,1,0,0,0,0,1,1,0,0,1,1,1,1,0,0,1,1,0,0,1,0,0,1,1,0,0,1,1,0,0,1,1,0,0,1,1,0,0,0,0,1,0,0,1,1,0,0,1,1,0,1,1,0,0,1,0,0,1,1,0,0,1,1,0,0,1,1,0,0,1,1,0,0,1,1,1,0,1,1,0,0,1,1,0,0,1,1,0,1,0,0,1,1,0,1,1,0,0,1,1,0,0,1,1,0,1,1,0,0,1,1,0,1,1,0,0,1,1,0,0,0,1,1,0,1,1,0,0,1,0,0,1,1,0,0,1,0,0,1,0,0,1,1,0,1,1,0,0,1,0,0,1,1,0,0,1,1,0,0,1,0,0,1,0,0,1,1,0,0,1,0,0,0,0,1,1,0,1,1,0,1,1,0,0,1,0,0,1,1,0,0,1,1,0,1,0,0,1,1,0,1,1,0,1,1,0,0,1,0,0,1,1,0,0,0,1,0,0,1,0,0,1,1,0,1,1,0,1,1,0,0,1,0,0,1,1,0,1,0,0,1,0,0,1,0,0,1,0,0,1,1,0,1,1,0,1,1,0,0,0,1,0,0,1,0,0,1,0,0,1,0,0,1,0,0,1,0,0,1,1,0,1,1,0,1,0,0,1,0,0,1,0,0,1,0,0,1,0,0,1,0,0,1,0,0,1,1,0,0,1,0,0,1,0,0,1,0,0,1,0,0,1,0,0,1,0,0,1,0,0,1,1,0,0,0,1,0,0,1,0,0,1,0,0,1,0,0,1,0,0,1,0,0,1,1,0,1,1,1,1,1,0,1,0,0,1,0,0,1,0,0,1,0,0,1,1,0,1,1,0,1,1,0,0,1,1,1,1,0,0,1,0,0,1,0,0,1,1,0,1,1,0,1,1,0,0,1,0,0,1,1,0,0,0,0,0,0,1,0,1,0,0,1,1,0,1,1,0,1,1,0,0,1,0,0,1,1,0,0,1,1,1,0,0,1,1,1,0,0,1,1,0,1,1,0,1,1,0,0,1,0,0,1,1,0,0,1,1,0,0,1,1,1,1,1,1,0,0,1,0,1,1,0,0,1,0,0,1,0,0,1,1,0,0,1,0,0,0,1,1,0,0,0,0,0,0,0,0,1,1,0,0,0,1,0,0,1,1,0,1,1,0,0,1,0,0,1,1,0,0,0,1,1,1,0,0,0,0,1,1,1,0,0,0,0,0,1,1,0,1,1,0,0,1,0,0,1,1,0,0,1,1,0,0,0,0,1,1,1,1,1,1,0,0,0,0,1,1,1,0,1,1,0,0,1,1,0,1,1,0,0,1,1,0,0,1,1,1,0,0,0,0,0,0,0,0,0,0,1,1,1,0,0,1,0,0,1,1,0,1,1,0,0,1,1,0,0,1,1,0,0,0,1,1,1,1,0,0,0,0,1,1,1,1,0,0,0,1,1,1,1,0,1,1,0,0,1,1,0,0,1,1,0,0,1,1,0,0,0,0,1,1,1,1,1,1,1,1,0,0,0,0,1,1,0,0,1,1,0,0,1,1,0,0,1,1,0,0,1,1,0,0,1,1,1,0,0,0,0,0,0,0,0,0,0,0,0,1,1,1,0,0,1,1,0,1,1,0,0,1,0,0,1,1,0,0,0,1,1,0,0,0,1,1,1,1,0,0,0,0,0,0,1,1,1,1,0,0,0,1,1,0,0,0,0,1,0,0,1,1,0,0,1,1,0,0,0,1,1,0,0,0,0,1,1,1,1,1,1,1,1,1,1,0,0,0,0,1,1,0,0,0,1,0,0,1,1,0,0,1,1,0,0,1,1,1,0,0,1,1,1,0,0,0,0,0,0,0,0,0,0,0,0,0,0,1,1,1,0,0,1,1,1,0,1,0,0,1,1,0,0,1,1,0,0,1,1,1,0,0,0,1,1,1,1,1,0,0,0,0,0,0,1,1,1,1,1,0,0,0,1,1,1,0,0,1,1,1,0,0,1,1,0,0,1,1,0,0,0,1,1,1,0,0,0,1,1,1,1,1,1,1,1,1,1,1,1,0,0,0,1,1,1,0,0,0,1,1,0,0,1,1,0,0,1,1,0,0,1,1,0,0,0,1,1,1,1,0,0,0,0,0,0,0,0,0,0,0,0,0,0,1,1,1,1,0,0,0,1,1,0,0,1,0,1,1,0,0,0,1,1,0,0,1,1,1,0,0,0,1,1,1,1,1,0,0,0,0,0,0,0,0,1,1,1,1,1,0,0,0,1,1,1,0,0,1,1,0,0,0,1,1,0,0,0,1,1,0,0,0,1,1,1,0,0,0,0,1,1,1,1,1,1,1,1,1,1,1,1,0,0,0,0,1,1,1,0,0,0,1,1,0,0,0,1,0,0,1,1,0,0,0,1,1,0,0,0,1,1,1,1,0,0,0,0,0,0,0,0,0,0,0,0,0,0,0,0,1,1,1,1,0,0,0,1,1,0,0,0,1,1,1,1,0,0,1,1,1,0,0,1,1,1,0,0,0,1,1,1,1,1,0,0,0,0,0,0,0,0,0,0,1,1,1,1,1,0,0,0,1,1,1,0,0,1,1,1,0,0,0,1,1,0,0,1,1,1,0,0,0,1,1,1,0,0,0,0,1,1,1,1,1,1,1,1,1,1,1,1,1,1,0,0,0,0,1,1,1,0,0,0,1,1,1,0,0,1,1,0,0,1,1,0,0,0,1,1,0,0,0,1,1,1,1,0,0,0,0,0,0,0,0,0,0,0,0,0,0,0,0,0,0,1,1,1,1,0,0,0,1,1,0,0,0,1,1,0,0]  distributed_mem=Distributed memory  rst=off  init_reg=0  en=off  latency=0  gui_display_data_type=Boolean  arith_type=Boolean  n_bits=2  bin_pt=0  preci_type=Double  exp_width=8  frac_width=24  optimize=Area  use_rpm=on  simulation_type=fast_sim  XmcBlockStatus=1  maskContainerNames=tabcontainer1  block_type=sprom  block_config=sysgen:SPROM_config
  ROM6 : hdlBasic/ROM  depth=1275  initVector=[1,0,1,1,0,1,0,1,0,1,1,0,1,0,1,0,1,0,1,0,0,0,1,0,1,0,1,0,1,0,1,0,1,0,1,0,0,1,0,1,0,1,0,1,0,1,0,1,0,1,0,1,0,1,0,1,0,0,1,0,1,0,1,0,1,0,0,1,0,1,0,0,1,0,1,0,1,0,1,0,1,0,1,0,1,0,1,0,1,0,1,1,0,1,1,0,1,0,1,0,1,0,1,0,1,0,1,0,1,0,0,1,0,1,0,1,0,1,0,1,0,1,1,0,1,0,1,0,0,1,0,1,0,1,0,1,1,0,1,0,0,1,0,1,0,1,1,0,1,0,1,0,1,1,0,0,1,0,1,0,0,1,0,1,0,1,1,0,1,0,1,1,1,0,1,0,0,1,0,1,1,0,1,0,1,0,1,1,0,0,0,1,0,0,1,0,1,1,0,1,0,1,1,0,1,0,1,0,1,0,0,1,1,0,1,0,0,1,0,1,1,0,1,0,0,1,0,1,0,1,0,0,1,1,0,1,1,0,1,0,0,1,0,0,1,0,1,0,0,1,0,1,0,0,0,1,0,0,1,0,1,1,0,1,1,0,1,0,0,1,0,1,1,0,1,0,0,0,1,0,0,1,0,0,1,0,1,1,0,1,1,0,1,1,0,1,0,0,1,0,0,0,1,0,0,1,0,0,1,0,0,1,0,1,1,0,1,1,0,1,1,0,1,0,0,0,0,1,0,0,1,0,0,1,0,0,1,0,1,1,0,1,1,0,1,1,0,1,0,0,0,0,0,1,0,0,1,0,0,1,0,1,1,0,1,1,0,1,1,0,1,0,0,1,0,0,0,0,0,0,1,0,0,1,0,1,1,0,1,1,0,1,0,0,1,0,1,1,0,1,0,1,1,1,1,0,0,1,1,0,1,1,0,1,0,0,1,0,0,1,0,1,0,0,1,0,1,0,1,0,0,0,0,1,0,0,1,1,0,1,0,0,1,0,1,1,0,1,0,0,1,0,1,0,1,0,1,0,0,1,1,0,0,1,0,0,1,0,0,1,0,1,1,0,1,0,1,1,0,1,0,1,0,1,0,1,0,1,1,1,1,1,1,0,1,0,1,1,0,1,0,0,1,0,1,1,0,1,0,1,0,1,1,0,0,1,0,1,1,0,0,0,0,1,1,0,1,0,1,0,0,1,0,1,0,0,1,0,1,0,1,1,0,1,0,1,0,0,1,0,0,1,1,1,1,0,0,1,0,0,1,1,0,1,0,0,1,0,1,0,1,1,0,1,0,1,0,1,0,1,1,0,0,1,1,1,1,1,1,0,0,1,1,0,1,0,1,1,0,1,0,1,0,0,1,0,1,0,1,0,1,0,1,1,0,1,1,0,0,0,0,0,0,1,1,0,1,1,0,1,0,1,0,1,0,0,1,0,1,0,1,0,1,0,1,0,1,0,0,1,0,0,0,1,1,1,1,0,0,0,1,0,0,1,0,1,1,0,1,1,0,1,0,1,0,1,0,1,0,1,0,1,0,1,1,0,0,1,1,1,1,1,1,1,1,0,0,1,1,0,1,0,1,1,0,1,0,1,0,1,0,1,0,1,0,1,0,1,0,1,1,0,1,1,0,0,0,0,0,0,0,0,1,1,0,1,1,0,1,0,1,0,1,0,1,0,0,1,0,1,0,1,0,0,1,0,1,0,0,1,1,0,0,1,1,1,1,1,1,0,0,1,1,0,0,1,0,1,0,0,1,0,0,1,0,1,0,1,0,1,0,1,1,0,1,0,1,1,0,0,1,1,1,1,0,0,1,1,1,1,0,0,1,1,0,1,0,1,1,0,1,0,1,0,1,0,1,0,1,0,1,0,0,1,0,1,1,0,1,1,1,0,0,0,0,0,0,0,0,1,1,1,0,1,1,0,1,0,0,1,0,0,1,0,1,0,1,0,1,0,1,0,1,1,0,1,0,0,1,1,0,0,0,1,1,1,1,1,1,0,0,0,1,1,0,0,1,0,1,1,0,1,0,1,0,1,0,1,0,1,0,1,0,1,0,0,1,0,0,1,0,0,1,1,1,1,0,0,0,0,1,1,1,1,0,0,1,0,0,1,0,0,1,0,1,0,0,1,0,1,0,1,0,1,0,1,0,1,1,0,1,1,0,0,1,1,0,0,0,0,0,0,0,0,0,0,1,1,0,0,1,1,0,1,1,0,1,0,1,0,0,1,0,1,0,0,1,0,1,0,1,0,0,1,0,0,1,1,0,0,0,1,1,1,1,1,1,1,1,0,0,0,1,1,0,0,1,0,0,1,0,1,0,1,0,1,0,1,0,1,0,0,1,0,1,0,0,1,0,0,1,0,0,0,1,1,1,0,0,0,0,0,0,1,1,1,0,0,0,1,0,0,1,0,0,1,0,1,0,0,1,0,1,0,1,0,1,1,0,1,0,1,1,0,1,1,0,0,1,1,0,0,0,0,0,0,0,0,0,0,0,0,1,1,0,0,1,1,0,1,1,0,1,0,1,1,0,1,1,0,1,0,1,0,0,1,0,1,0,0,1,1,0,1,1,0,0,0,1,1,1,1,1,1,1,1,1,1,0,0,0,1,1,0,1,1,0,0,1,0,1,0,0,1,0,1,0,1,0,1,0,1,1,0,1,0,0,1,0,0,1,1,0,0,1,1,1,1,0,0,0,0,0,0,1,1,1,1,0,0,1,1,0,0,1,0,0,1,0,1,1,0,1,0,1,1,0,1,0,1,0,0,1,0,1,1,0,1,1,0,0,1,1,1,0,0,0,0,0,0,0,0,0,0,0,0,1,1,1,0,0,1,1,0,1,1,0,1,0,0,1,0,1,0,1]  distributed_mem=Distributed memory  rst=off  init_reg=0  en=off  latency=0  gui_display_data_type=Boolean  arith_type=Boolean  n_bits=2  bin_pt=0  preci_type=Double  exp_width=8  frac_width=24  optimize=Area  use_rpm=on  simulation_type=fast_sim  XmcBlockStatus=1  maskContainerNames=tabcontainer1  block_type=sprom  block_config=sysgen:SPROM_config
  ROM7 : hdlBasic/ROM  depth=1275  initVector=[0,0,0,0,0,1,1,1,1,1,1,1,1,1,1,1,1,1,1,1,0,0,0,0,0,0,0,0,0,0,0,0,0,0,0,0,1,1,0,0,0,0,0,0,0,1,1,1,1,1,1,1,1,1,1,0,0,1,1,1,1,1,1,1,1,1,1,0,0,0,0,1,1,1,1,1,1,1,1,1,1,0,0,0,0,0,0,0,0,0,0,0,0,0,1,1,1,0,0,0,0,0,0,0,0,1,1,0,0,0,1,1,1,1,0,0,0,0,0,0,0,0,1,1,1,0,0,0,1,1,1,1,1,0,0,1,1,1,0,0,1,1,1,0,0,0,1,1,1,1,1,1,1,0,0,1,1,1,0,0,1,1,0,0,0,0,1,1,1,1,1,0,1,1,0,0,1,1,0,0,1,1,1,0,0,0,0,1,1,0,1,1,0,1,1,0,0,1,1,0,0,0,1,1,0,0,0,0,0,0,1,0,1,1,0,0,1,1,0,0,1,1,0,0,1,1,1,0,0,0,0,0,0,1,0,0,1,1,0,0,1,0,0,1,1,0,0,0,1,1,1,0,0,0,1,1,0,1,1,0,0,1,1,0,1,1,0,0,1,1,0,0,1,1,1,1,0,1,0,0,1,1,0,1,1,0,0,1,0,0,1,1,0,1,1,0,0,1,1,1,0,1,0,0,1,0,0,1,1,0,1,1,0,0,1,0,0,1,1,0,1,1,0,0,1,0,1,0,0,1,0,0,1,1,0,1,1,0,0,1,0,0,1,1,0,1,1,0,0,1,1,0,1,0,0,1,1,0,1,1,0,0,1,0,0,1,1,0,1,1,0,0,1,1,1,0,0,1,0,1,1,0,1,1,0,0,1,1,0,1,1,0,0,1,1,0,0,1,1,1,1,1,0,0,1,1,0,0,1,0,0,1,1,0,0,1,0,0,1,1,0,0,0,1,1,1,0,0,1,1,1,1,1,1,0,1,0,1,1,0,0,1,1,0,0,1,1,0,0,1,1,1,0,0,0,0,0,1,0,1,1,0,1,0,0,1,1,0,1,1,0,0,1,1,0,0,0,1,1,0,0,0,0,0,0,0,1,1,0,0,0,0,1,1,0,0,0,1,1,0,0,1,1,0,0,1,1,1,0,0,0,0,1,1,0,0,0,1,0,1,1,1,1,0,1,0,0,0,0,0,1,1,1,0,0,1,1,0,0,0,0,1,1,1,1,1,1,0,0,1,0,1,1,1,1,0,1,0,0,1,1,1,1,0,0,1,1,1,0,0,0,1,1,1,1,1,1,1,1,1,0,1,0,1,0,0,0,0,1,0,1,0,1,1,1,0,0,1,1,1,0,0,0,1,1,1,1,1,0,0,1,1,1,0,0,1,0,1,1,0,0,1,1,0,1,0,0,1,1,1,1,1,0,0,0,1,1,1,1,0,0,0,0,0,0,0,1,1,0,0,1,0,0,1,1,1,1,0,0,1,0,0,1,1,0,0,0,0,0,1,1,1,0,0,0,0,0,0,0,0,0,0,1,1,0,1,0,1,0,0,0,0,0,0,1,0,1,0,1,1,0,0,0,1,1,1,0,0,0,0,0,0,0,0,0,0,0,0,1,1,0,0,1,0,1,1,0,0,0,0,1,1,0,1,0,0,1,1,0,0,0,1,0,0,0,0,1,1,1,1,1,1,1,0,0,0,1,1,0,1,0,1,0,1,1,1,1,1,1,0,1,0,1,0,1,1,0,0,0,1,0,0,1,1,1,1,1,1,1,1,1,1,0,0,0,1,1,0,1,0,1,0,0,0,1,1,0,0,0,1,0,1,0,1,1,0,0,0,1,1,1,1,1,1,1,1,1,1,1,1,1,1,0,0,0,1,0,0,1,0,0,1,1,0,0,0,0,1,1,0,0,1,0,0,1,0,0,0,1,1,1,1,1,0,0,0,0,0,0,0,1,1,1,0,0,1,1,0,1,0,1,0,0,1,1,1,1,1,1,0,0,1,0,1,0,1,1,0,0,1,1,1,0,0,0,0,0,0,0,0,0,0,1,1,1,0,0,1,0,0,1,0,1,1,0,0,1,1,1,1,0,0,1,1,0,1,0,0,1,0,0,1,1,1,0,0,0,0,0,0,0,0,0,0,0,1,1,1,0,0,1,0,1,0,1,0,1,1,0,0,0,0,0,0,1,1,0,1,0,1,0,1,0,0,1,1,1,0,0,0,1,1,1,1,1,0,0,0,0,1,1,1,0,1,1,0,1,0,1,0,0,1,1,1,0,0,1,1,1,0,0,1,0,1,0,1,1,0,1,1,1,0,0,0,0,1,1,1,1,1,1,0,0,0,1,1,0,0,1,0,1,1,1,0,1,0,0,1,1,1,1,1,1,0,0,1,0,1,1,1,0,1,0,0,1,1,0,0,0,1,1,1,1,1,1,1,1,0,0,0,1,1,0,0,1,0,1,0,1,0,1,1,0,0,0,0,0,0,0,0,1,1,0,1,0,1,0,1,0,0,1,1,0,0,0,1,1,1,0,0,1,1,1,1,0,0,0,1,1,0,1,0,0,1,0,1,1,0,1,1,1,0,0,0,0,1,1,1,0,1,1,0,1,0,0,1,0,1,1,0,0,0,1,1,1,1,0,0,0,1,1,1,0,0,1,1,0,0,1,0,1,0,1,0,1,1,0,0,1,1,1,1,1,1,0,0,1,1,0,1,0,1,0,1,0,0,1,1,0,0,1,1,1,0,0,0,0,0,1,1,1,0,0,1,1,0,1,1,0,1,0,1,0,0,1,1,0,0,0,0,0,0,0,0,1,1,0,0,1,0,1,0,1,1,0,1,1,0,0,1,1,1,0,0,0]  distributed_mem=Distributed memory  rst=off  init_reg=0  en=off  latency=0  gui_display_data_type=Boolean  arith_type=Boolean  n_bits=2  bin_pt=0  preci_type=Double  exp_width=8  frac_width=24  optimize=Area  use_rpm=on  simulation_type=fast_sim  XmcBlockStatus=1  maskContainerNames=tabcontainer1  block_type=sprom  block_config=sysgen:SPROM_config
  ROM8 : hdlBasic/ROM  depth=1275  initVector=[1,1,1,1,1,0,0,0,0,0,0,0,1,1,1,1,1,1,1,1,0,0,0,0,0,0,0,0,1,1,0,0,0,0,1,1,0,0,1,1,1,1,1,1,1,1,1,0,0,0,0,0,0,0,0,0,0,1,1,1,0,0,0,0,0,1,0,1,1,0,0,1,1,1,1,1,1,1,1,1,0,1,1,1,0,0,0,0,0,0,0,1,0,0,1,0,0,1,1,1,0,0,0,0,0,1,0,1,1,0,1,1,0,0,1,1,1,1,1,1,1,0,1,0,0,1,0,0,1,0,0,0,0,1,1,0,1,0,1,0,1,1,0,1,0,0,1,1,0,0,0,0,0,1,0,1,0,0,1,0,1,0,1,1,0,0,1,1,1,1,1,0,1,0,1,0,1,0,1,0,1,1,0,1,1,0,0,1,1,0,1,0,1,1,0,1,0,1,0,1,1,0,1,0,1,1,0,0,0,0,0,1,1,0,1,0,1,0,1,0,1,0,1,0,1,0,0,1,1,1,1,1,0,0,1,0,1,0,1,0,1,1,0,1,0,1,0,0,1,0,0,1,1,0,1,0,1,1,0,1,0,1,0,0,1,0,1,0,1,0,1,0,1,0,0,0,0,1,1,0,1,0,0,1,0,1,0,0,1,0,1,0,1,1,0,1,0,1,1,1,0,0,1,0,1,1,0,1,0,1,1,0,1,0,0,1,0,1,0,0,1,0,1,0,1,0,0,1,0,1,1,0,1,0,1,1,0,1,0,0,1,0,1,0,0,1,0,1,0,1,1,0,1,1,0,1,0,0,1,0,1,0,0,1,0,1,0,1,1,0,1,0,1,1,1,0,0,1,0,1,0,1,1,0,1,0,1,0,0,1,0,1,0,1,0,1,0,1,0,0,0,1,1,1,1,0,1,0,0,1,0,1,0,1,0,1,1,0,1,0,1,0,0,1,0,0,1,1,0,1,0,0,1,0,1,0,1,1,0,1,0,1,0,1,0,1,0,1,0,1,0,0,1,1,1,1,1,0,0,1,1,0,0,1,1,1,0,1,1,0,1,0,1,0,1,1,0,1,0,1,1,0,0,0,0,1,0,1,1,0,0,1,1,0,1,0,0,1,0,1,0,1,0,1,0,1,1,0,1,1,0,0,1,1,0,0,1,0,0,0,0,0,0,0,0,1,0,0,1,0,1,0,0,1,0,1,0,1,1,0,0,1,1,1,1,1,1,0,1,1,1,1,1,1,1,1,1,1,0,1,1,1,0,1,0,1,1,0,1,0,0,1,1,0,0,0,0,0,1,1,0,0,0,0,1,0,0,1,0,0,0,0,1,1,0,1,0,1,0,0,1,0,0,1,0,0,0,0,1,1,0,0,1,0,1,0,0,1,0,1,1,0,1,0,0,1,0,1,0,0,1,0,1,1,0,1,1,0,0,1,1,1,1,1,1,1,0,1,0,1,1,1,0,1,0,0,1,0,1,1,1,0,1,0,1,1,1,0,0,1,0,0,1,1,1,0,0,0,0,0,1,1,0,1,1,0,0,0,1,0,0,0,0,1,0,0,0,1,1,0,1,1,0,1,1,0,1,1,1,0,0,0,0,0,0,0,0,1,0,0,0,1,1,1,1,0,1,1,1,1,0,1,1,1,1,0,0,0,1,0,0,0,1,1,0,0,1,1,1,1,1,1,1,0,0,1,0,1,0,0,0,0,0,1,0,0,0,0,1,0,0,0,0,0,1,0,1,0,0,1,0,0,1,1,1,0,0,0,0,0,1,1,0,0,1,0,1,1,1,1,1,1,0,0,1,1,0,0,1,1,1,1,1,1,0,1,0,0,1,1,1,1,0,0,0,0,0,0,0,0,0,1,0,0,1,0,0,1,1,1,0,1,0,1,1,1,1,0,1,0,1,1,1,0,0,1,0,0,1,0,0,0,0,1,1,1,1,1,1,1,0,0,1,0,1,0,1,0,0,0,0,1,0,1,0,0,0,0,1,0,1,0,0,0,0,1,0,1,0,1,0,0,1,1,1,0,0,0,0,1,1,1,0,0,1,0,1,0,0,1,1,1,1,0,1,0,1,1,1,1,0,1,0,1,1,1,1,0,0,1,0,1,0,0,1,1,0,0,0,0,0,0,0,1,1,0,0,1,0,1,1,0,0,0,0,0,1,0,1,0,0,0,0,1,0,1,0,0,0,0,0,1,1,0,1,0,0,1,1,0,1,1,1,1,1,0,0,0,1,0,0,1,1,0,1,1,1,1,1,1,0,1,0,0,1,1,0,0,1,0,1,1,1,1,1,1,0,1,1,0,0,1,0,0,0,0,0,1,1,1,1,0,0,1,0,1,0,1,0,0,0,1,0,0,0,1,0,1,1,1,1,1,1,0,1,0,0,0,1,0,0,0,1,0,1,0,1,0,0,1,1,0,0,0,0,1,1,0,0,1,0,1,0,1,1,1,0,0,0,1,1,0,1,1,0,0,0,0,1,1,0,1,1,0,0,0,1,1,1,0,1,0,1,0,0,1,1,0,1,1,0,0,1,1,0,0,1,0,1,1,0,0,1,1,1,1,0,1,1,0,0,1,1,1,1,0,0,1,1,0,1,1,1,1,0,0,1,1,0,1,0,0,1,1,0,0,1,1,1,0,0,1,0,1,0,1,0,1,1,0,0,0,0,0,1,0,1,0,1,1,0,0,1,1,0,1,0,1,0,0,0,0,0,1,1,0,1,0,1,0,1,0,0,1,1,1,1,1,0,0,1,0,1,0,1,0,0,1,1,1,1,1,1,0,1,0,1,0,0,0,0,0,0,1,0,1,0,1,1,1,1,1,1,0,0,1,0,1,0,1,0,0,1,1,1]  distributed_mem=Distributed memory  rst=off  init_reg=0  en=off  latency=0  gui_display_data_type=Boolean  arith_type=Boolean  n_bits=2  bin_pt=0  preci_type=Double  exp_width=8  frac_width=24  optimize=Area  use_rpm=on  simulation_type=fast_sim  XmcBlockStatus=1  maskContainerNames=tabcontainer1  block_type=sprom  block_config=sysgen:SPROM_config
  ROM9 : hdlBasic/ROM  depth=1275  initVector=[0,0,1,1,1,0,0,0,1,1,1,1,0,0,0,1,1,1,1,1,0,0,0,0,0,0,0,1,0,0,1,1,1,1,0,0,0,0,1,1,0,0,1,1,1,0,0,1,0,0,0,0,0,0,1,1,0,1,0,0,1,1,1,1,1,0,0,1,0,1,0,1,1,0,0,0,1,1,1,0,0,1,0,0,1,0,0,0,0,0,0,0,1,0,0,1,0,1,0,0,1,1,1,1,1,0,0,1,0,0,1,0,1,0,1,1,0,0,0,1,0,0,1,1,0,0,1,0,0,1,1,0,0,1,1,0,0,1,1,1,1,0,0,1,1,0,1,0,1,1,1,1,1,1,1,1,1,0,0,0,0,1,1,0,1,0,1,0,0,0,0,0,0,0,0,0,0,0,1,1,1,0,0,1,0,1,0,1,1,0,0,0,0,1,1,1,1,1,1,1,0,0,0,1,1,0,1,1,0,1,0,0,1,1,1,1,0,0,0,0,0,0,0,1,1,1,0,1,0,0,0,0,0,1,1,1,1,0,0,0,0,1,1,1,1,1,1,0,0,1,0,1,1,1,0,0,0,1,1,1,0,0,0,1,1,1,0,0,0,0,0,0,1,1,0,0,0,0,1,1,0,0,1,1,1,0,0,1,1,1,0,0,0,1,1,1,1,1,0,0,0,1,1,0,0,1,1,0,0,0,1,1,0,0,1,1,0,0,0,1,1,0,0,0,1,0,1,1,0,0,1,1,0,0,0,1,1,0,0,1,1,0,0,0,1,1,0,0,0,1,1,0,0,1,1,0,0,1,1,1,0,0,1,1,1,0,0,0,1,1,1,1,1,0,0,0,0,0,1,0,0,0,1,1,1,0,0,0,1,1,1,0,0,0,0,0,0,1,1,0,0,0,0,0,0,0,0,0,1,1,1,1,0,0,0,0,1,1,1,1,1,1,0,0,1,0,1,1,0,1,0,0,1,0,1,0,0,1,1,1,1,0,0,0,0,0,0,0,1,1,1,0,1,0,0,0,1,1,1,1,1,1,1,1,0,0,0,0,1,1,1,1,1,1,1,0,0,0,1,1,0,1,1,0,1,0,0,1,1,1,1,1,1,0,0,1,0,0,0,0,0,0,0,1,1,1,0,0,1,0,1,0,1,1,0,0,0,1,0,1,0,0,1,0,1,0,0,0,1,1,1,1,0,0,0,0,1,1,0,1,0,1,0,0,0,0,1,1,1,0,0,1,0,0,1,0,0,1,1,1,0,0,1,1,1,1,0,0,1,1,0,1,0,1,1,1,1,1,0,1,1,0,0,0,0,0,0,0,0,0,0,1,1,0,1,0,0,1,1,0,0,1,0,0,1,1,0,0,1,1,0,1,0,0,0,1,1,0,0,1,1,0,0,1,1,0,0,0,1,0,0,0,1,0,0,1,0,1,0,1,1,0,0,0,1,1,1,0,1,1,1,1,0,0,1,1,0,0,1,1,1,1,0,1,1,1,0,1,0,0,1,0,1,0,0,1,1,1,1,1,0,1,1,1,0,1,1,1,0,1,0,0,1,0,1,1,1,0,1,1,1,0,1,1,0,0,1,0,0,1,0,0,0,0,0,0,1,0,0,1,0,1,0,0,1,1,1,0,0,1,1,1,0,0,1,0,1,0,0,1,0,0,1,0,1,0,1,1,0,0,0,1,1,0,1,0,0,0,1,0,0,0,1,1,1,1,1,1,1,1,0,0,0,1,0,0,0,1,0,1,1,0,1,0,0,1,1,1,1,1,0,1,0,1,1,1,1,0,0,0,0,1,1,0,1,1,0,1,1,0,0,0,0,1,1,1,1,0,1,0,0,0,1,0,0,0,0,0,0,1,1,0,0,1,1,1,0,1,1,1,0,0,0,0,0,0,0,0,0,0,1,1,1,0,1,1,1,0,0,1,1,0,0,1,1,0,0,1,1,1,0,1,0,0,0,0,0,1,1,1,1,0,0,0,1,0,0,1,0,0,0,1,1,1,1,0,0,0,0,0,1,0,1,0,0,1,1,1,1,0,0,1,0,1,0,0,0,1,0,1,0,1,1,0,0,0,1,0,0,1,0,0,0,1,1,0,1,0,1,0,0,0,1,0,1,0,0,0,0,0,0,0,1,0,1,0,1,1,1,1,0,1,0,0,0,1,0,0,1,1,1,1,1,1,0,0,1,0,0,0,1,0,1,1,1,1,0,1,0,1,1,1,1,1,1,0,0,1,0,0,1,1,0,0,1,0,0,0,0,1,1,1,1,0,1,1,0,1,1,1,1,0,0,0,0,1,0,0,1,1,0,0,1,0,0,1,1,0,0,0,1,0,1,0,0,0,0,0,1,0,0,1,0,0,1,1,1,1,0,0,0,0,1,1,1,1,0,0,1,0,0,1,0,0,0,0,0,1,0,1,0,0,0,1,1,0,1,0,1,1,0,0,1,1,0,0,1,1,1,0,1,1,1,0,1,0,0,1,0,1,1,1,0,1,1,1,0,0,1,1,0,0,1,1,0,1,0,1,1,1,0,1,0,1,0,1,1,1,1,0,0,0,1,1,1,1,0,0,1,1,0,1,1,1,1,0,1,1,0,0,1,1,1,1,0,0,0,1,1,1,1,0,1,0,1,0,0,1,1,0,1,1,0,0,0,0,0,1,0,1,0,0,1,1,0,0,0,0,0,0,1,1,0,0,0,0,0,0,1,1,0,0,1,0,1,0,0,0,0,0,1,1,0,1,1,0,0,1,0,1,1,0,0,0,0,1,0,1,0,0,0,0,1,0,0,0,0,1,0,0,0,0,1,0,0,0,0,1,0,0,0,0,1,0,1,0,0,0,0,1,1,0,1,0,0]  distributed_mem=Distributed memory  rst=off  init_reg=0  en=off  latency=0  gui_display_data_type=Boolean  arith_type=Boolean  n_bits=2  bin_pt=0  preci_type=Double  exp_width=8  frac_width=24  optimize=Area  use_rpm=on  simulation_type=fast_sim  XmcBlockStatus=1  maskContainerNames=tabcontainer1  block_type=sprom  block_config=sysgen:SPROM_config
  Scaling : hdlBasic/Scale  scale_factor=-31  XmcBlockStatus=1  maskContainerNames=group1  block_type=scale  block_config=sysgen:Scale_config
  Slice : hdlBasic/Slice  nbits=6  boolean_output=off  mode=Lower Bit Location + Width  bit1=-1  base1=MSB of Input  bit0=0  base0=LSB of Input  XmcBlockStatus=1  maskContainerNames=group1  block_type=slice  block_config=sysgen:Slice_config
  Slice1 : hdlBasic/Slice  nbits=6  boolean_output=off  mode=Lower Bit Location + Width  bit1=-1  base1=MSB of Input  bit0=0  base0=LSB of Input  XmcBlockStatus=1  maskContainerNames=group1  block_type=slice  block_config=sysgen:Slice_config
  Slice2 : hdlBasic/Slice  nbits=21  boolean_output=off  mode=Two Bit Locations  bit1=-1  base1=MSB of Input  bit0=1  base0=LSB of Input  XmcBlockStatus=1  maskContainerNames=group1  block_type=slice  block_config=sysgen:Slice_config
  Slice3 : hdlBasic/Slice  nbits=21  boolean_output=off  mode=Two Bit Locations  bit1=-4  base1=MSB of Input  bit0=0  base0=LSB of Input  XmcBlockStatus=1  maskContainerNames=group1  block_type=slice  block_config=sysgen:Slice_config
  addsub{1..98} (98 alike) : hdlBasic/AddSub  mode=Addition  use_carryin=off  use_carryout=off  en=off  latency=0  precision=User Defined  arith_type=Unsigned  n_bits=6  bin_pt=0  quantization="Round  (unbiased: +/- Inf)"  overflow=Saturate  use_behavioral_HDL=off  hw_selection=Fabric  pipelined=on  XmcBlockStatus=1  maskContainerNames=tabcontainer1  block_type=addsub  block_config=sysgen:Addsub_config
  addsub100 : hdlBasic/AddSub  mode=Addition  use_carryin=off  use_carryout=off  en=off  latency=0  precision=Full  arith_type=Unsigned  n_bits=16  bin_pt=14  quantization=Truncate  overflow=Saturate  use_behavioral_HDL=off  hw_selection=Fabric  pipelined=on  XmcBlockStatus=1  maskContainerNames=tabcontainer1  block_type=addsub  block_config=sysgen:Addsub_config
  addsub101 : hdlBasic/AddSub  mode=Subtraction  use_carryin=off  use_carryout=off  en=off  latency=0  precision=User Defined  arith_type=Unsigned  n_bits=13  bin_pt=0  quantization=Truncate  overflow=Saturate  use_behavioral_HDL=off  hw_selection=Fabric  pipelined=on  XmcBlockStatus=1  maskContainerNames=tabcontainer1  block_type=addsub  block_config=sysgen:Addsub_config
  addsub102 : hdlBasic/AddSub  mode=Addition  use_carryin=off  use_carryout=off  en=off  latency=0  precision=Full  arith_type=Unsigned  n_bits=16  bin_pt=14  quantization=Truncate  overflow=Saturate  use_behavioral_HDL=off  hw_selection=Fabric  pipelined=on  XmcBlockStatus=1  maskContainerNames=tabcontainer1  block_type=addsub  block_config=sysgen:Addsub_config
  addsub103 : hdlBasic/AddSub  mode=Subtraction  use_carryin=off  use_carryout=off  en=off  latency=0  precision=Full  arith_type=Unsigned  n_bits=6  bin_pt=0  quantization=Truncate  overflow=Saturate  use_behavioral_HDL=off  hw_selection=Fabric  pipelined=on  XmcBlockStatus=1  maskContainerNames=tabcontainer1  block_type=addsub  block_config=sysgen:Addsub_config
  addsub99 : hdlBasic/AddSub  mode=Subtraction  use_carryin=off  use_carryout=off  en=off  latency=0  precision=Full  arith_type=Unsigned  n_bits=5  bin_pt=0  quantization=Truncate  overflow=Saturate  use_behavioral_HDL=off  hw_selection=Fabric  pipelined=on  XmcBlockStatus=1  maskContainerNames=tabcontainer1  block_type=addsub  block_config=sysgen:Addsub_config
  bool1 : hdlBasic/Relational  mode=a<b  op_type=Bool  en=off  latency=0  XmcBlockStatus=1  maskContainerNames=tabcontainer1  block_type=relational  block_config=sysgen:Relational_config
  logi_b0 : hdlBasic/Constant  const=-1.0000000000000000000000000000000000000000000000000000000  gui_display_data_type=Fixed-point  arith_type=Signed (2's comp)  n_bits=32  bin_pt=31  preci_type=Double  exp_width=8  frac_width=24  explicit_period=on  period=1  XmcBlockStatus=1  maskContainerNames=tabcontainer1  block_type=constant  block_config=sysgen:Constant_config
  logi_b1 : hdlBasic/Constant  const=-0.9591836734693877097868153214221820235252380371093750000  gui_display_data_type=Fixed-point  arith_type=Signed (2's comp)  n_bits=32  bin_pt=31  preci_type=Double  exp_width=8  frac_width=24  explicit_period=on  period=1  XmcBlockStatus=1  maskContainerNames=tabcontainer1  block_type=constant  block_config=sysgen:Constant_config
  logi_b10 : hdlBasic/Constant  const=-0.5918367346938775419573630642844364047050476074218750000  gui_display_data_type=Fixed-point  arith_type=Signed (2's comp)  n_bits=32  bin_pt=31  preci_type=Double  exp_width=8  frac_width=24  explicit_period=on  period=1  XmcBlockStatus=1  maskContainerNames=tabcontainer1  block_type=constant  block_config=sysgen:Constant_config
  logi_b11 : hdlBasic/Constant  const=-0.5510204081632652517441783857066184282302856445312500000  gui_display_data_type=Fixed-point  arith_type=Signed (2's comp)  n_bits=32  bin_pt=31  preci_type=Double  exp_width=8  frac_width=24  explicit_period=on  period=1  XmcBlockStatus=1  maskContainerNames=tabcontainer1  block_type=constant  block_config=sysgen:Constant_config
  logi_b12 : hdlBasic/Constant  const=-0.5102040816326530725532961696444544941186904907226562500  gui_display_data_type=Fixed-point  arith_type=Signed (2's comp)  n_bits=32  bin_pt=31  preci_type=Double  exp_width=8  frac_width=24  explicit_period=on  period=1  XmcBlockStatus=1  maskContainerNames=tabcontainer1  block_type=constant  block_config=sysgen:Constant_config
  logi_b13 : hdlBasic/Constant  const=-0.4693877551020407823401114910666365176439285278320312500  gui_display_data_type=Fixed-point  arith_type=Signed (2's comp)  n_bits=32  bin_pt=31  preci_type=Double  exp_width=8  frac_width=24  explicit_period=on  period=1  XmcBlockStatus=1  maskContainerNames=tabcontainer1  block_type=constant  block_config=sysgen:Constant_config
  logi_b14 : hdlBasic/Constant  const=-0.4285714285714285476380780437466455623507499694824218750  gui_display_data_type=Fixed-point  arith_type=Signed (2's comp)  n_bits=32  bin_pt=31  preci_type=Double  exp_width=8  frac_width=24  explicit_period=on  period=1  XmcBlockStatus=1  maskContainerNames=tabcontainer1  block_type=constant  block_config=sysgen:Constant_config
  logi_b15 : hdlBasic/Constant  const=-0.3877551020408163129360445964266546070575714111328125000  gui_display_data_type=Fixed-point  arith_type=Signed (2's comp)  n_bits=32  bin_pt=31  preci_type=Double  exp_width=8  frac_width=24  explicit_period=on  period=1  XmcBlockStatus=1  maskContainerNames=tabcontainer1  block_type=constant  block_config=sysgen:Constant_config
  logi_b16 : hdlBasic/Constant  const=-0.3469387755102040782340111491066636517643928527832031250  gui_display_data_type=Fixed-point  arith_type=Signed (2's comp)  n_bits=32  bin_pt=31  preci_type=Double  exp_width=8  frac_width=24  explicit_period=on  period=1  XmcBlockStatus=1  maskContainerNames=tabcontainer1  block_type=constant  block_config=sysgen:Constant_config
  logi_b17 : hdlBasic/Constant  const=-0.3061224489795917880208264705288456752896308898925781250  gui_display_data_type=Fixed-point  arith_type=Signed (2's comp)  n_bits=32  bin_pt=31  preci_type=Double  exp_width=8  frac_width=24  explicit_period=on  period=1  XmcBlockStatus=1  maskContainerNames=tabcontainer1  block_type=constant  block_config=sysgen:Constant_config
  logi_b18 : hdlBasic/Constant  const=-0.2653061224489795533187930232088547199964523315429687500  gui_display_data_type=Fixed-point  arith_type=Signed (2's comp)  n_bits=32  bin_pt=31  preci_type=Double  exp_width=8  frac_width=24  explicit_period=on  period=1  XmcBlockStatus=1  maskContainerNames=tabcontainer1  block_type=constant  block_config=sysgen:Constant_config
  logi_b19 : hdlBasic/Constant  const=-0.2244897959183673186167595758888637647032737731933593750  gui_display_data_type=Fixed-point  arith_type=Signed (2's comp)  n_bits=32  bin_pt=31  preci_type=Double  exp_width=8  frac_width=24  explicit_period=on  period=1  XmcBlockStatus=1  maskContainerNames=tabcontainer1  block_type=constant  block_config=sysgen:Constant_config
  logi_b2 : hdlBasic/Constant  const=-0.9183673469387754195736306428443640470504760742187500000  gui_display_data_type=Fixed-point  arith_type=Signed (2's comp)  n_bits=32  bin_pt=31  preci_type=Double  exp_width=8  frac_width=24  explicit_period=on  period=1  XmcBlockStatus=1  maskContainerNames=tabcontainer1  block_type=constant  block_config=sysgen:Constant_config
  logi_b20 : hdlBasic/Constant  const=-0.1836734693877550839147261285688728094100952148437500000  gui_display_data_type=Fixed-point  arith_type=Signed (2's comp)  n_bits=32  bin_pt=31  preci_type=Double  exp_width=8  frac_width=24  explicit_period=on  period=1  XmcBlockStatus=1  maskContainerNames=tabcontainer1  block_type=constant  block_config=sysgen:Constant_config
  logi_b21 : hdlBasic/Constant  const=-0.1428571428571428492126926812488818541169166564941406250  gui_display_data_type=Fixed-point  arith_type=Signed (2's comp)  n_bits=32  bin_pt=31  preci_type=Double  exp_width=8  frac_width=24  explicit_period=on  period=1  XmcBlockStatus=1  maskContainerNames=tabcontainer1  block_type=constant  block_config=sysgen:Constant_config
  logi_b22 : hdlBasic/Constant  const=-0.1020408163265306006328714261144341435283422470092773438  gui_display_data_type=Fixed-point  arith_type=Signed (2's comp)  n_bits=32  bin_pt=31  preci_type=Double  exp_width=8  frac_width=24  explicit_period=on  period=1  XmcBlockStatus=1  maskContainerNames=tabcontainer1  block_type=constant  block_config=sysgen:Constant_config
  logi_b23 : hdlBasic/Constant  const=-0.0612244897959183659308379787944431882351636886596679688  gui_display_data_type=Fixed-point  arith_type=Signed (2's comp)  n_bits=32  bin_pt=31  preci_type=Double  exp_width=8  frac_width=24  explicit_period=on  period=1  XmcBlockStatus=1  maskContainerNames=tabcontainer1  block_type=constant  block_config=sysgen:Constant_config
  logi_b24 : hdlBasic/Constant  const=-0.0204081632653061208204636756136096664704382419586181641  gui_display_data_type=Fixed-point  arith_type=Signed (2's comp)  n_bits=32  bin_pt=31  preci_type=Double  exp_width=8  frac_width=24  explicit_period=on  period=1  XmcBlockStatus=1  maskContainerNames=tabcontainer1  block_type=constant  block_config=sysgen:Constant_config
  logi_b25 : hdlBasic/Constant  const=0.0204081632653061208204636756136096664704382419586181641  gui_display_data_type=Fixed-point  arith_type=Signed (2's comp)  n_bits=32  bin_pt=31  preci_type=Double  exp_width=8  frac_width=24  explicit_period=on  period=1  XmcBlockStatus=1  maskContainerNames=tabcontainer1  block_type=constant  block_config=sysgen:Constant_config
  logi_b26 : hdlBasic/Constant  const=0.0612244897959183659308379787944431882351636886596679688  gui_display_data_type=Fixed-point  arith_type=Signed (2's comp)  n_bits=32  bin_pt=31  preci_type=Double  exp_width=8  frac_width=24  explicit_period=on  period=1  XmcBlockStatus=1  maskContainerNames=tabcontainer1  block_type=constant  block_config=sysgen:Constant_config
  logi_b27 : hdlBasic/Constant  const=0.1020408163265306006328714261144341435283422470092773438  gui_display_data_type=Fixed-point  arith_type=Signed (2's comp)  n_bits=32  bin_pt=31  preci_type=Double  exp_width=8  frac_width=24  explicit_period=on  period=1  XmcBlockStatus=1  maskContainerNames=tabcontainer1  block_type=constant  block_config=sysgen:Constant_config
  logi_b28 : hdlBasic/Constant  const=0.1428571428571428492126926812488818541169166564941406250  gui_display_data_type=Fixed-point  arith_type=Signed (2's comp)  n_bits=32  bin_pt=31  preci_type=Double  exp_width=8  frac_width=24  explicit_period=on  period=1  XmcBlockStatus=1  maskContainerNames=tabcontainer1  block_type=constant  block_config=sysgen:Constant_config
  logi_b29 : hdlBasic/Constant  const=0.1836734693877550839147261285688728094100952148437500000  gui_display_data_type=Fixed-point  arith_type=Signed (2's comp)  n_bits=32  bin_pt=31  preci_type=Double  exp_width=8  frac_width=24  explicit_period=on  period=1  XmcBlockStatus=1  maskContainerNames=tabcontainer1  block_type=constant  block_config=sysgen:Constant_config
  logi_b3 : hdlBasic/Constant  const=-0.8775510204081632403827484267822001129388809204101562500  gui_display_data_type=Fixed-point  arith_type=Signed (2's comp)  n_bits=32  bin_pt=31  preci_type=Double  exp_width=8  frac_width=24  explicit_period=on  period=1  XmcBlockStatus=1  maskContainerNames=tabcontainer1  block_type=constant  block_config=sysgen:Constant_config
  logi_b30 : hdlBasic/Constant  const=0.2244897959183673186167595758888637647032737731933593750  gui_display_data_type=Fixed-point  arith_type=Signed (2's comp)  n_bits=32  bin_pt=31  preci_type=Double  exp_width=8  frac_width=24  explicit_period=on  period=1  XmcBlockStatus=1  maskContainerNames=tabcontainer1  block_type=constant  block_config=sysgen:Constant_config
  logi_b31 : hdlBasic/Constant  const=0.2653061224489795533187930232088547199964523315429687500  gui_display_data_type=Fixed-point  arith_type=Signed (2's comp)  n_bits=32  bin_pt=31  preci_type=Double  exp_width=8  frac_width=24  explicit_period=on  period=1  XmcBlockStatus=1  maskContainerNames=tabcontainer1  block_type=constant  block_config=sysgen:Constant_config
  logi_b32 : hdlBasic/Constant  const=0.3061224489795917880208264705288456752896308898925781250  gui_display_data_type=Fixed-point  arith_type=Signed (2's comp)  n_bits=32  bin_pt=31  preci_type=Double  exp_width=8  frac_width=24  explicit_period=on  period=1  XmcBlockStatus=1  maskContainerNames=tabcontainer1  block_type=constant  block_config=sysgen:Constant_config
  logi_b33 : hdlBasic/Constant  const=0.3469387755102040782340111491066636517643928527832031250  gui_display_data_type=Fixed-point  arith_type=Signed (2's comp)  n_bits=32  bin_pt=31  preci_type=Double  exp_width=8  frac_width=24  explicit_period=on  period=1  XmcBlockStatus=1  maskContainerNames=tabcontainer1  block_type=constant  block_config=sysgen:Constant_config
  logi_b34 : hdlBasic/Constant  const=0.3877551020408163129360445964266546070575714111328125000  gui_display_data_type=Fixed-point  arith_type=Signed (2's comp)  n_bits=32  bin_pt=31  preci_type=Double  exp_width=8  frac_width=24  explicit_period=on  period=1  XmcBlockStatus=1  maskContainerNames=tabcontainer1  block_type=constant  block_config=sysgen:Constant_config
  logi_b35 : hdlBasic/Constant  const=0.4285714285714285476380780437466455623507499694824218750  gui_display_data_type=Fixed-point  arith_type=Signed (2's comp)  n_bits=32  bin_pt=31  preci_type=Double  exp_width=8  frac_width=24  explicit_period=on  period=1  XmcBlockStatus=1  maskContainerNames=tabcontainer1  block_type=constant  block_config=sysgen:Constant_config
  logi_b36 : hdlBasic/Constant  const=0.4693877551020407823401114910666365176439285278320312500  gui_display_data_type=Fixed-point  arith_type=Signed (2's comp)  n_bits=32  bin_pt=31  preci_type=Double  exp_width=8  frac_width=24  explicit_period=on  period=1  XmcBlockStatus=1  maskContainerNames=tabcontainer1  block_type=constant  block_config=sysgen:Constant_config
  logi_b37 : hdlBasic/Constant  const=0.5102040816326530725532961696444544941186904907226562500  gui_display_data_type=Fixed-point  arith_type=Signed (2's comp)  n_bits=32  bin_pt=31  preci_type=Double  exp_width=8  frac_width=24  explicit_period=on  period=1  XmcBlockStatus=1  maskContainerNames=tabcontainer1  block_type=constant  block_config=sysgen:Constant_config
  logi_b38 : hdlBasic/Constant  const=0.5510204081632652517441783857066184282302856445312500000  gui_display_data_type=Fixed-point  arith_type=Signed (2's comp)  n_bits=32  bin_pt=31  preci_type=Double  exp_width=8  frac_width=24  explicit_period=on  period=1  XmcBlockStatus=1  maskContainerNames=tabcontainer1  block_type=constant  block_config=sysgen:Constant_config
  logi_b39 : hdlBasic/Constant  const=0.5918367346938775419573630642844364047050476074218750000  gui_display_data_type=Fixed-point  arith_type=Signed (2's comp)  n_bits=32  bin_pt=31  preci_type=Double  exp_width=8  frac_width=24  explicit_period=on  period=1  XmcBlockStatus=1  maskContainerNames=tabcontainer1  block_type=constant  block_config=sysgen:Constant_config
  logi_b4 : hdlBasic/Constant  const=-0.8367346938775509501695637482043821364641189575195312500  gui_display_data_type=Fixed-point  arith_type=Signed (2's comp)  n_bits=32  bin_pt=31  preci_type=Double  exp_width=8  frac_width=24  explicit_period=on  period=1  XmcBlockStatus=1  maskContainerNames=tabcontainer1  block_type=constant  block_config=sysgen:Constant_config
  logi_b40 : hdlBasic/Constant  const=0.6326530612244897211482452803466003388166427612304687500  gui_display_data_type=Fixed-point  arith_type=Signed (2's comp)  n_bits=32  bin_pt=31  preci_type=Double  exp_width=8  frac_width=24  explicit_period=on  period=1  XmcBlockStatus=1  maskContainerNames=tabcontainer1  block_type=constant  block_config=sysgen:Constant_config
  logi_b41 : hdlBasic/Constant  const=0.6734693877551020113614299589244183152914047241210937500  gui_display_data_type=Fixed-point  arith_type=Signed (2's comp)  n_bits=32  bin_pt=31  preci_type=Double  exp_width=8  frac_width=24  explicit_period=on  period=1  XmcBlockStatus=1  maskContainerNames=tabcontainer1  block_type=constant  block_config=sysgen:Constant_config
  logi_b42 : hdlBasic/Constant  const=0.7142857142857141905523121749865822494029998779296875000  gui_display_data_type=Fixed-point  arith_type=Signed (2's comp)  n_bits=32  bin_pt=31  preci_type=Double  exp_width=8  frac_width=24  explicit_period=on  period=1  XmcBlockStatus=1  maskContainerNames=tabcontainer1  block_type=constant  block_config=sysgen:Constant_config
  logi_b43 : hdlBasic/Constant  const=0.7551020408163264807654968535644002258777618408203125000  gui_display_data_type=Fixed-point  arith_type=Signed (2's comp)  n_bits=32  bin_pt=31  preci_type=Double  exp_width=8  frac_width=24  explicit_period=on  period=1  XmcBlockStatus=1  maskContainerNames=tabcontainer1  block_type=constant  block_config=sysgen:Constant_config
  logi_b44 : hdlBasic/Constant  const=0.7959183673469386599563790696265641599893569946289062500  gui_display_data_type=Fixed-point  arith_type=Signed (2's comp)  n_bits=32  bin_pt=31  preci_type=Double  exp_width=8  frac_width=24  explicit_period=on  period=1  XmcBlockStatus=1  maskContainerNames=tabcontainer1  block_type=constant  block_config=sysgen:Constant_config
  logi_b45 : hdlBasic/Constant  const=0.8367346938775509501695637482043821364641189575195312500  gui_display_data_type=Fixed-point  arith_type=Signed (2's comp)  n_bits=32  bin_pt=31  preci_type=Double  exp_width=8  frac_width=24  explicit_period=on  period=1  XmcBlockStatus=1  maskContainerNames=tabcontainer1  block_type=constant  block_config=sysgen:Constant_config
  logi_b46 : hdlBasic/Constant  const=0.8775510204081632403827484267822001129388809204101562500  gui_display_data_type=Fixed-point  arith_type=Signed (2's comp)  n_bits=32  bin_pt=31  preci_type=Double  exp_width=8  frac_width=24  explicit_period=on  period=1  XmcBlockStatus=1  maskContainerNames=tabcontainer1  block_type=constant  block_config=sysgen:Constant_config
  logi_b47 : hdlBasic/Constant  const=0.9183673469387754195736306428443640470504760742187500000  gui_display_data_type=Fixed-point  arith_type=Signed (2's comp)  n_bits=32  bin_pt=31  preci_type=Double  exp_width=8  frac_width=24  explicit_period=on  period=1  XmcBlockStatus=1  maskContainerNames=tabcontainer1  block_type=constant  block_config=sysgen:Constant_config
  logi_b48 : hdlBasic/Constant  const=0.9591836734693877097868153214221820235252380371093750000  gui_display_data_type=Fixed-point  arith_type=Signed (2's comp)  n_bits=32  bin_pt=31  preci_type=Double  exp_width=8  frac_width=24  explicit_period=on  period=1  XmcBlockStatus=1  maskContainerNames=tabcontainer1  block_type=constant  block_config=sysgen:Constant_config
  logi_b49 : hdlBasic/Constant  const=1.0000000000000000000000000000000000000000000000000000000  gui_display_data_type=Fixed-point  arith_type=Signed (2's comp)  n_bits=32  bin_pt=31  preci_type=Double  exp_width=8  frac_width=24  explicit_period=on  period=1  XmcBlockStatus=1  maskContainerNames=tabcontainer1  block_type=constant  block_config=sysgen:Constant_config
  logi_b5 : hdlBasic/Constant  const=-0.7959183673469386599563790696265641599893569946289062500  gui_display_data_type=Fixed-point  arith_type=Signed (2's comp)  n_bits=32  bin_pt=31  preci_type=Double  exp_width=8  frac_width=24  explicit_period=on  period=1  XmcBlockStatus=1  maskContainerNames=tabcontainer1  block_type=constant  block_config=sysgen:Constant_config
  logi_b6 : hdlBasic/Constant  const=-0.7551020408163264807654968535644002258777618408203125000  gui_display_data_type=Fixed-point  arith_type=Signed (2's comp)  n_bits=32  bin_pt=31  preci_type=Double  exp_width=8  frac_width=24  explicit_period=on  period=1  XmcBlockStatus=1  maskContainerNames=tabcontainer1  block_type=constant  block_config=sysgen:Constant_config
  logi_b7 : hdlBasic/Constant  const=-0.7142857142857141905523121749865822494029998779296875000  gui_display_data_type=Fixed-point  arith_type=Signed (2's comp)  n_bits=32  bin_pt=31  preci_type=Double  exp_width=8  frac_width=24  explicit_period=on  period=1  XmcBlockStatus=1  maskContainerNames=tabcontainer1  block_type=constant  block_config=sysgen:Constant_config
  logi_b8 : hdlBasic/Constant  const=-0.6734693877551020113614299589244183152914047241210937500  gui_display_data_type=Fixed-point  arith_type=Signed (2's comp)  n_bits=32  bin_pt=31  preci_type=Double  exp_width=8  frac_width=24  explicit_period=on  period=1  XmcBlockStatus=1  maskContainerNames=tabcontainer1  block_type=constant  block_config=sysgen:Constant_config
  logi_b9 : hdlBasic/Constant  const=-0.6326530612244897211482452803466003388166427612304687500  gui_display_data_type=Fixed-point  arith_type=Signed (2's comp)  n_bits=32  bin_pt=31  preci_type=Double  exp_width=8  frac_width=24  explicit_period=on  period=1  XmcBlockStatus=1  maskContainerNames=tabcontainer1  block_type=constant  block_config=sysgen:Constant_config
  mult1 : hdlBasic/Mult  precision=Full  arith_type="Signed  (2's comp)"  n_bits=30  bin_pt=16  quantization="Round  (unbiased: +/- Inf)"  overflow=Saturate  en=off  latency=0  use_behavioral_HDL=off  opt=Area  use_embedded=off  optimum_pipeline=off  pipeline=on  use_rpm=on  placement_style=Triangular  XmcBlockStatus=1  maskContainerNames=group1  block_type=mult  block_config=sysgen:Mult_config
  mux{1..102} (102 alike) : hdlBasic/Mux  inputs=2  en=off  latency=0  precision=Full  arith_type=Unsigned  n_bits=16  bin_pt=14  quantization=Truncate  overflow=Wrap  XmcBlockStatus=1  maskContainerNames=tabcontainer1  block_type=mux  block_config=sysgen:Mux_config
  rela{1..100} (100 alike) : hdlBasic/Relational  mode=a>=b  op_type=Bool  en=off  latency=0  XmcBlockStatus=1  maskContainerNames=tabcontainer1  block_type=relational  block_config=sysgen:Relational_config
  Output : Outport
  wires:
  addsub9/1 -> mux13/3
  In4/1 -> Gate_In2/1
  addsub13/1 -> mux17/3
  In3/1 -> Gate_In1/1
  addsub1/1 -> mux5/3
  addsub5/1 -> mux9/3
  addsub3/1 -> mux7/3
  rela1/1 -> mux3/1
  addsub7/1 -> mux11/3
  addsub11/1 -> mux15/3
  addsub15/1 -> mux19/3
  bool1/1 -> mux2/1, mux1/1
  Constant3/1 -> addsub100/2
  Constant/1 -> addsub99/2
  addsub100/1 -> mult1/2
  addsub99/1 -> Negate/1
  addsub103/1 -> Slice3/1
  addsub102/1 -> addsub103/1
  addsub101/1 -> addsub102/1
  CMult1/1 -> addsub101/1
  Negate/1 -> addsub100/1
  mult1/1 -> Slice2/1
  Gate_In2/1 -> bool1/2, mux2/2, mux1/3
  Gate_In1/1 -> bool1/1, mux2/3, mux1/2
  rela3/1 -> mux5/1
  mux3/1 -> mux5/2, addsub1/1
  rela5/1 -> mux7/1
  mux5/1 -> mux7/2, addsub3/1
  rela7/1 -> mux9/1
  mux7/1 -> mux9/2, addsub5/1
  rela9/1 -> mux11/1
  mux9/1 -> mux11/2, addsub7/1
  rela11/1 -> mux13/1
  mux11/1 -> mux13/2, addsub9/1
  rela13/1 -> mux15/1
  mux13/1 -> mux15/2, addsub11/1
  rela15/1 -> mux17/1
  mux15/1 -> mux17/2, addsub13/1
  rela17/1 -> mux19/1
  mux17/1 -> mux19/2, addsub15/1
  mux6/1 -> mux8/2, addsub4/1
  mux16/1 -> mux18/2, addsub14/1
  rela18/1 -> mux20/1
  rela10/1 -> mux12/1
  logi_b3/1 -> rela8/2, rela7/2
  addsub4/1 -> mux8/3
  addsub12/1 -> mux16/3
  rela12/1 -> mux14/1
  logi_b1/1 -> rela4/2, rela3/2
  rela2/1 -> mux4/1
  addsub6/1 -> mux10/3
  mux8/1 -> mux10/2, addsub6/1
  rela14/1 -> mux16/1
  logi_b4/1 -> rela10/2, rela9/2
  mux10/1 -> mux12/2, addsub8/1
  logi_b7/1 -> rela16/2, rela15/2
  rela16/1 -> mux18/1
  logi_b0/1 -> rela2/2, rela1/2
  mux18/1 -> mux20/2, addsub16/1
  logi_b5/1 -> rela12/2, rela11/2
  mux4/1 -> mux6/2, addsub2/1
  rela8/1 -> mux10/1
  mux14/1 -> mux16/2, addsub12/1
  rela6/1 -> mux8/1
  logi_b2/1 -> rela5/2, rela6/2
  addsub8/1 -> mux12/3
  addsub14/1 -> mux18/3
  mux12/1 -> mux14/2, addsub10/1
  logi_b6/1 -> rela14/2, rela13/2
  rela4/1 -> mux6/1
  addsub10/1 -> mux14/3
  addsub16/1 -> mux20/3
  logi_b8/1 -> rela18/2, rela17/2
  addsub2/1 -> mux6/3
  Constant6/1 -> mux4/2
  Constant1/1 -> mux3/2
  Slice/1 -> CMult1/1, mult1/1, addsub99/1
  Slice1/1 -> addsub102/2
  rela36/1 -> mux38/1
  rela32/1 -> mux34/1
  mux31/1 -> mux33/2, addsub29/1
  rela28/1 -> mux30/1
  rela30/1 -> mux32/1
  mux30/1 -> mux32/2, addsub28/1
  addsub28/1 -> mux32/3
  rela24/1 -> mux26/1
  mux26/1 -> mux28/2, addsub24/1
  addsub19/1 -> mux23/3
  addsub25/1 -> mux29/3
  logi_b11/1 -> rela24/2, rela23/2
  rela35/1 -> mux37/1
  rela29/1 -> mux31/1
  addsub32/1 -> mux36/3
  rela34/1 -> mux36/1
  rela27/1 -> mux29/1
  logi_b13/1 -> rela28/2, rela27/2
  logi_b15/1 -> rela32/2, rela31/2
  rela26/1 -> mux28/1
  addsub22/1 -> mux26/3
  logi_b17/1 -> rela36/2, rela35/2
  addsub29/1 -> mux33/3
  mux28/1 -> mux30/2, addsub26/1
  addsub26/1 -> mux30/3
  rela23/1 -> mux25/1
  rela33/1 -> mux35/1
  mux34/1 -> mux36/2, addsub32/1
  addsub33/1 -> mux37/3
  mux29/1 -> mux31/2, addsub27/1
  addsub27/1 -> mux31/3
  addsub24/1 -> mux28/3
  mux32/1 -> mux34/2, addsub30/1
  logi_b12/1 -> rela26/2, rela25/2
  rela22/1 -> mux24/1
  rela31/1 -> mux33/1
  mux35/1 -> mux37/2, addsub33/1
  logi_b10/1 -> rela22/2, rela21/2
  logi_b16/1 -> rela34/2, rela33/2
  addsub20/1 -> mux24/3
  addsub34/1 -> mux38/3
  mux27/1 -> mux29/2, addsub25/1
  addsub23/1 -> mux27/3
  mux21/1 -> mux23/2, addsub19/1
  addsub21/1 -> mux25/3
  mux36/1 -> mux38/2, addsub34/1
  mux22/1 -> mux24/2, addsub20/1
  mux25/1 -> mux27/2, addsub23/1
  mux23/1 -> mux25/2, addsub21/1
  addsub30/1 -> mux34/3
  addsub31/1 -> mux35/3
  logi_b14/1 -> rela30/2, rela29/2
  rela21/1 -> mux23/1
  mux24/1 -> mux26/2, addsub22/1
  mux33/1 -> mux35/2, addsub31/1
  rela25/1 -> mux27/1
  mux99/1 -> mux101/2, addsub97/1
  logi_b49/1 -> rela100/2, rela99/2
  rela99/1 -> mux101/1
  addsub98/1 -> mux102/3
  mux2/1 -> rela100/1, rela98/1, rela96/1, rela94/1, rela92/1, rela90/1, rela88/1, rela86/1, rela84/1, rela82/1, rela80/1, rela78/1, rela76/1, rela74/1, rela72/1, rela70/1, rela68/1, rela66/1, rela64/1, rela62/1, rela60/1, rela58/1, rela56/1, rela54/1, rela52/1, rela50/1, rela48/1, rela46/1, rela44/1, rela42/1, rela40/1, rela38/1, rela36/1, rela34/1, rela32/1, rela30/1, rela28/1, rela26/1, rela24/1, rela22/1, rela20/1, rela18/1, rela16/1, rela14/1, rela12/1, rela10/1, rela8/1, rela6/1, rela4/1, rela2/1
  rela100/1 -> mux102/1
  Constant7/1 -> addsub20/2, addsub38/2, addsub72/2, addsub90/2, addsub98/2, addsub96/2, addsub94/2, addsub92/2, addsub88/2, addsub86/2, addsub84/2, addsub82/2, addsub80/2, addsub78/2, addsub76/2, addsub74/2, addsub70/2, addsub68/2, addsub66/2, addsub64/2, addsub62/2, addsub60/2, addsub58/2, addsub56/2, addsub54/2, addsub52/2, addsub50/2, addsub48/2, addsub46/2, addsub44/2, addsub42/2, addsub40/2, addsub36/2, addsub34/2, addsub32/2, addsub30/2, addsub28/2, addsub26/2, addsub24/2, addsub22/2, addsub18/2, addsub16/2, addsub14/2, addsub12/2, addsub10/2, addsub8/2, addsub6/2, addsub4/2, addsub2/2, mux4/3
  Constant2/1 -> addsub17/2, addsub19/2, addsub23/2, addsub25/2, addsub27/2, addsub29/2, addsub31/2, addsub37/2, addsub41/2, addsub43/2, addsub45/2, addsub47/2, addsub49/2, addsub53/2, addsub69/2, addsub71/2, addsub75/2, addsub77/2, addsub79/2, addsub81/2, addsub83/2, addsub89/2, addsub93/2, addsub97/2, addsub95/2, addsub91/2, addsub87/2, addsub85/2, addsub73/2, addsub67/2, addsub65/2, addsub63/2, addsub61/2, addsub59/2, addsub57/2, addsub55/2, addsub51/2, addsub39/2, addsub35/2, addsub33/2, addsub21/2, addsub15/2, addsub13/2, addsub11/2, addsub9/2, addsub7/2, addsub5/2, addsub3/2, addsub1/2, mux3/3
  addsub97/1 -> mux101/3
  mux1/1 -> rela99/1, rela97/1, rela95/1, rela93/1, rela91/1, rela89/1, rela87/1, rela85/1, rela83/1, rela81/1, rela79/1, rela77/1, rela75/1, rela73/1, rela71/1, rela69/1, rela67/1, rela65/1, rela63/1, rela61/1, rela59/1, rela57/1, rela55/1, rela53/1, rela51/1, rela49/1, rela47/1, rela45/1, rela43/1, rela41/1, rela39/1, rela37/1, rela35/1, rela33/1, rela31/1, rela29/1, rela27/1, rela25/1, rela23/1, rela21/1, rela19/1, rela17/1, rela15/1, rela13/1, rela11/1, rela9/1, rela7/1, rela5/1, rela3/1, rela1/1
  mux100/1 -> mux102/2, addsub98/1
  addsub18/1 -> mux22/3
  addsub17/1 -> mux21/3
  rela19/1 -> mux21/1
  mux20/1 -> mux22/2, addsub18/1
  mux19/1 -> mux21/2, addsub17/1
  rela20/1 -> mux22/1
  logi_b9/1 -> rela20/2, rela19/2
  addsub36/1 -> mux40/3
  addsub35/1 -> mux39/3
  rela37/1 -> mux39/1
  mux38/1 -> mux40/2, addsub36/1
  mux37/1 -> mux39/2, addsub35/1
  rela38/1 -> mux40/1
  logi_b18/1 -> rela38/2, rela37/2
  mux51/1 -> mux53/2, addsub49/1
  addsub48/1 -> mux52/3
  mux40/1 -> mux42/2, addsub38/1
  addsub49/1 -> mux53/3
  mux54/1 -> mux56/2, addsub52/1
  rela43/1 -> mux45/1
  mux45/1 -> mux47/2, addsub43/1
  addsub52/1 -> mux56/3
  logi_b25/1 -> rela52/2, rela51/2
  rela50/1 -> mux52/1
  mux41/1 -> mux43/2, addsub39/1
  logi_b26/1 -> rela54/2, rela53/2
  addsub40/1 -> mux44/3
  rela48/1 -> mux50/1
  mux55/1 -> mux57/2, addsub53/1
  mux46/1 -> mux48/2, addsub44/1
  rela52/1 -> mux54/1
  addsub54/1 -> mux58/3
  logi_b22/1 -> rela46/2, rela45/2
  addsub53/1 -> mux57/3
  rela54/1 -> mux56/1
  mux56/1 -> mux58/2, addsub54/1
  addsub50/1 -> mux54/3
  rela39/1 -> mux41/1
  mux39/1 -> mux41/2, addsub37/1
  addsub47/1 -> mux51/3
  mux44/1 -> mux46/2, addsub42/1
  logi_b23/1 -> rela48/2, rela47/2
  rela45/1 -> mux47/1
  logi_b24/1 -> rela50/2, rela49/2
  addsub44/1 -> mux48/3
  mux48/1 -> mux50/2, addsub46/1
  addsub39/1 -> mux43/3
  rela55/1 -> mux57/1
  addsub43/1 -> mux47/3
  addsub41/1 -> mux45/3
  rela47/1 -> mux49/1
  addsub38/1 -> mux42/3
  logi_b19/1 -> rela40/2, rela39/2
  addsub37/1 -> mux41/3
  rela42/1 -> mux44/1
  logi_b27/1 -> rela56/2, rela55/2
  mux43/1 -> mux45/2, addsub41/1
  logi_b21/1 -> rela44/2, rela43/2
  rela44/1 -> mux46/1
  addsub42/1 -> mux46/3
  mux53/1 -> mux55/2, addsub51/1
  rela51/1 -> mux53/1
  rela53/1 -> mux55/1
  addsub46/1 -> mux50/3
  mux49/1 -> mux51/2, addsub47/1
  rela46/1 -> mux48/1
  mux50/1 -> mux52/2, addsub48/1
  rela40/1 -> mux42/1
  logi_b20/1 -> rela42/2, rela41/2
  rela49/1 -> mux51/1
  rela41/1 -> mux43/1
  mux52/1 -> mux54/2, addsub50/1
  addsub51/1 -> mux55/3
  mux47/1 -> mux49/2, addsub45/1
  addsub45/1 -> mux49/3
  rela56/1 -> mux58/1
  mux42/1 -> mux44/2, addsub40/1
  addsub59/1 -> mux63/3
  addsub63/1 -> mux67/3
  addsub74/1 -> mux78/3
  addsub96/1 -> mux100/3
  logi_b45/1 -> rela92/2, rela91/2
  rela79/1 -> mux81/1
  rela97/1 -> mux99/1
  mux92/1 -> mux94/2, addsub90/1
  rela60/1 -> mux62/1
  addsub69/1 -> mux73/3
  rela91/1 -> mux93/1
  addsub95/1 -> mux99/3
  addsub62/1 -> mux66/3
  rela96/1 -> mux98/1
  mux98/1 -> mux100/2, addsub96/1
  addsub80/1 -> mux84/3
  addsub93/1 -> mux97/3
  logi_b47/1 -> rela96/2, rela95/2
  logi_b48/1 -> rela98/2, rela97/2
  rela59/1 -> mux61/1
  addsub91/1 -> mux95/3
  mux95/1 -> mux97/2, addsub93/1
  addsub70/1 -> mux74/3
  addsub66/1 -> mux70/3
  rela68/1 -> mux70/1
  rela94/1 -> mux96/1
  rela86/1 -> mux88/1
  logi_b30/1 -> rela62/2, rela61/2
  addsub89/1 -> mux93/3
  addsub57/1 -> mux61/3
  mux96/1 -> mux98/2, addsub94/1
  mux94/1 -> mux96/2, addsub92/1
  mux59/1 -> mux61/2, addsub57/1
  mux91/1 -> mux93/2, addsub89/1
  rela89/1 -> mux91/1
  rela69/1 -> mux71/1
  rela63/1 -> mux65/1
  rela84/1 -> mux86/1
  addsub88/1 -> mux92/3
  mux85/1 -> mux87/2, addsub83/1
  rela95/1 -> mux97/1
  mux82/1 -> mux84/2, addsub80/1
  mux88/1 -> mux90/2, addsub86/1
  rela88/1 -> mux90/1
  rela62/1 -> mux64/1
  logi_b36/1 -> rela74/2, rela73/2
  mux69/1 -> mux71/2, addsub67/1
  addsub90/1 -> mux94/3
  addsub75/1 -> mux79/3
  logi_b40/1 -> rela82/2, rela81/2
  addsub87/1 -> mux91/3
  mux90/1 -> mux92/2, addsub88/1
  logi_b39/1 -> rela80/2, rela79/2
  logi_b41/1 -> rela84/2, rela83/2
  rela70/1 -> mux72/1
  addsub83/1 -> mux87/3
  rela93/1 -> mux95/1
  mux67/1 -> mux69/2, addsub65/1
  addsub58/1 -> mux62/3
  addsub84/1 -> mux88/3
  mux72/1 -> mux74/2, addsub70/1
  addsub55/1 -> mux59/3
  addsub71/1 -> mux75/3
  rela92/1 -> mux94/1
  mux70/1 -> mux72/2, addsub68/1
  mux89/1 -> mux91/2, addsub87/1
  logi_b35/1 -> rela72/2, rela71/2
  addsub56/1 -> mux60/3
  rela81/1 -> mux83/1
  addsub72/1 -> mux76/3
  mux97/1 -> mux99/2, addsub95/1
  rela71/1 -> mux73/1
  rela83/1 -> mux85/1
  rela57/1 -> mux59/1
  rela67/1 -> mux69/1
  addsub92/1 -> mux96/3
  addsub77/1 -> mux81/3
  rela78/1 -> mux80/1
  mux73/1 -> mux75/2, addsub71/1
  rela87/1 -> mux89/1
  rela80/1 -> mux82/1
  mux78/1 -> mux80/2, addsub76/1
  logi_b28/1 -> rela58/2, rela57/2
  logi_b46/1 -> rela94/2, rela93/2
  rela73/1 -> mux75/1
  logi_b42/1 -> rela86/2, rela85/2
  addsub94/1 -> mux98/3
  mux62/1 -> mux64/2, addsub60/1
  addsub67/1 -> mux71/3
  mux71/1 -> mux73/2, addsub69/1
  mux63/1 -> mux65/2, addsub61/1
  addsub61/1 -> mux65/3
  mux87/1 -> mux89/2, addsub85/1
  addsub60/1 -> mux64/3
  logi_b44/1 -> rela90/2, rela89/2
  rela65/1 -> mux67/1
  logi_b32/1 -> rela66/2, rela65/2
  mux93/1 -> mux95/2, addsub91/1
  mux61/1 -> mux63/2, addsub59/1
  logi_b43/1 -> rela88/2, rela87/2
  addsub81/1 -> mux85/3
  mux80/1 -> mux82/2, addsub78/1
  addsub86/1 -> mux90/3
  mux79/1 -> mux81/2, addsub77/1
  rela58/1 -> mux60/1
  rela66/1 -> mux68/1
  mux66/1 -> mux68/2, addsub64/1
  rela98/1 -> mux100/1
  mux81/1 -> mux83/2, addsub79/1
  mux83/1 -> mux85/2, addsub81/1
  addsub68/1 -> mux72/3
  mux68/1 -> mux70/2, addsub66/1
  mux74/1 -> mux76/2, addsub72/1
  mux77/1 -> mux79/2, addsub75/1
  mux75/1 -> mux77/2, addsub73/1
  addsub82/1 -> mux86/3
  addsub73/1 -> mux77/3
  rela77/1 -> mux79/1
  rela76/1 -> mux78/1
  addsub79/1 -> mux83/3
  rela82/1 -> mux84/1
  addsub76/1 -> mux80/3
  mux84/1 -> mux86/2, addsub82/1
  logi_b38/1 -> rela78/2, rela77/2
  rela74/1 -> mux76/1
  logi_b37/1 -> rela76/2, rela75/2
  addsub78/1 -> mux82/3
  rela75/1 -> mux77/1
  rela85/1 -> mux87/1
  mux86/1 -> mux88/2, addsub84/1
  addsub85/1 -> mux89/3
  rela61/1 -> mux63/1
  logi_b34/1 -> rela70/2, rela69/2
  mux64/1 -> mux66/2, addsub62/1
  mux60/1 -> mux62/2, addsub58/1
  logi_b29/1 -> rela60/2, rela59/2
  mux65/1 -> mux67/2, addsub63/1
  mux76/1 -> mux78/2, addsub74/1
  logi_b33/1 -> rela68/2, rela67/2
  rela90/1 -> mux92/1
  mux57/1 -> mux59/2, addsub55/1
  addsub64/1 -> mux68/3
  logi_b31/1 -> rela64/2, rela63/2
  mux58/1 -> mux60/2, addsub56/1
  addsub65/1 -> mux69/3
  rela72/1 -> mux74/1
  rela64/1 -> mux66/1
  mux101/1 -> Slice/1
  mux102/1 -> Slice1/1
  Gate_out1/1 -> Output/1
  Scaling/1 -> Gate_out1/1
  Slice2/1 -> addsub101/2
  ROM20/1 -> Concat/20
  ROM25/1 -> Concat/25
  ROM22/1 -> Concat/22
  ROM32/1 -> Concat/32
  ROM16/1 -> Concat/16
  ROM29/1 -> Concat/29
  ROM24/1 -> Concat/24
  ROM15/1 -> Concat/15
  ROM5/1 -> Concat/5
  ROM23/1 -> Concat/23
  Slice3/1 -> ROM31/1, ROM32/1, ROM30/1, ROM29/1, ROM28/1, ROM27/1, ROM26/1, ROM25/1, ROM24/1, ROM23/1, ROM22/1, ROM21/1, ROM20/1, ROM19/1, ROM18/1, ROM17/1, ROM16/1, ROM15/1, ROM14/1, ROM13/1, ROM12/1, ROM11/1, ROM10/1, ROM9/1, ROM4/1, ROM1/1, ROM2/1, ROM3/1, ROM5/1, ROM6/1, ROM7/1, ROM8/1
  Concat/1 -> Scaling/1
  ROM28/1 -> Concat/28
  ROM9/1 -> Concat/9
  ROM26/1 -> Concat/26
  ROM7/1 -> Concat/7
  ROM14/1 -> Concat/14
  ROM12/1 -> Concat/12
  ROM17/1 -> Concat/17
  ROM6/1 -> Concat/6
  ROM1/1 -> Concat/1
  ROM4/1 -> Concat/4
  ROM27/1 -> Concat/27
  ROM21/1 -> Concat/21
  ROM19/1 -> Concat/19
  ROM3/1 -> Concat/3
  ROM10/1 -> Concat/10
  ROM18/1 -> Concat/18
  ROM11/1 -> Concat/11
  ROM13/1 -> Concat/13
  ROM30/1 -> Concat/30
  ROM2/1 -> Concat/2
  ROM8/1 -> Concat/8
  ROM31/1 -> Concat/31
  Constant5/1 -> addsub103/2
